simulink model "MainPlanevsRainCameras"  (R2020a)
settings: Solver=FixedStepDiscrete  StartTime=0.0  StopTime=20  RelTol=1e-3
model workspace (MAT data in the model file):
  firstWarning = 0
  originalScenarioChecksum = '4AECC2AEC181DD8EA774641D9E64C004'
undefined symbols (not defined in the file): driving
libraries: drivingscenarioandsensors x28
(part 2 of 6)

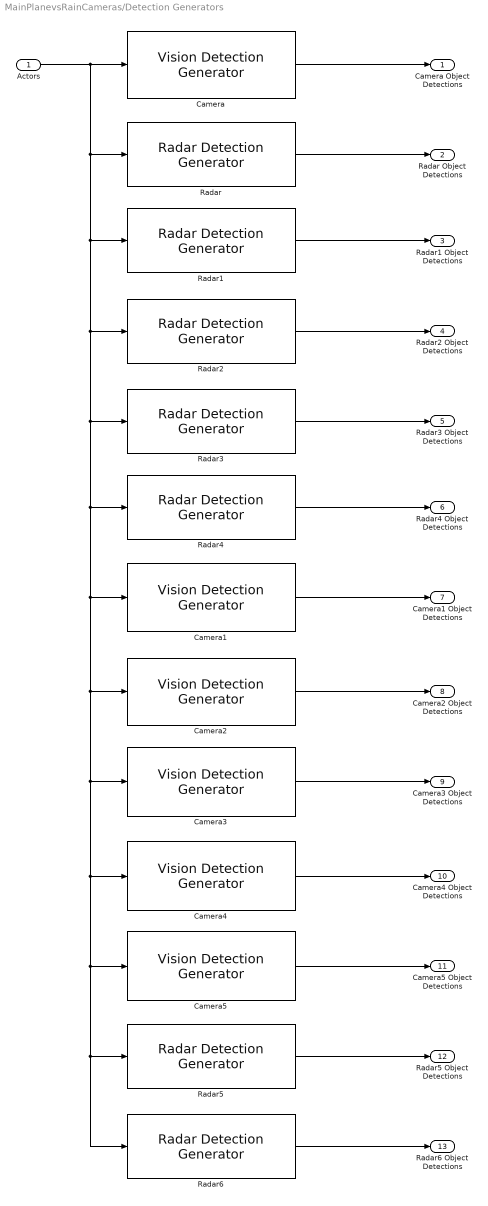
== system MainPlanevsRainCameras/Detection Generators ==
  Actors : Inport
  Camera : drivingscenarioandsensors/Vision Detection Generator  SensorIndex=1  DetectorOutput=Objects only  UpdateInterval=0.1  LaneUpdateInterval=0.1  SensorLocation=[1.9 0]  Height=1.1  Yaw=2.64254529406472  Pitch=1  Roll=0  BusNameSource=Auto  BusName=BusObjectDetections  BusName2Source=Auto  BusName2=BusLaneDetections  MaxNumDetectionsSource=Property  MaxNumDetections=50  MaxNumLanesSource=Property  MaxNumLanes=30  DetectionCoordinates=Ego Cartesian  SimulateUsing=Interpreted execution  MaxRange=11  BoundingBoxAccuracy=5  ProcessNoiseIntensity=5  MaxSpeed=50  MaxAllowedOcclusion=0.5  MinObjectImageSize=[15 15]  DetectionProbability=0.9  FalsePositivesPerImage=0.1  MinLaneImageSize=[20 3]  LaneBoundaryAccuracy=3  HasNoise=on  InitialSeedSource=Repeatable  InitialSeed=0  UsedSeed=0  ActorProfilesSource=MATLAB expression  ActorProfilesParameters=driving.internal.ActorProfilesParameters  ActorProfilesExpression=[struct('ActorID',1,'ClassID',1,'Length',4.7,'Width',1.8,'Height',1.4,'OriginOffset',[-1.35 0 0],'MeshVertices',[3.7 -0.9 1.4;3.7 0.9 1.4;-1 0.9 1.4;-1 -0.9 1.4;3.7 -0.9 0;3.7 0.9 0;-1 0.9 0;-1 -0.9 0],'MeshFaces',[6 2 1;1 5 6;8 4 3;3 7 8;6 7 3;3 2 6;5 1 4;4 8 5;4 1 2;2 3 4;7 6 5;5 8 7],'RCSPattern',[10 10;10 10],'RCSAzimuthAngles',[-180 180],'RCSElevationAngles',[-90 90]); struct('ActorID',2,'ClassID',1,'Length',4.7,'Width',1.8,'Height',1.4,'OriginOffset',[-1.35 0 0],'MeshVertices',[3.7 -0.9 1.4;3.7 0.9 1.4;-1 0.9 1.4;-1 -0.9 1.4;3.7 -0.9 0;3.7 0.9 0;-1 0.9 0;-1 -0.9 0],'MeshFaces',[6 2 1;1 5 6;8 4 3;3 7 8;6 7 3;3 2 6;5 1 4;4 8 5;4 1 2;2 3 4;7 6 5;5 8 7],'RCSPattern',[10 10;10 10],'RCSAzimuthAngles',[-180 180],'RCSElevationAngles',[-90 90]); struct('ActorID',3,'ClassID',1,'Length',4.7,'Width',1.8,'Height',1.4,'OriginOffset',[-1.35 0 0],'MeshVertices',[3.7 -0.9 1.4;3.7 0.9 1.4;-1 0.9 1.4;-1 -0.9 1.4;3.7 -0.9 0;3.7 0.9 0;-1 0.9 0;-1 -0.9 0],'MeshFaces',[6 2 1;1 5 6;8 4 3;3 7 8;6 7 3;3 2 6;5 1 4;4 8 5;4 1 2;2 3 4;7 6 5;5 8 7],'RCSPattern',[10 10;10 10],'RCSAzimuthAngles',[-180 180],'RCSElevationAngles',[-90 90]); struct('ActorID',4,'ClassID',1,'Length',4.7,'Width',1.8,'Height',1.4,'OriginOffset',[-1.35 0 0],'MeshVertices',[3.7 -0.9 1.4;3.7 0.9 1.4;-1 0.9 1.4;-1 -0.9 1.4;3.7 -0.9 0;3.7 0.9 0;-1 0.9 0;-1 -0.9 0],'MeshFaces',[6 2 1;1 5 6;8 4 3;3 7 8;6 7 3;3 2 6;5 1 4;4 8 5;4 1 2;2 3 4;7 6 5;5 8 7],'RCSPattern',[10 10;10 10],'RCSAzimuthAngles',[-180 180],'RCSElevationAngles',[-90 90]); struct('ActorID',5,'ClassID',1,'Length',4.7,'Width',1.8,'Height',1.4,'OriginOffset',[-1.35 0 0],'MeshVertices',[3.7 -0.9 1.4;3.7 0.9 1.4;-1 0.9 1.4;-1 -0.9 1.4;3.7 -0.9 0;3.7 0.9 0;-1 0.9 0;-1 -0.9 0],'MeshFaces',[6 2 1;1 5 6;8 4 3;3 7 8;6 7 3;3 2 6;5 1 4;4 8 5;4 1 2;2 3 4;7 6 5;5 8 7],'RCSPattern',[10 10;10 10],'RCSAzimuthAngles',[-180 180],'RCSElevationAngles',[-90 90]); struct('ActorID',6,'ClassID',4,'Length',0.24,'Width',0.45,'Height',1.7,'OriginOffset',[0 0 0],'MeshVertices',[0.12 -0.225 1.7;0.12 0.225 1.7;-0.12 0.225 1.7;-0.12 -0.225 1.7;0.12 -0.225 -1.11022302462516e-16;0.12 0.225 -1.11022302462516e-16;-0.12 0.225 -1.11022302462516e-16;-0.12 -0.225 -1.11022302462516e-16],'MeshFaces',[6 2 1;1 5 6;8 4 3;3 7 8;6 7 3;3 2 6;5 1 4;4 8 5;4 1 2;2 3 4;7 6 5;5 8 7],'RCSPattern',[-8 -8;-8 -8],'RCSAzimuthAngles',[-180 180],'RCSElevationAngles',[-90 90]); struct('ActorID',7,'ClassID',4,'Length',0.24,'Width',0.45,'Height',1.7,'OriginOffset',[0 0 0],'MeshVertices',[0.12 -0.225 1.7;0.12 0.225 1.7;-0.12 0.225 1.7;-0.12 -0.225 1.7;0.12 -0.225 -1.11022302462516e-16;0.12 0.225 -1.11022302462516e-16;-0.12 0.225 -1.11022302462516e-16;-0.12 -0.225 -1.11022302462516e-16],'MeshFaces',[6 2 1;1 5 6;8 4 3;3 7 8;6 7 3;3 2 6;5 1 4;4 8 5;4 1 2;2 3 4;7 6 5;5 8 7],'RCSPattern',[-8 -8;-8 -8],'RCSAzimuthAngles',[-180 180],'RCSElevationAngles',[-90 90]); struct('ActorID',8,'ClassID',4,'Length',0.24,'Width',0.45,'Height',1.7,'OriginOffset',[0 0 0],'MeshVertices',[0.12 -0.225 1.7;0.12 0.225 1.7;-0.12 0.225 1.7;-0.12 -0.225 1.7;0.12 -0.225 -1.11022302462516e-16;0.12 0.225 -1.11022302462516e-16;-0.12 0.225 -1.11022302462516e-16;-0.12 -0.225 -1.11022302462516e-16],'MeshFaces',[6 2 1;1 5 6;8 4 3;3 7 8;6 7 3;3 2 6;5 1 4;4 8 5;4 1 2;2 3 4;7 6 5;5 8 7],'RCSPattern',[-8 -8;-8 -8],'RCSAzimuthAngles',[-180 180],'RCSElevationAngles',[-90 90]); struct('ActorID',9,'ClassID',4,'Length',0.24,'Width',0.45,'Height',1.7,'OriginOffset',[0 0 0],'MeshVertices',[0.12 -0.225 1.7;0.12 0.225 1.7;-0.12 0.225 1.7;-0.12 -0.225 1.7;0.12 -0.225 -1.11022302462516e-16;0.12 0.225 -1.11022302462516e-16;-0.12 0.225 -1.11022302462516e-16;-0.12 -0.225 -1.11022302462516e-16],'MeshFaces',[6 2 1;1 5 6;8 4 3;3 7 8;6 7 3;3 2 6;5 1 4;4 8 5;4 1 2;2 3 4;7 6 5;5 8 7],'RCSPattern',[-8 -8;-8 -8],'RCSAzimuthAngles',[-180 180],'RCSElevationAngles',[-90 90]); struct('ActorID',10,'ClassID',4,'Length',0.24,'Width',0.45,'Height',1.7,'OriginOffset',[0 0 0],'MeshVertices',[0.12 -0.225 1.7;0.12 0.225 1.7;-0.12 0.225 1.7;-0.12 -0.225 1.7;0.12 -0.225 -1.11022302462516e-16;0.12 0.225 -1.11022302462516e-16;-0.12 0.225 -1.11022302462516e-16;-0.12 -0.225 -1.11022302462516e-16],'MeshFaces',[6 2 1;1 5 6;8 4 3;3 7 8;6 7 3;3 2 6;5 1 4;4 8 5;4 1 2;2 3 4;7 6 5;5 8 7],'RCSPattern',[-8 -8;-8 -8],'RCSAzimuthAngles',[-180 180],'RCSElevationAngles',[-90 90]); struct('ActorID',11,'ClassID',4,'Length',0.24,'Width',0.45,'Height',1.7,'OriginOffset',[0 0 0],'MeshVertices',[0.12 -0.225 1.7;0.12 0.225 1.7;-0.12 0.225 1.7;-0.12 -0.225 1.7;0.12 -0.225 -1.11022302462516e-16;0.12 0.225 -1.11022302462516e-16;-0.12 0.225 -1.11022302462516e-16;-0.12 -0.225 -1.11022302462516e-16],'MeshFaces',[6 2 1;1 5 6;8 4 3;3 7 8;6 7 3;3 2 6;5 1 4;4 8 5;4 1 2;2 3 4;7 6 5;5 8 7],'RCSPattern',[-8 -8;-8 -8],'RCSAzimuthAngles',[-180 180],'RCSElevationAngles',[-90 90]); struct('ActorID',12,'ClassID',4,'Length',0.24,'Width',0.45,'Height',1.7,'OriginOffset',[0 0 0],'MeshVertices',[0.12 -0.225 1.7;0.12 0.225 1.7;-0.12 0.225 1.7;-0.12 -0.225 1.7;0.12 -0.225 -1.11022302462516e-16;0.12 0.225 -1.11022302462516e-16;-0.12 0.225 -1.11022302462516e-16;-0.12 -0.225 -1.11022302462516e-16],'MeshFaces',[6 2 1;1 5 6;8 4 3;3 7 8;6 7 3;3 2 6;5 1 4;4 8 5;4 1 2;2 3 4;7 6 5;5 8 7],'RCSPattern',[-8 -8;-8 -8],'RCSAzimuthAngles',[-180 180],'RCSElevationAngles',[-90 90]); struct('ActorID',13,'ClassID',4,'Length',0.24,'Width',0.45,'Height',1.7,'OriginOffset',[0 0 0],'MeshVertices',[0.12 -0.225 1.7;0.12 0.225 1.7;-0.12 0.225 1.7;-0.12 -0.225 1.7;0.12 -0.225 -1.11022302462516e-16;0.12 0.225 -1.11022302462516e-16;-0.12 0.225 -1.11022302462516e-16;-0.12 -0.225 -1.11022302462516e-16],'MeshFaces',[6 2 1;1 5 6;8 4 3;3 7 8;6 7 3;3 2 6;5 1 4;4 8 5;4 1 2;2 3 4;7 6 5;5 8 7],'RCSPattern',[-8 -8;-8 -8],'RCSAzimuthAngles',[-180 180],'RCSElevationAngles',[-90 90]); struct('ActorID',14,'ClassID',4,'Length',0.24,'Width',0.45,'Height',1.7,'OriginOffset',[0 0 0],'MeshVertices',[0.12 -0.225 1.7;0.12 0.225 1.7;-0.12 0.225 1.7;-0.12 -0.225 1.7;0.12 -0.225 -1.11022302462516e-16;0.12 0.225 -1.11022302462516e-16;-0.12 0.225 -1.11022302462516e-16;-0.12 -0.225 -1.11022302462516e-16],'MeshFaces',[6 2 1;1 5 6;8 4 3;3 7 8;6 7 3;3 2 6;5 1 4;4 8 5;4 1 2;2 3 4;7 6 5;5 8 7],'RCSPattern',[-8 -8;-8 -8],'RCSAzimuthAngles',[-180 180],'RCSElevationAngles',[-90 90]); struct('ActorID',15,'ClassID',4,'Length',0.24,'Width',0.45,'Height',1.7,'OriginOffset',[0 0 0],'MeshVertices',[0.12 -0.225 1.7;0.12 0.225 1.7;-0.12 0.225 1.7;-0.12 -0.225 1.7;0.12 -0.225 -1.11022302462516e-16;0.12 0.225 -1.11022302462516e-16;-0.12 0.225 -1.11022302462516e-16;-0.12 -0.225 -1.11022302462516e-16],'MeshFaces',[6 2 1;1 5 6;8 4 3;3 7 8;6 7 3;3 2 6;5 1 4;4 8 5;4 1 2;2 3 4;7 6 5;5 8 7],'RCSPattern',[-8 -8;-8 -8],'RCSAzimuthAngles',[-180 180],'RCSElevationAngles',[-90 90]); struct('ActorID',16,'ClassID',4,'Length',0.24,'Width',0.45,'Height',1.7,'OriginOffset',[0 0 0],'MeshVertices',[0.12 -0.225 1.7;0.12 0.225 1.7;-0.12 0.225 1.7;-0.12 -0.225 1.7;0.12 -0.225 -1.11022302462516e-16;0.12 0.225 -1.11022302462516e-16;-0.12 0.225 -1.11022302462516e-16;-0.12 -0.225 -1.11022302462516e-16],'MeshFaces',[6 2 1;1 5 6;8 4 3;3 7 8;6 7 3;3 2 6;5 1 4;4 8 5;4 1 2;2 3 4;7 6 5;5 8 7],'RCSPattern',[-8 -8;-8 -8],'RCSAzimuthAngles',[-180 180],'RCSElevationAngles',[-90 90]); struct('ActorID',17,'ClassID',4,'Length',0.24,'Width',0.45,'Height',1.7,'OriginOffset',[0 0 0],'MeshVertices',[0.12 -0.225 1.7;0.12 0.225 1.7;-0.12 0.225 1.7;-0.12 -0.225 1.7;0.12 -0.225 -1.11022302462516e-16;0.12 0.225 -1.11022302462516e-16;-0.12 0.225 -1.11022302462516e-16;-0.12 -0.225 -1.11022302462516e-16],'MeshFaces',[6 2 1;1 5 6;8 4 3;3 7 8;6 7 3;3 2 6;5 1 4;4 8 5;4 1 2;2 3 4;7 6 5;5 8 7],'RCSPattern',[-8 -8;-8 -8],'RCSAzimuthAngles',[-180 180],'RCSElevationAngles',[-90 90]); struct('ActorID',18,'ClassID',4,'Length',0.24,'Width',0.45,'Height',1.7,'OriginOffset',[0 0 0],'MeshVertices',[0.12 -0.225 1.7;0.12 0.225 1.7;-0.12 0.225 1.7;-0.12 -0.225 1.7;0.12 -0.225 -1.11022302462516e-16;0.12 0.225 -1.11022302462516e-16;-0.12 0.225 -1.11022302462516e-16;-0.12 -0.225 -1.11022302462516e-16],'MeshFaces',[6 2 1;1 5 6;8 4 3;3 7 8;6 7 3;3 2 6;5 1 4;4 8 5;4 1 2;2 3 4;7 6 5;5 8 7],'RCSPattern',[-8 -8;-8 -8],'RCSAzimuthAngles',[-180 180],'RCSElevationAngles',[-90 90]); struct('ActorID',19,'ClassID',4,'Length',0.24,'Width',0.45,'Height',1.7,'OriginOffset',[0 0 0],'MeshVertices',[0.12 -0.225 1.7;0.12 0.225 1.7;-0.12 0.225 1.7;-0.12 -0.225 1.7;0.12 -0.225 -1.11022302462516e-16;0.12 0.225 -1.11022302462516e-16;-0.12 0.225 -1.11022302462516e-16;-0.12 -0.225 -1.11022302462516e-16],'MeshFaces',[6 2 1;1 5 6;8 4 3;3 7 8;6 7 3;3 2 6;5 1 4;4 8 5;4 1 2;2 3 4;7 6 5;5 8 7],'RCSPattern',[-8 -8;-8 -8],'RCSAzimuthAngles',[-180 180],'RCSElevationAngles',[-90 90]); struct('ActorID',20,'ClassID',4,'Length',0.24,'Width',0.45,'Height',1.7,'OriginOffset',[0 0 0],'MeshVertices',[0.12 -0.225 1.7;0.12 0.225 1.7;-0.12 0.225 1.7;-0.12 -0.225 1.7;0.12 -0.225 -1.11022302462516e-16;0.12 0.225 -1.11022302462516e-16;-0.12 0.225 -1.11022302462516e-16;-0.12 -0.225 -1.11022302462516e-16],'MeshFaces',[6 2 1;1 5 6;8 4 3;3 7 8;6 7 3;3 2 6;5 1 4;4 8 5;4 1 2;2 3 4;7 6 5;5 8 7],'RCSPattern',[-8 -8;-8 -8],'RCSAzimuthAngles',[-180 180],'RCSElevationAngles',[-90 90]); struct('ActorID',21,'ClassID',4,'Length',0.24,'Width',0.45,'Height',1.7,'OriginOffset',[0 0 0],'MeshVertices',[0.12 -0.225 1.7;0.12 0.225 1.7;-0.12 0.225 1.7;-0.12 -0.225 1.7;0.12 -0.225 -1.11022302462516e-16;0.12 0.225 -1.11022302462516e-16;-0.12 0.225 -1.11022302462516e-16;-0.12 -0.225 -1.11022302462516e-16],'MeshFaces',[6 2 1;1 5 6;8 4 3;3 7 8;6 7 3;3 2 6;5 1 4;4 8 5;4 1 2;2 3 4;7 6 5;5 8 7],'RCSPattern',[-8 -8;-8 -8],'RCSAzimuthAngles',[-180 180],'RCSElevationAngles',[-90 90]); struct('ActorID',22,'ClassID',4,'Length',0.24,'Width',0.45,'Height',1.7,'OriginOffset',[0 0 0],'MeshVertices',[0.12 -0.225 1.7;0.12 0.225 1.7;-0.12 0.225 1.7;-0.12 -0.225 1.7;0.12 -0.225 -1.11022302462516e-16;0.12 0.225 -1.11022302462516e-16;-0.12 0.225 -1.11022302462516e-16;-0.12 -0.225 -1.11022302462516e-16],'MeshFaces',[6 2 1;1 5 6;8 4 3;3 7 8;6 7 3;3 2 6;5 1 4;4 8 5;4 1 2;2 3 4;7 6 5;5 8 7],'RCSPattern',[-8 -8;-8 -8],'RCSAzimuthAngles',[-180 180],'RCSElevationAngles',[-90 90]); struct('ActorID',23,'ClassID',4,'Length',0.24,'Width',0.45,'Height',1.7,'OriginOffset',[0 0 0],'MeshVertices',[0.12 -0.225 1.7;0.12 0.225 1.7;-0.12 0.225 1.7;-0.12 -0.225 1.7;0.12 -0.225 -1.11022302462516e-16;0.12 0.225 -1.11022302462516e-16;-0.12 0.225 -1.11022302462516e-16;-0.12 -0.225 -1.11022302462516e-16],'MeshFaces',[6 2 1;1 5 6;8 4 3;3 7 8;6 7 3;3 2 6;5 1 4;4 8 5;4 1 2;2 3 4;7 6 5;5 8 7],'RCSPattern',[-8 -8;-8 -8],'RCSAzimuthAngles',[-180 180],'RCSElevationAngles',[-90 90]); struct('ActorID',24,'ClassID',4,'Length',0.24,'Width',0.45,'Height',1.7,'OriginOffset',[0 0 0],'MeshVertices',[0.12 -0.225 1.7;0.12 0.225 1.7;-0.12 0.225 1.7;-0.12 -0.225 1.7;0.12 -0.225 -1.11022302462516e-16;0.12 0.225 -1.11022302462516e-16;-0.12 0.225 -1.11022302462516e-16;-0.12 -0.225 -1.11022302462516e-16],'MeshFaces',[6 2 1;1 5 6;8 4 3;3 7 8;6 7 3;3 2 6;5 1 4;4 8 5;4 1 2;2 3 4;7 6 5;5 8 7],'RCSPattern',[-8 -8;-8 -8],'RCSAzimuthAngles',[-180 180],'RCSElevationAngles',[-90 90]); struct('ActorID',25,'ClassID',4,'Length',0.24,'Width',0.45,'Height',1.7,'OriginOffset',[0 0 0],'MeshVertices',[0.12 -0.225 1.7;0.12 0.225 1.7;-0.12 0.225 1.7;-0.12 -0.225 1.7;0.12 -0.225 -1.11022302462516e-16;0.12 0.225 -1.11022302462516e-16;-0.12 0.225 -1.11022302462516e-16;-0.12 -0.225 -1.11022302462516e-16],'MeshFaces',[6 2 1;1 5 6;8 4 3;3 7 8;6 7 3;3 2 6;5 1 4;4 8 5;4 1 2;2 3 4;7 6 5;5 8 7],'RCSPattern',[-8 -8;-8 -8],'RCSAzimuthAngles',[-180 180],'RCSElevationAngles',[-90 90]); struct('ActorID',26,'ClassID',4,'Length',0.24,'Width',0.45,'Height',1.7,'OriginOffset',[0 0 0],'MeshVertices',[0.12 -0.225 1.7;0.12 0.225 1.7;-0.12 0.225 1.7;-0.12 -0.225 1.7;0.12 -0.225 -1.11022302462516e-16;0.12 0.225 -1.11022302462516e-16;-0.12 0.225 -1.11022302462516e-16;-0.12 -0.225 -1.11022302462516e-16],'MeshFaces',[6 2 1;1 5 6;8 4 3;3 7 8;6 7 3;3 2 6;5 1 4;4 8 5;4 1 2;2 3 4;7 6 5;5 8 7],'RCSPattern',[-8 -8;-8 -8],'RCSAzimuthAngles',[-180 180],'RCSElevationAngles',[-90 90]); struct('ActorID',27,'ClassID',4,'Length',0.24,'Width',0.45,'Height',1.7,'OriginOffset',[0 0 0],'MeshVertices',[0.12 -0.225 1.7;0.12 0.225 1.7;-0.12 0.225 1.7;-0.12 -0.225 1.7;0.12 -0.225 -1.11022302462516e-16;0.12 0.225 -1.11022302462516e-16;-0.12 0.225 -1.11022302462516e-16;-0.12 -0.225 -1.11022302462516e-16],'MeshFaces',[6 2 1;1 5 6;8 4 3;3 7 8;6 7 3;3 2 6;5 1 4;4 8 5;4 1 2;2 3 4;7 6 5;5 8 7],'RCSPattern',[-8 -8;-8 -8],'RCSAzimuthAngles',[-180 180],'RCSElevationAngles',[-90 90]); struct('ActorID',28,'ClassID',3,'Length',1.7,'Width',0.45,'Height',1.7,'OriginOffset',[0 0 0],'MeshVertices',[0.85 -0.225 1.7;0.85 0.225 1.7;-0.85 0.225 1.7;-0.85 -0.225 1.7;0.85 -0.225 -1.11022302462516e-16;0.85 0.225 -1.11022302462516e-16;-0.85 0.225 -1.11022302462516e-16;-0.85 -0.225 -1.11022302462516e-16],'MeshFaces',[6 2 1;1 5 6;8 4 3;3 7 8;6 7 3;3 2 6;5 1 4;4 8 5;4 1 2;2 3 4;7 6 5;5 8 7],'RCSPattern',[10 10;10 10],'RCSAzimuthAngles',[-180 180],'RCSElevationAngles',[-90 90]); struct('ActorID',29,'ClassID',4,'Length',0.24,'Width',0.45,'Height',1.7,'OriginOffset',[0 0 0],'MeshVertices',[0.12 -0.225 1.7;0.12 0.225 1.7;-0.12 0.225 1.7;-0.12 -0.225 1.7;0.12 -0.225 -1.11022302462516e-16;0.12 0.225 -1.11022302462516e-16;-0.12 0.225 -1.11022302462516e-16;-0.12 -0.225 -1.11022302462516e-16],'MeshFaces',[6 2 1;1 5 6;8 4 3;3 7 8;6 7 3;3 2 6;5 1 4;4 8 5;4 1 2;2 3 4;7 6 5;5 8 7],'RCSPattern',[-8 -8;-8 -8],'RCSAzimuthAngles',[-180 180],'RCSElevationAngles',[-90 90])]  Intrinsics=driving.internal.cameraIntrinsics('FocalLength',[800 799.999999999999],'PrincipalPoint',[320 240],'ImageSize',[480 640],'RadialDistortion',[0 0],'TangentialDistortion',[0 0],'Skew',0)
  Camera1 : drivingscenarioandsensors/Vision Detection Generator  SensorIndex=7  DetectorOutput=Objects only  UpdateInterval=0.1  LaneUpdateInterval=0.1  SensorLocation=[0 0.9]  Height=1.1  Yaw=90  Pitch=1  Roll=0  BusNameSource=Auto  BusName=BusObjectDetections  BusName2Source=Auto  BusName2=BusLaneDetections  MaxNumDetectionsSource=Property  MaxNumDetections=50  MaxNumLanesSource=Property  MaxNumLanes=30  DetectionCoordinates=Ego Cartesian  SimulateUsing=Interpreted execution  MaxRange=10  BoundingBoxAccuracy=5  ProcessNoiseIntensity=5  MaxSpeed=50  MaxAllowedOcclusion=0.5  MinObjectImageSize=[15 15]  DetectionProbability=0.2  FalsePositivesPerImage=0.1  MinLaneImageSize=[20 3]  LaneBoundaryAccuracy=3  HasNoise=on  InitialSeedSource=Repeatable  InitialSeed=0  UsedSeed=0  ActorProfilesSource=MATLAB expression  ActorProfilesParameters=driving.internal.ActorProfilesParameters  ActorProfilesExpression=[struct('ActorID',1,'ClassID',1,'Length',4.7,'Width',1.8,'Height',1.4,'OriginOffset',[-1.35 0 0],'MeshVertices',[3.7 -0.9 1.4;3.7 0.9 1.4;-1 0.9 1.4;-1 -0.9 1.4;3.7 -0.9 0;3.7 0.9 0;-1 0.9 0;-1 -0.9 0],'MeshFaces',[6 2 1;1 5 6;8 4 3;3 7 8;6 7 3;3 2 6;5 1 4;4 8 5;4 1 2;2 3 4;7 6 5;5 8 7],'RCSPattern',[10 10;10 10],'RCSAzimuthAngles',[-180 180],'RCSElevationAngles',[-90 90]); struct('ActorID',2,'ClassID',1,'Length',4.7,'Width',1.8,'Height',1.4,'OriginOffset',[-1.35 0 0],'MeshVertices',[3.7 -0.9 1.4;3.7 0.9 1.4;-1 0.9 1.4;-1 -0.9 1.4;3.7 -0.9 0;3.7 0.9 0;-1 0.9 0;-1 -0.9 0],'MeshFaces',[6 2 1;1 5 6;8 4 3;3 7 8;6 7 3;3 2 6;5 1 4;4 8 5;4 1 2;2 3 4;7 6 5;5 8 7],'RCSPattern',[10 10;10 10],'RCSAzimuthAngles',[-180 180],'RCSElevationAngles',[-90 90]); struct('ActorID',3,'ClassID',1,'Length',4.7,'Width',1.8,'Height',1.4,'OriginOffset',[-1.35 0 0],'MeshVertices',[3.7 -0.9 1.4;3.7 0.9 1.4;-1 0.9 1.4;-1 -0.9 1.4;3.7 -0.9 0;3.7 0.9 0;-1 0.9 0;-1 -0.9 0],'MeshFaces',[6 2 1;1 5 6;8 4 3;3 7 8;6 7 3;3 2 6;5 1 4;4 8 5;4 1 2;2 3 4;7 6 5;5 8 7],'RCSPattern',[10 10;10 10],'RCSAzimuthAngles',[-180 180],'RCSElevationAngles',[-90 90]); struct('ActorID',4,'ClassID',1,'Length',4.7,'Width',1.8,'Height',1.4,'OriginOffset',[-1.35 0 0],'MeshVertices',[3.7 -0.9 1.4;3.7 0.9 1.4;-1 0.9 1.4;-1 -0.9 1.4;3.7 -0.9 0;3.7 0.9 0;-1 0.9 0;-1 -0.9 0],'MeshFaces',[6 2 1;1 5 6;8 4 3;3 7 8;6 7 3;3 2 6;5 1 4;4 8 5;4 1 2;2 3 4;7 6 5;5 8 7],'RCSPattern',[10 10;10 10],'RCSAzimuthAngles',[-180 180],'RCSElevationAngles',[-90 90]); struct('ActorID',5,'ClassID',1,'Length',4.7,'Width',1.8,'Height',1.4,'OriginOffset',[-1.35 0 0],'MeshVertices',[3.7 -0.9 1.4;3.7 0.9 1.4;-1 0.9 1.4;-1 -0.9 1.4;3.7 -0.9 0;3.7 0.9 0;-1 0.9 0;-1 -0.9 0],'MeshFaces',[6 2 1;1 5 6;8 4 3;3 7 8;6 7 3;3 2 6;5 1 4;4 8 5;4 1 2;2 3 4;7 6 5;5 8 7],'RCSPattern',[10 10;10 10],'RCSAzimuthAngles',[-180 180],'RCSElevationAngles',[-90 90]); struct('ActorID',6,'ClassID',4,'Length',0.24,'Width',0.45,'Height',1.7,'OriginOffset',[0 0 0],'MeshVertices',[0.12 -0.225 1.7;0.12 0.225 1.7;-0.12 0.225 1.7;-0.12 -0.225 1.7;0.12 -0.225 -1.11022302462516e-16;0.12 0.225 -1.11022302462516e-16;-0.12 0.225 -1.11022302462516e-16;-0.12 -0.225 -1.11022302462516e-16],'MeshFaces',[6 2 1;1 5 6;8 4 3;3 7 8;6 7 3;3 2 6;5 1 4;4 8 5;4 1 2;2 3 4;7 6 5;5 8 7],'RCSPattern',[-8 -8;-8 -8],'RCSAzimuthAngles',[-180 180],'RCSElevationAngles',[-90 90]); struct('ActorID',7,'ClassID',4,'Length',0.24,'Width',0.45,'Height',1.7,'OriginOffset',[0 0 0],'MeshVertices',[0.12 -0.225 1.7;0.12 0.225 1.7;-0.12 0.225 1.7;-0.12 -0.225 1.7;0.12 -0.225 -1.11022302462516e-16;0.12 0.225 -1.11022302462516e-16;-0.12 0.225 -1.11022302462516e-16;-0.12 -0.225 -1.11022302462516e-16],'MeshFaces',[6 2 1;1 5 6;8 4 3;3 7 8;6 7 3;3 2 6;5 1 4;4 8 5;4 1 2;2 3 4;7 6 5;5 8 7],'RCSPattern',[-8 -8;-8 -8],'RCSAzimuthAngles',[-180 180],'RCSElevationAngles',[-90 90]); struct('ActorID',8,'ClassID',4,'Length',0.24,'Width',0.45,'Height',1.7,'OriginOffset',[0 0 0],'MeshVertices',[0.12 -0.225 1.7;0.12 0.225 1.7;-0.12 0.225 1.7;-0.12 -0.225 1.7;0.12 -0.225 -1.11022302462516e-16;0.12 0.225 -1.11022302462516e-16;-0.12 0.225 -1.11022302462516e-16;-0.12 -0.225 -1.11022302462516e-16],'MeshFaces',[6 2 1;1 5 6;8 4 3;3 7 8;6 7 3;3 2 6;5 1 4;4 8 5;4 1 2;2 3 4;7 6 5;5 8 7],'RCSPattern',[-8 -8;-8 -8],'RCSAzimuthAngles',[-180 180],'RCSElevationAngles',[-90 90]); struct('ActorID',9,'ClassID',4,'Length',0.24,'Width',0.45,'Height',1.7,'OriginOffset',[0 0 0],'MeshVertices',[0.12 -0.225 1.7;0.12 0.225 1.7;-0.12 0.225 1.7;-0.12 -0.225 1.7;0.12 -0.225 -1.11022302462516e-16;0.12 0.225 -1.11022302462516e-16;-0.12 0.225 -1.11022302462516e-16;-0.12 -0.225 -1.11022302462516e-16],'MeshFaces',[6 2 1;1 5 6;8 4 3;3 7 8;6 7 3;3 2 6;5 1 4;4 8 5;4 1 2;2 3 4;7 6 5;5 8 7],'RCSPattern',[-8 -8;-8 -8],'RCSAzimuthAngles',[-180 180],'RCSElevationAngles',[-90 90]); struct('ActorID',10,'ClassID',4,'Length',0.24,'Width',0.45,'Height',1.7,'OriginOffset',[0 0 0],'MeshVertices',[0.12 -0.225 1.7;0.12 0.225 1.7;-0.12 0.225 1.7;-0.12 -0.225 1.7;0.12 -0.225 -1.11022302462516e-16;0.12 0.225 -1.11022302462516e-16;-0.12 0.225 -1.11022302462516e-16;-0.12 -0.225 -1.11022302462516e-16],'MeshFaces',[6 2 1;1 5 6;8 4 3;3 7 8;6 7 3;3 2 6;5 1 4;4 8 5;4 1 2;2 3 4;7 6 5;5 8 7],'RCSPattern',[-8 -8;-8 -8],'RCSAzimuthAngles',[-180 180],'RCSElevationAngles',[-90 90]); struct('ActorID',11,'ClassID',4,'Length',0.24,'Width',0.45,'Height',1.7,'OriginOffset',[0 0 0],'MeshVertices',[0.12 -0.225 1.7;0.12 0.225 1.7;-0.12 0.225 1.7;-0.12 -0.225 1.7;0.12 -0.225 -1.11022302462516e-16;0.12 0.225 -1.11022302462516e-16;-0.12 0.225 -1.11022302462516e-16;-0.12 -0.225 -1.11022302462516e-16],'MeshFaces',[6 2 1;1 5 6;8 4 3;3 7 8;6 7 3;3 2 6;5 1 4;4 8 5;4 1 2;2 3 4;7 6 5;5 8 7],'RCSPattern',[-8 -8;-8 -8],'RCSAzimuthAngles',[-180 180],'RCSElevationAngles',[-90 90]); struct('ActorID',12,'ClassID',4,'Length',0.24,'Width',0.45,'Height',1.7,'OriginOffset',[0 0 0],'MeshVertices',[0.12 -0.225 1.7;0.12 0.225 1.7;-0.12 0.225 1.7;-0.12 -0.225 1.7;0.12 -0.225 -1.11022302462516e-16;0.12 0.225 -1.11022302462516e-16;-0.12 0.225 -1.11022302462516e-16;-0.12 -0.225 -1.11022302462516e-16],'MeshFaces',[6 2 1;1 5 6;8 4 3;3 7 8;6 7 3;3 2 6;5 1 4;4 8 5;4 1 2;2 3 4;7 6 5;5 8 7],'RCSPattern',[-8 -8;-8 -8],'RCSAzimuthAngles',[-180 180],'RCSElevationAngles',[-90 90]); struct('ActorID',13,'ClassID',4,'Length',0.24,'Width',0.45,'Height',1.7,'OriginOffset',[0 0 0],'MeshVertices',[0.12 -0.225 1.7;0.12 0.225 1.7;-0.12 0.225 1.7;-0.12 -0.225 1.7;0.12 -0.225 -1.11022302462516e-16;0.12 0.225 -1.11022302462516e-16;-0.12 0.225 -1.11022302462516e-16;-0.12 -0.225 -1.11022302462516e-16],'MeshFaces',[6 2 1;1 5 6;8 4 3;3 7 8;6 7 3;3 2 6;5 1 4;4 8 5;4 1 2;2 3 4;7 6 5;5 8 7],'RCSPattern',[-8 -8;-8 -8],'RCSAzimuthAngles',[-180 180],'RCSElevationAngles',[-90 90]); struct('ActorID',14,'ClassID',4,'Length',0.24,'Width',0.45,'Height',1.7,'OriginOffset',[0 0 0],'MeshVertices',[0.12 -0.225 1.7;0.12 0.225 1.7;-0.12 0.225 1.7;-0.12 -0.225 1.7;0.12 -0.225 -1.11022302462516e-16;0.12 0.225 -1.11022302462516e-16;-0.12 0.225 -1.11022302462516e-16;-0.12 -0.225 -1.11022302462516e-16],'MeshFaces',[6 2 1;1 5 6;8 4 3;3 7 8;6 7 3;3 2 6;5 1 4;4 8 5;4 1 2;2 3 4;7 6 5;5 8 7],'RCSPattern',[-8 -8;-8 -8],'RCSAzimuthAngles',[-180 180],'RCSElevationAngles',[-90 90]); struct('ActorID',15,'ClassID',4,'Length',0.24,'Width',0.45,'Height',1.7,'OriginOffset',[0 0 0],'MeshVertices',[0.12 -0.225 1.7;0.12 0.225 1.7;-0.12 0.225 1.7;-0.12 -0.225 1.7;0.12 -0.225 -1.11022302462516e-16;0.12 0.225 -1.11022302462516e-16;-0.12 0.225 -1.11022302462516e-16;-0.12 -0.225 -1.11022302462516e-16],'MeshFaces',[6 2 1;1 5 6;8 4 3;3 7 8;6 7 3;3 2 6;5 1 4;4 8 5;4 1 2;2 3 4;7 6 5;5 8 7],'RCSPattern',[-8 -8;-8 -8],'RCSAzimuthAngles',[-180 180],'RCSElevationAngles',[-90 90]); struct('ActorID',16,'ClassID',4,'Length',0.24,'Width',0.45,'Height',1.7,'OriginOffset',[0 0 0],'MeshVertices',[0.12 -0.225 1.7;0.12 0.225 1.7;-0.12 0.225 1.7;-0.12 -0.225 1.7;0.12 -0.225 -1.11022302462516e-16;0.12 0.225 -1.11022302462516e-16;-0.12 0.225 -1.11022302462516e-16;-0.12 -0.225 -1.11022302462516e-16],'MeshFaces',[6 2 1;1 5 6;8 4 3;3 7 8;6 7 3;3 2 6;5 1 4;4 8 5;4 1 2;2 3 4;7 6 5;5 8 7],'RCSPattern',[-8 -8;-8 -8],'RCSAzimuthAngles',[-180 180],'RCSElevationAngles',[-90 90]); struct('ActorID',17,'ClassID',4,'Length',0.24,'Width',0.45,'Height',1.7,'OriginOffset',[0 0 0],'MeshVertices',[0.12 -0.225 1.7;0.12 0.225 1.7;-0.12 0.225 1.7;-0.12 -0.225 1.7;0.12 -0.225 -1.11022302462516e-16;0.12 0.225 -1.11022302462516e-16;-0.12 0.225 -1.11022302462516e-16;-0.12 -0.225 -1.11022302462516e-16],'MeshFaces',[6 2 1;1 5 6;8 4 3;3 7 8;6 7 3;3 2 6;5 1 4;4 8 5;4 1 2;2 3 4;7 6 5;5 8 7],'RCSPattern',[-8 -8;-8 -8],'RCSAzimuthAngles',[-180 180],'RCSElevationAngles',[-90 90]); struct('ActorID',18,'ClassID',4,'Length',0.24,'Width',0.45,'Height',1.7,'OriginOffset',[0 0 0],'MeshVertices',[0.12 -0.225 1.7;0.12 0.225 1.7;-0.12 0.225 1.7;-0.12 -0.225 1.7;0.12 -0.225 -1.11022302462516e-16;0.12 0.225 -1.11022302462516e-16;-0.12 0.225 -1.11022302462516e-16;-0.12 -0.225 -1.11022302462516e-16],'MeshFaces',[6 2 1;1 5 6;8 4 3;3 7 8;6 7 3;3 2 6;5 1 4;4 8 5;4 1 2;2 3 4;7 6 5;5 8 7],'RCSPattern',[-8 -8;-8 -8],'RCSAzimuthAngles',[-180 180],'RCSElevationAngles',[-90 90]); struct('ActorID',19,'ClassID',4,'Length',0.24,'Width',0.45,'Height',1.7,'OriginOffset',[0 0 0],'MeshVertices',[0.12 -0.225 1.7;0.12 0.225 1.7;-0.12 0.225 1.7;-0.12 -0.225 1.7;0.12 -0.225 -1.11022302462516e-16;0.12 0.225 -1.11022302462516e-16;-0.12 0.225 -1.11022302462516e-16;-0.12 -0.225 -1.11022302462516e-16],'MeshFaces',[6 2 1;1 5 6;8 4 3;3 7 8;6 7 3;3 2 6;5 1 4;4 8 5;4 1 2;2 3 4;7 6 5;5 8 7],'RCSPattern',[-8 -8;-8 -8],'RCSAzimuthAngles',[-180 180],'RCSElevationAngles',[-90 90]); struct('ActorID',20,'ClassID',4,'Length',0.24,'Width',0.45,'Height',1.7,'OriginOffset',[0 0 0],'MeshVertices',[0.12 -0.225 1.7;0.12 0.225 1.7;-0.12 0.225 1.7;-0.12 -0.225 1.7;0.12 -0.225 -1.11022302462516e-16;0.12 0.225 -1.11022302462516e-16;-0.12 0.225 -1.11022302462516e-16;-0.12 -0.225 -1.11022302462516e-16],'MeshFaces',[6 2 1;1 5 6;8 4 3;3 7 8;6 7 3;3 2 6;5 1 4;4 8 5;4 1 2;2 3 4;7 6 5;5 8 7],'RCSPattern',[-8 -8;-8 -8],'RCSAzimuthAngles',[-180 180],'RCSElevationAngles',[-90 90]); struct('ActorID',21,'ClassID',4,'Length',0.24,'Width',0.45,'Height',1.7,'OriginOffset',[0 0 0],'MeshVertices',[0.12 -0.225 1.7;0.12 0.225 1.7;-0.12 0.225 1.7;-0.12 -0.225 1.7;0.12 -0.225 -1.11022302462516e-16;0.12 0.225 -1.11022302462516e-16;-0.12 0.225 -1.11022302462516e-16;-0.12 -0.225 -1.11022302462516e-16],'MeshFaces',[6 2 1;1 5 6;8 4 3;3 7 8;6 7 3;3 2 6;5 1 4;4 8 5;4 1 2;2 3 4;7 6 5;5 8 7],'RCSPattern',[-8 -8;-8 -8],'RCSAzimuthAngles',[-180 180],'RCSElevationAngles',[-90 90]); struct('ActorID',22,'ClassID',4,'Length',0.24,'Width',0.45,'Height',1.7,'OriginOffset',[0 0 0],'MeshVertices',[0.12 -0.225 1.7;0.12 0.225 1.7;-0.12 0.225 1.7;-0.12 -0.225 1.7;0.12 -0.225 -1.11022302462516e-16;0.12 0.225 -1.11022302462516e-16;-0.12 0.225 -1.11022302462516e-16;-0.12 -0.225 -1.11022302462516e-16],'MeshFaces',[6 2 1;1 5 6;8 4 3;3 7 8;6 7 3;3 2 6;5 1 4;4 8 5;4 1 2;2 3 4;7 6 5;5 8 7],'RCSPattern',[-8 -8;-8 -8],'RCSAzimuthAngles',[-180 180],'RCSElevationAngles',[-90 90]); struct('ActorID',23,'ClassID',4,'Length',0.24,'Width',0.45,'Height',1.7,'OriginOffset',[0 0 0],'MeshVertices',[0.12 -0.225 1.7;0.12 0.225 1.7;-0.12 0.225 1.7;-0.12 -0.225 1.7;0.12 -0.225 -1.11022302462516e-16;0.12 0.225 -1.11022302462516e-16;-0.12 0.225 -1.11022302462516e-16;-0.12 -0.225 -1.11022302462516e-16],'MeshFaces',[6 2 1;1 5 6;8 4 3;3 7 8;6 7 3;3 2 6;5 1 4;4 8 5;4 1 2;2 3 4;7 6 5;5 8 7],'RCSPattern',[-8 -8;-8 -8],'RCSAzimuthAngles',[-180 180],'RCSElevationAngles',[-90 90]); struct('ActorID',24,'ClassID',4,'Length',0.24,'Width',0.45,'Height',1.7,'OriginOffset',[0 0 0],'MeshVertices',[0.12 -0.225 1.7;0.12 0.225 1.7;-0.12 0.225 1.7;-0.12 -0.225 1.7;0.12 -0.225 -1.11022302462516e-16;0.12 0.225 -1.11022302462516e-16;-0.12 0.225 -1.11022302462516e-16;-0.12 -0.225 -1.11022302462516e-16],'MeshFaces',[6 2 1;1 5 6;8 4 3;3 7 8;6 7 3;3 2 6;5 1 4;4 8 5;4 1 2;2 3 4;7 6 5;5 8 7],'RCSPattern',[-8 -8;-8 -8],'RCSAzimuthAngles',[-180 180],'RCSElevationAngles',[-90 90]); struct('ActorID',25,'ClassID',4,'Length',0.24,'Width',0.45,'Height',1.7,'OriginOffset',[0 0 0],'MeshVertices',[0.12 -0.225 1.7;0.12 0.225 1.7;-0.12 0.225 1.7;-0.12 -0.225 1.7;0.12 -0.225 -1.11022302462516e-16;0.12 0.225 -1.11022302462516e-16;-0.12 0.225 -1.11022302462516e-16;-0.12 -0.225 -1.11022302462516e-16],'MeshFaces',[6 2 1;1 5 6;8 4 3;3 7 8;6 7 3;3 2 6;5 1 4;4 8 5;4 1 2;2 3 4;7 6 5;5 8 7],'RCSPattern',[-8 -8;-8 -8],'RCSAzimuthAngles',[-180 180],'RCSElevationAngles',[-90 90]); struct('ActorID',26,'ClassID',4,'Length',0.24,'Width',0.45,'Height',1.7,'OriginOffset',[0 0 0],'MeshVertices',[0.12 -0.225 1.7;0.12 0.225 1.7;-0.12 0.225 1.7;-0.12 -0.225 1.7;0.12 -0.225 -1.11022302462516e-16;0.12 0.225 -1.11022302462516e-16;-0.12 0.225 -1.11022302462516e-16;-0.12 -0.225 -1.11022302462516e-16],'MeshFaces',[6 2 1;1 5 6;8 4 3;3 7 8;6 7 3;3 2 6;5 1 4;4 8 5;4 1 2;2 3 4;7 6 5;5 8 7],'RCSPattern',[-8 -8;-8 -8],'RCSAzimuthAngles',[-180 180],'RCSElevationAngles',[-90 90]); struct('ActorID',27,'ClassID',4,'Length',0.24,'Width',0.45,'Height',1.7,'OriginOffset',[0 0 0],'MeshVertices',[0.12 -0.225 1.7;0.12 0.225 1.7;-0.12 0.225 1.7;-0.12 -0.225 1.7;0.12 -0.225 -1.11022302462516e-16;0.12 0.225 -1.11022302462516e-16;-0.12 0.225 -1.11022302462516e-16;-0.12 -0.225 -1.11022302462516e-16],'MeshFaces',[6 2 1;1 5 6;8 4 3;3 7 8;6 7 3;3 2 6;5 1 4;4 8 5;4 1 2;2 3 4;7 6 5;5 8 7],'RCSPattern',[-8 -8;-8 -8],'RCSAzimuthAngles',[-180 180],'RCSElevationAngles',[-90 90]); struct('ActorID',28,'ClassID',3,'Length',1.7,'Width',0.45,'Height',1.7,'OriginOffset',[0 0 0],'MeshVertices',[0.85 -0.225 1.7;0.85 0.225 1.7;-0.85 0.225 1.7;-0.85 -0.225 1.7;0.85 -0.225 -1.11022302462516e-16;0.85 0.225 -1.11022302462516e-16;-0.85 0.225 -1.11022302462516e-16;-0.85 -0.225 -1.11022302462516e-16],'MeshFaces',[6 2 1;1 5 6;8 4 3;3 7 8;6 7 3;3 2 6;5 1 4;4 8 5;4 1 2;2 3 4;7 6 5;5 8 7],'RCSPattern',[10 10;10 10],'RCSAzimuthAngles',[-180 180],'RCSElevationAngles',[-90 90]); struct('ActorID',29,'ClassID',4,'Length',0.24,'Width',0.45,'Height',1.7,'OriginOffset',[0 0 0],'MeshVertices',[0.12 -0.225 1.7;0.12 0.225 1.7;-0.12 0.225 1.7;-0.12 -0.225 1.7;0.12 -0.225 -1.11022302462516e-16;0.12 0.225 -1.11022302462516e-16;-0.12 0.225 -1.11022302462516e-16;-0.12 -0.225 -1.11022302462516e-16],'MeshFaces',[6 2 1;1 5 6;8 4 3;3 7 8;6 7 3;3 2 6;5 1 4;4 8 5;4 1 2;2 3 4;7 6 5;5 8 7],'RCSPattern',[-8 -8;-8 -8],'RCSAzimuthAngles',[-180 180],'RCSElevationAngles',[-90 90])]  Intrinsics=driving.internal.cameraIntrinsics('FocalLength',[320 320],'PrincipalPoint',[320 240],'ImageSize',[480 640],'RadialDistortion',[0 0],'TangentialDistortion',[0 0],'Skew',0)
  Camera2 : drivingscenarioandsensors/Vision Detection Generator  SensorIndex=8  DetectorOutput=Objects only  UpdateInterval=0.1  LaneUpdateInterval=0.1  SensorLocation=[0 -0.9]  Height=1.1  Yaw=-90  Pitch=1  Roll=0  BusNameSource=Auto  BusName=BusObjectDetections  BusName2Source=Auto  BusName2=BusLaneDetections  MaxNumDetectionsSource=Property  MaxNumDetections=50  MaxNumLanesSource=Property  MaxNumLanes=30  DetectionCoordinates=Ego Cartesian  SimulateUsing=Interpreted execution  MaxRange=10  BoundingBoxAccuracy=5  ProcessNoiseIntensity=2  MaxSpeed=50  MaxAllowedOcclusion=0.5  MinObjectImageSize=[15 15]  DetectionProbability=0.2  FalsePositivesPerImage=0.1  MinLaneImageSize=[20 3]  LaneBoundaryAccuracy=3  HasNoise=on  InitialSeedSource=Repeatable  InitialSeed=0  UsedSeed=0  ActorProfilesSource=MATLAB expression  ActorProfilesParameters=driving.internal.ActorProfilesParameters  ActorProfilesExpression=[struct('ActorID',1,'ClassID',1,'Length',4.7,'Width',1.8,'Height',1.4,'OriginOffset',[-1.35 0 0],'MeshVertices',[3.7 -0.9 1.4;3.7 0.9 1.4;-1 0.9 1.4;-1 -0.9 1.4;3.7 -0.9 0;3.7 0.9 0;-1 0.9 0;-1 -0.9 0],'MeshFaces',[6 2 1;1 5 6;8 4 3;3 7 8;6 7 3;3 2 6;5 1 4;4 8 5;4 1 2;2 3 4;7 6 5;5 8 7],'RCSPattern',[10 10;10 10],'RCSAzimuthAngles',[-180 180],'RCSElevationAngles',[-90 90]); struct('ActorID',2,'ClassID',1,'Length',4.7,'Width',1.8,'Height',1.4,'OriginOffset',[-1.35 0 0],'MeshVertices',[3.7 -0.9 1.4;3.7 0.9 1.4;-1 0.9 1.4;-1 -0.9 1.4;3.7 -0.9 0;3.7 0.9 0;-1 0.9 0;-1 -0.9 0],'MeshFaces',[6 2 1;1 5 6;8 4 3;3 7 8;6 7 3;3 2 6;5 1 4;4 8 5;4 1 2;2 3 4;7 6 5;5 8 7],'RCSPattern',[10 10;10 10],'RCSAzimuthAngles',[-180 180],'RCSElevationAngles',[-90 90]); struct('ActorID',3,'ClassID',1,'Length',4.7,'Width',1.8,'Height',1.4,'OriginOffset',[-1.35 0 0],'MeshVertices',[3.7 -0.9 1.4;3.7 0.9 1.4;-1 0.9 1.4;-1 -0.9 1.4;3.7 -0.9 0;3.7 0.9 0;-1 0.9 0;-1 -0.9 0],'MeshFaces',[6 2 1;1 5 6;8 4 3;3 7 8;6 7 3;3 2 6;5 1 4;4 8 5;4 1 2;2 3 4;7 6 5;5 8 7],'RCSPattern',[10 10;10 10],'RCSAzimuthAngles',[-180 180],'RCSElevationAngles',[-90 90]); struct('ActorID',4,'ClassID',1,'Length',4.7,'Width',1.8,'Height',1.4,'OriginOffset',[-1.35 0 0],'MeshVertices',[3.7 -0.9 1.4;3.7 0.9 1.4;-1 0.9 1.4;-1 -0.9 1.4;3.7 -0.9 0;3.7 0.9 0;-1 0.9 0;-1 -0.9 0],'MeshFaces',[6 2 1;1 5 6;8 4 3;3 7 8;6 7 3;3 2 6;5 1 4;4 8 5;4 1 2;2 3 4;7 6 5;5 8 7],'RCSPattern',[10 10;10 10],'RCSAzimuthAngles',[-180 180],'RCSElevationAngles',[-90 90]); struct('ActorID',5,'ClassID',1,'Length',4.7,'Width',1.8,'Height',1.4,'OriginOffset',[-1.35 0 0],'MeshVertices',[3.7 -0.9 1.4;3.7 0.9 1.4;-1 0.9 1.4;-1 -0.9 1.4;3.7 -0.9 0;3.7 0.9 0;-1 0.9 0;-1 -0.9 0],'MeshFaces',[6 2 1;1 5 6;8 4 3;3 7 8;6 7 3;3 2 6;5 1 4;4 8 5;4 1 2;2 3 4;7 6 5;5 8 7],'RCSPattern',[10 10;10 10],'RCSAzimuthAngles',[-180 180],'RCSElevationAngles',[-90 90]); struct('ActorID',6,'ClassID',4,'Length',0.24,'Width',0.45,'Height',1.7,'OriginOffset',[0 0 0],'MeshVertices',[0.12 -0.225 1.7;0.12 0.225 1.7;-0.12 0.225 1.7;-0.12 -0.225 1.7;0.12 -0.225 -1.11022302462516e-16;0.12 0.225 -1.11022302462516e-16;-0.12 0.225 -1.11022302462516e-16;-0.12 -0.225 -1.11022302462516e-16],'MeshFaces',[6 2 1;1 5 6;8 4 3;3 7 8;6 7 3;3 2 6;5 1 4;4 8 5;4 1 2;2 3 4;7 6 5;5 8 7],'RCSPattern',[-8 -8;-8 -8],'RCSAzimuthAngles',[-180 180],'RCSElevationAngles',[-90 90]); struct('ActorID',7,'ClassID',4,'Length',0.24,'Width',0.45,'Height',1.7,'OriginOffset',[0 0 0],'MeshVertices',[0.12 -0.225 1.7;0.12 0.225 1.7;-0.12 0.225 1.7;-0.12 -0.225 1.7;0.12 -0.225 -1.11022302462516e-16;0.12 0.225 -1.11022302462516e-16;-0.12 0.225 -1.11022302462516e-16;-0.12 -0.225 -1.11022302462516e-16],'MeshFaces',[6 2 1;1 5 6;8 4 3;3 7 8;6 7 3;3 2 6;5 1 4;4 8 5;4 1 2;2 3 4;7 6 5;5 8 7],'RCSPattern',[-8 -8;-8 -8],'RCSAzimuthAngles',[-180 180],'RCSElevationAngles',[-90 90]); struct('ActorID',8,'ClassID',4,'Length',0.24,'Width',0.45,'Height',1.7,'OriginOffset',[0 0 0],'MeshVertices',[0.12 -0.225 1.7;0.12 0.225 1.7;-0.12 0.225 1.7;-0.12 -0.225 1.7;0.12 -0.225 -1.11022302462516e-16;0.12 0.225 -1.11022302462516e-16;-0.12 0.225 -1.11022302462516e-16;-0.12 -0.225 -1.11022302462516e-16],'MeshFaces',[6 2 1;1 5 6;8 4 3;3 7 8;6 7 3;3 2 6;5 1 4;4 8 5;4 1 2;2 3 4;7 6 5;5 8 7],'RCSPattern',[-8 -8;-8 -8],'RCSAzimuthAngles',[-180 180],'RCSElevationAngles',[-90 90]); struct('ActorID',9,'ClassID',4,'Length',0.24,'Width',0.45,'Height',1.7,'OriginOffset',[0 0 0],'MeshVertices',[0.12 -0.225 1.7;0.12 0.225 1.7;-0.12 0.225 1.7;-0.12 -0.225 1.7;0.12 -0.225 -1.11022302462516e-16;0.12 0.225 -1.11022302462516e-16;-0.12 0.225 -1.11022302462516e-16;-0.12 -0.225 -1.11022302462516e-16],'MeshFaces',[6 2 1;1 5 6;8 4 3;3 7 8;6 7 3;3 2 6;5 1 4;4 8 5;4 1 2;2 3 4;7 6 5;5 8 7],'RCSPattern',[-8 -8;-8 -8],'RCSAzimuthAngles',[-180 180],'RCSElevationAngles',[-90 90]); struct('ActorID',10,'ClassID',4,'Length',0.24,'Width',0.45,'Height',1.7,'OriginOffset',[0 0 0],'MeshVertices',[0.12 -0.225 1.7;0.12 0.225 1.7;-0.12 0.225 1.7;-0.12 -0.225 1.7;0.12 -0.225 -1.11022302462516e-16;0.12 0.225 -1.11022302462516e-16;-0.12 0.225 -1.11022302462516e-16;-0.12 -0.225 -1.11022302462516e-16],'MeshFaces',[6 2 1;1 5 6;8 4 3;3 7 8;6 7 3;3 2 6;5 1 4;4 8 5;4 1 2;2 3 4;7 6 5;5 8 7],'RCSPattern',[-8 -8;-8 -8],'RCSAzimuthAngles',[-180 180],'RCSElevationAngles',[-90 90]); struct('ActorID',11,'ClassID',4,'Length',0.24,'Width',0.45,'Height',1.7,'OriginOffset',[0 0 0],'MeshVertices',[0.12 -0.225 1.7;0.12 0.225 1.7;-0.12 0.225 1.7;-0.12 -0.225 1.7;0.12 -0.225 -1.11022302462516e-16;0.12 0.225 -1.11022302462516e-16;-0.12 0.225 -1.11022302462516e-16;-0.12 -0.225 -1.11022302462516e-16],'MeshFaces',[6 2 1;1 5 6;8 4 3;3 7 8;6 7 3;3 2 6;5 1 4;4 8 5;4 1 2;2 3 4;7 6 5;5 8 7],'RCSPattern',[-8 -8;-8 -8],'RCSAzimuthAngles',[-180 180],'RCSElevationAngles',[-90 90]); struct('ActorID',12,'ClassID',4,'Length',0.24,'Width',0.45,'Height',1.7,'OriginOffset',[0 0 0],'MeshVertices',[0.12 -0.225 1.7;0.12 0.225 1.7;-0.12 0.225 1.7;-0.12 -0.225 1.7;0.12 -0.225 -1.11022302462516e-16;0.12 0.225 -1.11022302462516e-16;-0.12 0.225 -1.11022302462516e-16;-0.12 -0.225 -1.11022302462516e-16],'MeshFaces',[6 2 1;1 5 6;8 4 3;3 7 8;6 7 3;3 2 6;5 1 4;4 8 5;4 1 2;2 3 4;7 6 5;5 8 7],'RCSPattern',[-8 -8;-8 -8],'RCSAzimuthAngles',[-180 180],'RCSElevationAngles',[-90 90]); struct('ActorID',13,'ClassID',4,'Length',0.24,'Width',0.45,'Height',1.7,'OriginOffset',[0 0 0],'MeshVertices',[0.12 -0.225 1.7;0.12 0.225 1.7;-0.12 0.225 1.7;-0.12 -0.225 1.7;0.12 -0.225 -1.11022302462516e-16;0.12 0.225 -1.11022302462516e-16;-0.12 0.225 -1.11022302462516e-16;-0.12 -0.225 -1.11022302462516e-16],'MeshFaces',[6 2 1;1 5 6;8 4 3;3 7 8;6 7 3;3 2 6;5 1 4;4 8 5;4 1 2;2 3 4;7 6 5;5 8 7],'RCSPattern',[-8 -8;-8 -8],'RCSAzimuthAngles',[-180 180],'RCSElevationAngles',[-90 90]); struct('ActorID',14,'ClassID',4,'Length',0.24,'Width',0.45,'Height',1.7,'OriginOffset',[0 0 0],'MeshVertices',[0.12 -0.225 1.7;0.12 0.225 1.7;-0.12 0.225 1.7;-0.12 -0.225 1.7;0.12 -0.225 -1.11022302462516e-16;0.12 0.225 -1.11022302462516e-16;-0.12 0.225 -1.11022302462516e-16;-0.12 -0.225 -1.11022302462516e-16],'MeshFaces',[6 2 1;1 5 6;8 4 3;3 7 8;6 7 3;3 2 6;5 1 4;4 8 5;4 1 2;2 3 4;7 6 5;5 8 7],'RCSPattern',[-8 -8;-8 -8],'RCSAzimuthAngles',[-180 180],'RCSElevationAngles',[-90 90]); struct('ActorID',15,'ClassID',4,'Length',0.24,'Width',0.45,'Height',1.7,'OriginOffset',[0 0 0],'MeshVertices',[0.12 -0.225 1.7;0.12 0.225 1.7;-0.12 0.225 1.7;-0.12 -0.225 1.7;0.12 -0.225 -1.11022302462516e-16;0.12 0.225 -1.11022302462516e-16;-0.12 0.225 -1.11022302462516e-16;-0.12 -0.225 -1.11022302462516e-16],'MeshFaces',[6 2 1;1 5 6;8 4 3;3 7 8;6 7 3;3 2 6;5 1 4;4 8 5;4 1 2;2 3 4;7 6 5;5 8 7],'RCSPattern',[-8 -8;-8 -8],'RCSAzimuthAngles',[-180 180],'RCSElevationAngles',[-90 90]); struct('ActorID',16,'ClassID',4,'Length',0.24,'Width',0.45,'Height',1.7,'OriginOffset',[0 0 0],'MeshVertices',[0.12 -0.225 1.7;0.12 0.225 1.7;-0.12 0.225 1.7;-0.12 -0.225 1.7;0.12 -0.225 -1.11022302462516e-16;0.12 0.225 -1.11022302462516e-16;-0.12 0.225 -1.11022302462516e-16;-0.12 -0.225 -1.11022302462516e-16],'MeshFaces',[6 2 1;1 5 6;8 4 3;3 7 8;6 7 3;3 2 6;5 1 4;4 8 5;4 1 2;2 3 4;7 6 5;5 8 7],'RCSPattern',[-8 -8;-8 -8],'RCSAzimuthAngles',[-180 180],'RCSElevationAngles',[-90 90]); struct('ActorID',17,'ClassID',4,'Length',0.24,'Width',0.45,'Height',1.7,'OriginOffset',[0 0 0],'MeshVertices',[0.12 -0.225 1.7;0.12 0.225 1.7;-0.12 0.225 1.7;-0.12 -0.225 1.7;0.12 -0.225 -1.11022302462516e-16;0.12 0.225 -1.11022302462516e-16;-0.12 0.225 -1.11022302462516e-16;-0.12 -0.225 -1.11022302462516e-16],'MeshFaces',[6 2 1;1 5 6;8 4 3;3 7 8;6 7 3;3 2 6;5 1 4;4 8 5;4 1 2;2 3 4;7 6 5;5 8 7],'RCSPattern',[-8 -8;-8 -8],'RCSAzimuthAngles',[-180 180],'RCSElevationAngles',[-90 90]); struct('ActorID',18,'ClassID',4,'Length',0.24,'Width',0.45,'Height',1.7,'OriginOffset',[0 0 0],'MeshVertices',[0.12 -0.225 1.7;0.12 0.225 1.7;-0.12 0.225 1.7;-0.12 -0.225 1.7;0.12 -0.225 -1.11022302462516e-16;0.12 0.225 -1.11022302462516e-16;-0.12 0.225 -1.11022302462516e-16;-0.12 -0.225 -1.11022302462516e-16],'MeshFaces',[6 2 1;1 5 6;8 4 3;3 7 8;6 7 3;3 2 6;5 1 4;4 8 5;4 1 2;2 3 4;7 6 5;5 8 7],'RCSPattern',[-8 -8;-8 -8],'RCSAzimuthAngles',[-180 180],'RCSElevationAngles',[-90 90]); struct('ActorID',19,'ClassID',4,'Length',0.24,'Width',0.45,'Height',1.7,'OriginOffset',[0 0 0],'MeshVertices',[0.12 -0.225 1.7;0.12 0.225 1.7;-0.12 0.225 1.7;-0.12 -0.225 1.7;0.12 -0.225 -1.11022302462516e-16;0.12 0.225 -1.11022302462516e-16;-0.12 0.225 -1.11022302462516e-16;-0.12 -0.225 -1.11022302462516e-16],'MeshFaces',[6 2 1;1 5 6;8 4 3;3 7 8;6 7 3;3 2 6;5 1 4;4 8 5;4 1 2;2 3 4;7 6 5;5 8 7],'RCSPattern',[-8 -8;-8 -8],'RCSAzimuthAngles',[-180 180],'RCSElevationAngles',[-90 90]); struct('ActorID',20,'ClassID',4,'Length',0.24,'Width',0.45,'Height',1.7,'OriginOffset',[0 0 0],'MeshVertices',[0.12 -0.225 1.7;0.12 0.225 1.7;-0.12 0.225 1.7;-0.12 -0.225 1.7;0.12 -0.225 -1.11022302462516e-16;0.12 0.225 -1.11022302462516e-16;-0.12 0.225 -1.11022302462516e-16;-0.12 -0.225 -1.11022302462516e-16],'MeshFaces',[6 2 1;1 5 6;8 4 3;3 7 8;6 7 3;3 2 6;5 1 4;4 8 5;4 1 2;2 3 4;7 6 5;5 8 7],'RCSPattern',[-8 -8;-8 -8],'RCSAzimuthAngles',[-180 180],'RCSElevationAngles',[-90 90]); struct('ActorID',21,'ClassID',4,'Length',0.24,'Width',0.45,'Height',1.7,'OriginOffset',[0 0 0],'MeshVertices',[0.12 -0.225 1.7;0.12 0.225 1.7;-0.12 0.225 1.7;-0.12 -0.225 1.7;0.12 -0.225 -1.11022302462516e-16;0.12 0.225 -1.11022302462516e-16;-0.12 0.225 -1.11022302462516e-16;-0.12 -0.225 -1.11022302462516e-16],'MeshFaces',[6 2 1;1 5 6;8 4 3;3 7 8;6 7 3;3 2 6;5 1 4;4 8 5;4 1 2;2 3 4;7 6 5;5 8 7],'RCSPattern',[-8 -8;-8 -8],'RCSAzimuthAngles',[-180 180],'RCSElevationAngles',[-90 90]); struct('ActorID',22,'ClassID',4,'Length',0.24,'Width',0.45,'Height',1.7,'OriginOffset',[0 0 0],'MeshVertices',[0.12 -0.225 1.7;0.12 0.225 1.7;-0.12 0.225 1.7;-0.12 -0.225 1.7;0.12 -0.225 -1.11022302462516e-16;0.12 0.225 -1.11022302462516e-16;-0.12 0.225 -1.11022302462516e-16;-0.12 -0.225 -1.11022302462516e-16],'MeshFaces',[6 2 1;1 5 6;8 4 3;3 7 8;6 7 3;3 2 6;5 1 4;4 8 5;4 1 2;2 3 4;7 6 5;5 8 7],'RCSPattern',[-8 -8;-8 -8],'RCSAzimuthAngles',[-180 180],'RCSElevationAngles',[-90 90]); struct('ActorID',23,'ClassID',4,'Length',0.24,'Width',0.45,'Height',1.7,'OriginOffset',[0 0 0],'MeshVertices',[0.12 -0.225 1.7;0.12 0.225 1.7;-0.12 0.225 1.7;-0.12 -0.225 1.7;0.12 -0.225 -1.11022302462516e-16;0.12 0.225 -1.11022302462516e-16;-0.12 0.225 -1.11022302462516e-16;-0.12 -0.225 -1.11022302462516e-16],'MeshFaces',[6 2 1;1 5 6;8 4 3;3 7 8;6 7 3;3 2 6;5 1 4;4 8 5;4 1 2;2 3 4;7 6 5;5 8 7],'RCSPattern',[-8 -8;-8 -8],'RCSAzimuthAngles',[-180 180],'RCSElevationAngles',[-90 90]); struct('ActorID',24,'ClassID',4,'Length',0.24,'Width',0.45,'Height',1.7,'OriginOffset',[0 0 0],'MeshVertices',[0.12 -0.225 1.7;0.12 0.225 1.7;-0.12 0.225 1.7;-0.12 -0.225 1.7;0.12 -0.225 -1.11022302462516e-16;0.12 0.225 -1.11022302462516e-16;-0.12 0.225 -1.11022302462516e-16;-0.12 -0.225 -1.11022302462516e-16],'MeshFaces',[6 2 1;1 5 6;8 4 3;3 7 8;6 7 3;3 2 6;5 1 4;4 8 5;4 1 2;2 3 4;7 6 5;5 8 7],'RCSPattern',[-8 -8;-8 -8],'RCSAzimuthAngles',[-180 180],'RCSElevationAngles',[-90 90]); struct('ActorID',25,'ClassID',4,'Length',0.24,'Width',0.45,'Height',1.7,'OriginOffset',[0 0 0],'MeshVertices',[0.12 -0.225 1.7;0.12 0.225 1.7;-0.12 0.225 1.7;-0.12 -0.225 1.7;0.12 -0.225 -1.11022302462516e-16;0.12 0.225 -1.11022302462516e-16;-0.12 0.225 -1.11022302462516e-16;-0.12 -0.225 -1.11022302462516e-16],'MeshFaces',[6 2 1;1 5 6;8 4 3;3 7 8;6 7 3;3 2 6;5 1 4;4 8 5;4 1 2;2 3 4;7 6 5;5 8 7],'RCSPattern',[-8 -8;-8 -8],'RCSAzimuthAngles',[-180 180],'RCSElevationAngles',[-90 90]); struct('ActorID',26,'ClassID',4,'Length',0.24,'Width',0.45,'Height',1.7,'OriginOffset',[0 0 0],'MeshVertices',[0.12 -0.225 1.7;0.12 0.225 1.7;-0.12 0.225 1.7;-0.12 -0.225 1.7;0.12 -0.225 -1.11022302462516e-16;0.12 0.225 -1.11022302462516e-16;-0.12 0.225 -1.11022302462516e-16;-0.12 -0.225 -1.11022302462516e-16],'MeshFaces',[6 2 1;1 5 6;8 4 3;3 7 8;6 7 3;3 2 6;5 1 4;4 8 5;4 1 2;2 3 4;7 6 5;5 8 7],'RCSPattern',[-8 -8;-8 -8],'RCSAzimuthAngles',[-180 180],'RCSElevationAngles',[-90 90]); struct('ActorID',27,'ClassID',4,'Length',0.24,'Width',0.45,'Height',1.7,'OriginOffset',[0 0 0],'MeshVertices',[0.12 -0.225 1.7;0.12 0.225 1.7;-0.12 0.225 1.7;-0.12 -0.225 1.7;0.12 -0.225 -1.11022302462516e-16;0.12 0.225 -1.11022302462516e-16;-0.12 0.225 -1.11022302462516e-16;-0.12 -0.225 -1.11022302462516e-16],'MeshFaces',[6 2 1;1 5 6;8 4 3;3 7 8;6 7 3;3 2 6;5 1 4;4 8 5;4 1 2;2 3 4;7 6 5;5 8 7],'RCSPattern',[-8 -8;-8 -8],'RCSAzimuthAngles',[-180 180],'RCSElevationAngles',[-90 90]); struct('ActorID',28,'ClassID',3,'Length',1.7,'Width',0.45,'Height',1.7,'OriginOffset',[0 0 0],'MeshVertices',[0.85 -0.225 1.7;0.85 0.225 1.7;-0.85 0.225 1.7;-0.85 -0.225 1.7;0.85 -0.225 -1.11022302462516e-16;0.85 0.225 -1.11022302462516e-16;-0.85 0.225 -1.11022302462516e-16;-0.85 -0.225 -1.11022302462516e-16],'MeshFaces',[6 2 1;1 5 6;8 4 3;3 7 8;6 7 3;3 2 6;5 1 4;4 8 5;4 1 2;2 3 4;7 6 5;5 8 7],'RCSPattern',[10 10;10 10],'RCSAzimuthAngles',[-180 180],'RCSElevationAngles',[-90 90]); struct('ActorID',29,'ClassID',4,'Length',0.24,'Width',0.45,'Height',1.7,'OriginOffset',[0 0 0],'MeshVertices',[0.12 -0.225 1.7;0.12 0.225 1.7;-0.12 0.225 1.7;-0.12 -0.225 1.7;0.12 -0.225 -1.11022302462516e-16;0.12 0.225 -1.11022302462516e-16;-0.12 0.225 -1.11022302462516e-16;-0.12 -0.225 -1.11022302462516e-16],'MeshFaces',[6 2 1;1 5 6;8 4 3;3 7 8;6 7 3;3 2 6;5 1 4;4 8 5;4 1 2;2 3 4;7 6 5;5 8 7],'RCSPattern',[-8 -8;-8 -8],'RCSAzimuthAngles',[-180 180],'RCSElevationAngles',[-90 90])]  Intrinsics=driving.internal.cameraIntrinsics('FocalLength',[320 320],'PrincipalPoint',[320 240],'ImageSize',[480 640],'RadialDistortion',[0 0],'TangentialDistortion',[0 0],'Skew',0)
  Camera3 : drivingscenarioandsensors/Vision Detection Generator  SensorIndex=9  DetectorOutput=Objects only  UpdateInterval=0.1  LaneUpdateInterval=0.1  SensorLocation=[3.7 0]  Height=1.1  Yaw=64.0691935373481  Pitch=1  Roll=0  BusNameSource=Auto  BusName=BusObjectDetections  BusName2Source=Auto  BusName2=BusLaneDetections  MaxNumDetectionsSource=Property  MaxNumDetections=50  MaxNumLanesSource=Property  MaxNumLanes=30  DetectionCoordinates=Ego Cartesian  SimulateUsing=Interpreted execution  MaxRange=10  BoundingBoxAccuracy=5  ProcessNoiseIntensity=5  MaxSpeed=50  MaxAllowedOcclusion=0.5  MinObjectImageSize=[15 15]  DetectionProbability=0.2  FalsePositivesPerImage=0.1  MinLaneImageSize=[20 3]  LaneBoundaryAccuracy=3  HasNoise=on  InitialSeedSource=Repeatable  InitialSeed=0  UsedSeed=0  ActorProfilesSource=MATLAB expression  ActorProfilesParameters=driving.internal.ActorProfilesParameters  ActorProfilesExpression=[struct('ActorID',1,'ClassID',1,'Length',4.7,'Width',1.8,'Height',1.4,'OriginOffset',[-1.35 0 0],'MeshVertices',[3.7 -0.9 1.4;3.7 0.9 1.4;-1 0.9 1.4;-1 -0.9 1.4;3.7 -0.9 0;3.7 0.9 0;-1 0.9 0;-1 -0.9 0],'MeshFaces',[6 2 1;1 5 6;8 4 3;3 7 8;6 7 3;3 2 6;5 1 4;4 8 5;4 1 2;2 3 4;7 6 5;5 8 7],'RCSPattern',[10 10;10 10],'RCSAzimuthAngles',[-180 180],'RCSElevationAngles',[-90 90]); struct('ActorID',2,'ClassID',1,'Length',4.7,'Width',1.8,'Height',1.4,'OriginOffset',[-1.35 0 0],'MeshVertices',[3.7 -0.9 1.4;3.7 0.9 1.4;-1 0.9 1.4;-1 -0.9 1.4;3.7 -0.9 0;3.7 0.9 0;-1 0.9 0;-1 -0.9 0],'MeshFaces',[6 2 1;1 5 6;8 4 3;3 7 8;6 7 3;3 2 6;5 1 4;4 8 5;4 1 2;2 3 4;7 6 5;5 8 7],'RCSPattern',[10 10;10 10],'RCSAzimuthAngles',[-180 180],'RCSElevationAngles',[-90 90]); struct('ActorID',3,'ClassID',1,'Length',4.7,'Width',1.8,'Height',1.4,'OriginOffset',[-1.35 0 0],'MeshVertices',[3.7 -0.9 1.4;3.7 0.9 1.4;-1 0.9 1.4;-1 -0.9 1.4;3.7 -0.9 0;3.7 0.9 0;-1 0.9 0;-1 -0.9 0],'MeshFaces',[6 2 1;1 5 6;8 4 3;3 7 8;6 7 3;3 2 6;5 1 4;4 8 5;4 1 2;2 3 4;7 6 5;5 8 7],'RCSPattern',[10 10;10 10],'RCSAzimuthAngles',[-180 180],'RCSElevationAngles',[-90 90]); struct('ActorID',4,'ClassID',1,'Length',4.7,'Width',1.8,'Height',1.4,'OriginOffset',[-1.35 0 0],'MeshVertices',[3.7 -0.9 1.4;3.7 0.9 1.4;-1 0.9 1.4;-1 -0.9 1.4;3.7 -0.9 0;3.7 0.9 0;-1 0.9 0;-1 -0.9 0],'MeshFaces',[6 2 1;1 5 6;8 4 3;3 7 8;6 7 3;3 2 6;5 1 4;4 8 5;4 1 2;2 3 4;7 6 5;5 8 7],'RCSPattern',[10 10;10 10],'RCSAzimuthAngles',[-180 180],'RCSElevationAngles',[-90 90]); struct('ActorID',5,'ClassID',1,'Length',4.7,'Width',1.8,'Height',1.4,'OriginOffset',[-1.35 0 0],'MeshVertices',[3.7 -0.9 1.4;3.7 0.9 1.4;-1 0.9 1.4;-1 -0.9 1.4;3.7 -0.9 0;3.7 0.9 0;-1 0.9 0;-1 -0.9 0],'MeshFaces',[6 2 1;1 5 6;8 4 3;3 7 8;6 7 3;3 2 6;5 1 4;4 8 5;4 1 2;2 3 4;7 6 5;5 8 7],'RCSPattern',[10 10;10 10],'RCSAzimuthAngles',[-180 180],'RCSElevationAngles',[-90 90]); struct('ActorID',6,'ClassID',4,'Length',0.24,'Width',0.45,'Height',1.7,'OriginOffset',[0 0 0],'MeshVertices',[0.12 -0.225 1.7;0.12 0.225 1.7;-0.12 0.225 1.7;-0.12 -0.225 1.7;0.12 -0.225 -1.11022302462516e-16;0.12 0.225 -1.11022302462516e-16;-0.12 0.225 -1.11022302462516e-16;-0.12 -0.225 -1.11022302462516e-16],'MeshFaces',[6 2 1;1 5 6;8 4 3;3 7 8;6 7 3;3 2 6;5 1 4;4 8 5;4 1 2;2 3 4;7 6 5;5 8 7],'RCSPattern',[-8 -8;-8 -8],'RCSAzimuthAngles',[-180 180],'RCSElevationAngles',[-90 90]); struct('ActorID',7,'ClassID',4,'Length',0.24,'Width',0.45,'Height',1.7,'OriginOffset',[0 0 0],'MeshVertices',[0.12 -0.225 1.7;0.12 0.225 1.7;-0.12 0.225 1.7;-0.12 -0.225 1.7;0.12 -0.225 -1.11022302462516e-16;0.12 0.225 -1.11022302462516e-16;-0.12 0.225 -1.11022302462516e-16;-0.12 -0.225 -1.11022302462516e-16],'MeshFaces',[6 2 1;1 5 6;8 4 3;3 7 8;6 7 3;3 2 6;5 1 4;4 8 5;4 1 2;2 3 4;7 6 5;5 8 7],'RCSPattern',[-8 -8;-8 -8],'RCSAzimuthAngles',[-180 180],'RCSElevationAngles',[-90 90]); struct('ActorID',8,'ClassID',4,'Length',0.24,'Width',0.45,'Height',1.7,'OriginOffset',[0 0 0],'MeshVertices',[0.12 -0.225 1.7;0.12 0.225 1.7;-0.12 0.225 1.7;-0.12 -0.225 1.7;0.12 -0.225 -1.11022302462516e-16;0.12 0.225 -1.11022302462516e-16;-0.12 0.225 -1.11022302462516e-16;-0.12 -0.225 -1.11022302462516e-16],'MeshFaces',[6 2 1;1 5 6;8 4 3;3 7 8;6 7 3;3 2 6;5 1 4;4 8 5;4 1 2;2 3 4;7 6 5;5 8 7],'RCSPattern',[-8 -8;-8 -8],'RCSAzimuthAngles',[-180 180],'RCSElevationAngles',[-90 90]); struct('ActorID',9,'ClassID',4,'Length',0.24,'Width',0.45,'Height',1.7,'OriginOffset',[0 0 0],'MeshVertices',[0.12 -0.225 1.7;0.12 0.225 1.7;-0.12 0.225 1.7;-0.12 -0.225 1.7;0.12 -0.225 -1.11022302462516e-16;0.12 0.225 -1.11022302462516e-16;-0.12 0.225 -1.11022302462516e-16;-0.12 -0.225 -1.11022302462516e-16],'MeshFaces',[6 2 1;1 5 6;8 4 3;3 7 8;6 7 3;3 2 6;5 1 4;4 8 5;4 1 2;2 3 4;7 6 5;5 8 7],'RCSPattern',[-8 -8;-8 -8],'RCSAzimuthAngles',[-180 180],'RCSElevationAngles',[-90 90]); struct('ActorID',10,'ClassID',4,'Length',0.24,'Width',0.45,'Height',1.7,'OriginOffset',[0 0 0],'MeshVertices',[0.12 -0.225 1.7;0.12 0.225 1.7;-0.12 0.225 1.7;-0.12 -0.225 1.7;0.12 -0.225 -1.11022302462516e-16;0.12 0.225 -1.11022302462516e-16;-0.12 0.225 -1.11022302462516e-16;-0.12 -0.225 -1.11022302462516e-16],'MeshFaces',[6 2 1;1 5 6;8 4 3;3 7 8;6 7 3;3 2 6;5 1 4;4 8 5;4 1 2;2 3 4;7 6 5;5 8 7],'RCSPattern',[-8 -8;-8 -8],'RCSAzimuthAngles',[-180 180],'RCSElevationAngles',[-90 90]); struct('ActorID',11,'ClassID',4,'Length',0.24,'Width',0.45,'Height',1.7,'OriginOffset',[0 0 0],'MeshVertices',[0.12 -0.225 1.7;0.12 0.225 1.7;-0.12 0.225 1.7;-0.12 -0.225 1.7;0.12 -0.225 -1.11022302462516e-16;0.12 0.225 -1.11022302462516e-16;-0.12 0.225 -1.11022302462516e-16;-0.12 -0.225 -1.11022302462516e-16],'MeshFaces',[6 2 1;1 5 6;8 4 3;3 7 8;6 7 3;3 2 6;5 1 4;4 8 5;4 1 2;2 3 4;7 6 5;5 8 7],'RCSPattern',[-8 -8;-8 -8],'RCSAzimuthAngles',[-180 180],'RCSElevationAngles',[-90 90]); struct('ActorID',12,'ClassID',4,'Length',0.24,'Width',0.45,'Height',1.7,'OriginOffset',[0 0 0],'MeshVertices',[0.12 -0.225 1.7;0.12 0.225 1.7;-0.12 0.225 1.7;-0.12 -0.225 1.7;0.12 -0.225 -1.11022302462516e-16;0.12 0.225 -1.11022302462516e-16;-0.12 0.225 -1.11022302462516e-16;-0.12 -0.225 -1.11022302462516e-16],'MeshFaces',[6 2 1;1 5 6;8 4 3;3 7 8;6 7 3;3 2 6;5 1 4;4 8 5;4 1 2;2 3 4;7 6 5;5 8 7],'RCSPattern',[-8 -8;-8 -8],'RCSAzimuthAngles',[-180 180],'RCSElevationAngles',[-90 90]); struct('ActorID',13,'ClassID',4,'Length',0.24,'Width',0.45,'Height',1.7,'OriginOffset',[0 0 0],'MeshVertices',[0.12 -0.225 1.7;0.12 0.225 1.7;-0.12 0.225 1.7;-0.12 -0.225 1.7;0.12 -0.225 -1.11022302462516e-16;0.12 0.225 -1.11022302462516e-16;-0.12 0.225 -1.11022302462516e-16;-0.12 -0.225 -1.11022302462516e-16],'MeshFaces',[6 2 1;1 5 6;8 4 3;3 7 8;6 7 3;3 2 6;5 1 4;4 8 5;4 1 2;2 3 4;7 6 5;5 8 7],'RCSPattern',[-8 -8;-8 -8],'RCSAzimuthAngles',[-180 180],'RCSElevationAngles',[-90 90]); struct('ActorID',14,'ClassID',4,'Length',0.24,'Width',0.45,'Height',1.7,'OriginOffset',[0 0 0],'MeshVertices',[0.12 -0.225 1.7;0.12 0.225 1.7;-0.12 0.225 1.7;-0.12 -0.225 1.7;0.12 -0.225 -1.11022302462516e-16;0.12 0.225 -1.11022302462516e-16;-0.12 0.225 -1.11022302462516e-16;-0.12 -0.225 -1.11022302462516e-16],'MeshFaces',[6 2 1;1 5 6;8 4 3;3 7 8;6 7 3;3 2 6;5 1 4;4 8 5;4 1 2;2 3 4;7 6 5;5 8 7],'RCSPattern',[-8 -8;-8 -8],'RCSAzimuthAngles',[-180 180],'RCSElevationAngles',[-90 90]); struct('ActorID',15,'ClassID',4,'Length',0.24,'Width',0.45,'Height',1.7,'OriginOffset',[0 0 0],'MeshVertices',[0.12 -0.225 1.7;0.12 0.225 1.7;-0.12 0.225 1.7;-0.12 -0.225 1.7;0.12 -0.225 -1.11022302462516e-16;0.12 0.225 -1.11022302462516e-16;-0.12 0.225 -1.11022302462516e-16;-0.12 -0.225 -1.11022302462516e-16],'MeshFaces',[6 2 1;1 5 6;8 4 3;3 7 8;6 7 3;3 2 6;5 1 4;4 8 5;4 1 2;2 3 4;7 6 5;5 8 7],'RCSPattern',[-8 -8;-8 -8],'RCSAzimuthAngles',[-180 180],'RCSElevationAngles',[-90 90]); struct('ActorID',16,'ClassID',4,'Length',0.24,'Width',0.45,'Height',1.7,'OriginOffset',[0 0 0],'MeshVertices',[0.12 -0.225 1.7;0.12 0.225 1.7;-0.12 0.225 1.7;-0.12 -0.225 1.7;0.12 -0.225 -1.11022302462516e-16;0.12 0.225 -1.11022302462516e-16;-0.12 0.225 -1.11022302462516e-16;-0.12 -0.225 -1.11022302462516e-16],'MeshFaces',[6 2 1;1 5 6;8 4 3;3 7 8;6 7 3;3 2 6;5 1 4;4 8 5;4 1 2;2 3 4;7 6 5;5 8 7],'RCSPattern',[-8 -8;-8 -8],'RCSAzimuthAngles',[-180 180],'RCSElevationAngles',[-90 90]); struct('ActorID',17,'ClassID',4,'Length',0.24,'Width',0.45,'Height',1.7,'OriginOffset',[0 0 0],'MeshVertices',[0.12 -0.225 1.7;0.12 0.225 1.7;-0.12 0.225 1.7;-0.12 -0.225 1.7;0.12 -0.225 -1.11022302462516e-16;0.12 0.225 -1.11022302462516e-16;-0.12 0.225 -1.11022302462516e-16;-0.12 -0.225 -1.11022302462516e-16],'MeshFaces',[6 2 1;1 5 6;8 4 3;3 7 8;6 7 3;3 2 6;5 1 4;4 8 5;4 1 2;2 3 4;7 6 5;5 8 7],'RCSPattern',[-8 -8;-8 -8],'RCSAzimuthAngles',[-180 180],'RCSElevationAngles',[-90 90]); struct('ActorID',18,'ClassID',4,'Length',0.24,'Width',0.45,'Height',1.7,'OriginOffset',[0 0 0],'MeshVertices',[0.12 -0.225 1.7;0.12 0.225 1.7;-0.12 0.225 1.7;-0.12 -0.225 1.7;0.12 -0.225 -1.11022302462516e-16;0.12 0.225 -1.11022302462516e-16;-0.12 0.225 -1.11022302462516e-16;-0.12 -0.225 -1.11022302462516e-16],'MeshFaces',[6 2 1;1 5 6;8 4 3;3 7 8;6 7 3;3 2 6;5 1 4;4 8 5;4 1 2;2 3 4;7 6 5;5 8 7],'RCSPattern',[-8 -8;-8 -8],'RCSAzimuthAngles',[-180 180],'RCSElevationAngles',[-90 90]); struct('ActorID',19,'ClassID',4,'Length',0.24,'Width',0.45,'Height',1.7,'OriginOffset',[0 0 0],'MeshVertices',[0.12 -0.225 1.7;0.12 0.225 1.7;-0.12 0.225 1.7;-0.12 -0.225 1.7;0.12 -0.225 -1.11022302462516e-16;0.12 0.225 -1.11022302462516e-16;-0.12 0.225 -1.11022302462516e-16;-0.12 -0.225 -1.11022302462516e-16],'MeshFaces',[6 2 1;1 5 6;8 4 3;3 7 8;6 7 3;3 2 6;5 1 4;4 8 5;4 1 2;2 3 4;7 6 5;5 8 7],'RCSPattern',[-8 -8;-8 -8],'RCSAzimuthAngles',[-180 180],'RCSElevationAngles',[-90 90]); struct('ActorID',20,'ClassID',4,'Length',0.24,'Width',0.45,'Height',1.7,'OriginOffset',[0 0 0],'MeshVertices',[0.12 -0.225 1.7;0.12 0.225 1.7;-0.12 0.225 1.7;-0.12 -0.225 1.7;0.12 -0.225 -1.11022302462516e-16;0.12 0.225 -1.11022302462516e-16;-0.12 0.225 -1.11022302462516e-16;-0.12 -0.225 -1.11022302462516e-16],'MeshFaces',[6 2 1;1 5 6;8 4 3;3 7 8;6 7 3;3 2 6;5 1 4;4 8 5;4 1 2;2 3 4;7 6 5;5 8 7],'RCSPattern',[-8 -8;-8 -8],'RCSAzimuthAngles',[-180 180],'RCSElevationAngles',[-90 90]); struct('ActorID',21,'ClassID',4,'Length',0.24,'Width',0.45,'Height',1.7,'OriginOffset',[0 0 0],'MeshVertices',[0.12 -0.225 1.7;0.12 0.225 1.7;-0.12 0.225 1.7;-0.12 -0.225 1.7;0.12 -0.225 -1.11022302462516e-16;0.12 0.225 -1.11022302462516e-16;-0.12 0.225 -1.11022302462516e-16;-0.12 -0.225 -1.11022302462516e-16],'MeshFaces',[6 2 1;1 5 6;8 4 3;3 7 8;6 7 3;3 2 6;5 1 4;4 8 5;4 1 2;2 3 4;7 6 5;5 8 7],'RCSPattern',[-8 -8;-8 -8],'RCSAzimuthAngles',[-180 180],'RCSElevationAngles',[-90 90]); struct('ActorID',22,'ClassID',4,'Length',0.24,'Width',0.45,'Height',1.7,'OriginOffset',[0 0 0],'MeshVertices',[0.12 -0.225 1.7;0.12 0.225 1.7;-0.12 0.225 1.7;-0.12 -0.225 1.7;0.12 -0.225 -1.11022302462516e-16;0.12 0.225 -1.11022302462516e-16;-0.12 0.225 -1.11022302462516e-16;-0.12 -0.225 -1.11022302462516e-16],'MeshFaces',[6 2 1;1 5 6;8 4 3;3 7 8;6 7 3;3 2 6;5 1 4;4 8 5;4 1 2;2 3 4;7 6 5;5 8 7],'RCSPattern',[-8 -8;-8 -8],'RCSAzimuthAngles',[-180 180],'RCSElevationAngles',[-90 90]); struct('ActorID',23,'ClassID',4,'Length',0.24,'Width',0.45,'Height',1.7,'OriginOffset',[0 0 0],'MeshVertices',[0.12 -0.225 1.7;0.12 0.225 1.7;-0.12 0.225 1.7;-0.12 -0.225 1.7;0.12 -0.225 -1.11022302462516e-16;0.12 0.225 -1.11022302462516e-16;-0.12 0.225 -1.11022302462516e-16;-0.12 -0.225 -1.11022302462516e-16],'MeshFaces',[6 2 1;1 5 6;8 4 3;3 7 8;6 7 3;3 2 6;5 1 4;4 8 5;4 1 2;2 3 4;7 6 5;5 8 7],'RCSPattern',[-8 -8;-8 -8],'RCSAzimuthAngles',[-180 180],'RCSElevationAngles',[-90 90]); struct('ActorID',24,'ClassID',4,'Length',0.24,'Width',0.45,'Height',1.7,'OriginOffset',[0 0 0],'MeshVertices',[0.12 -0.225 1.7;0.12 0.225 1.7;-0.12 0.225 1.7;-0.12 -0.225 1.7;0.12 -0.225 -1.11022302462516e-16;0.12 0.225 -1.11022302462516e-16;-0.12 0.225 -1.11022302462516e-16;-0.12 -0.225 -1.11022302462516e-16],'MeshFaces',[6 2 1;1 5 6;8 4 3;3 7 8;6 7 3;3 2 6;5 1 4;4 8 5;4 1 2;2 3 4;7 6 5;5 8 7],'RCSPattern',[-8 -8;-8 -8],'RCSAzimuthAngles',[-180 180],'RCSElevationAngles',[-90 90]); struct('ActorID',25,'ClassID',4,'Length',0.24,'Width',0.45,'Height',1.7,'OriginOffset',[0 0 0],'MeshVertices',[0.12 -0.225 1.7;0.12 0.225 1.7;-0.12 0.225 1.7;-0.12 -0.225 1.7;0.12 -0.225 -1.11022302462516e-16;0.12 0.225 -1.11022302462516e-16;-0.12 0.225 -1.11022302462516e-16;-0.12 -0.225 -1.11022302462516e-16],'MeshFaces',[6 2 1;1 5 6;8 4 3;3 7 8;6 7 3;3 2 6;5 1 4;4 8 5;4 1 2;2 3 4;7 6 5;5 8 7],'RCSPattern',[-8 -8;-8 -8],'RCSAzimuthAngles',[-180 180],'RCSElevationAngles',[-90 90]); struct('ActorID',26,'ClassID',4,'Length',0.24,'Width',0.45,'Height',1.7,'OriginOffset',[0 0 0],'MeshVertices',[0.12 -0.225 1.7;0.12 0.225 1.7;-0.12 0.225 1.7;-0.12 -0.225 1.7;0.12 -0.225 -1.11022302462516e-16;0.12 0.225 -1.11022302462516e-16;-0.12 0.225 -1.11022302462516e-16;-0.12 -0.225 -1.11022302462516e-16],'MeshFaces',[6 2 1;1 5 6;8 4 3;3 7 8;6 7 3;3 2 6;5 1 4;4 8 5;4 1 2;2 3 4;7 6 5;5 8 7],'RCSPattern',[-8 -8;-8 -8],'RCSAzimuthAngles',[-180 180],'RCSElevationAngles',[-90 90]); struct('ActorID',27,'ClassID',4,'Length',0.24,'Width',0.45,'Height',1.7,'OriginOffset',[0 0 0],'MeshVertices',[0.12 -0.225 1.7;0.12 0.225 1.7;-0.12 0.225 1.7;-0.12 -0.225 1.7;0.12 -0.225 -1.11022302462516e-16;0.12 0.225 -1.11022302462516e-16;-0.12 0.225 -1.11022302462516e-16;-0.12 -0.225 -1.11022302462516e-16],'MeshFaces',[6 2 1;1 5 6;8 4 3;3 7 8;6 7 3;3 2 6;5 1 4;4 8 5;4 1 2;2 3 4;7 6 5;5 8 7],'RCSPattern',[-8 -8;-8 -8],'RCSAzimuthAngles',[-180 180],'RCSElevationAngles',[-90 90]); struct('ActorID',28,'ClassID',3,'Length',1.7,'Width',0.45,'Height',1.7,'OriginOffset',[0 0 0],'MeshVertices',[0.85 -0.225 1.7;0.85 0.225 1.7;-0.85 0.225 1.7;-0.85 -0.225 1.7;0.85 -0.225 -1.11022302462516e-16;0.85 0.225 -1.11022302462516e-16;-0.85 0.225 -1.11022302462516e-16;-0.85 -0.225 -1.11022302462516e-16],'MeshFaces',[6 2 1;1 5 6;8 4 3;3 7 8;6 7 3;3 2 6;5 1 4;4 8 5;4 1 2;2 3 4;7 6 5;5 8 7],'RCSPattern',[10 10;10 10],'RCSAzimuthAngles',[-180 180],'RCSElevationAngles',[-90 90]); struct('ActorID',29,'ClassID',4,'Length',0.24,'Width',0.45,'Height',1.7,'OriginOffset',[0 0 0],'MeshVertices',[0.12 -0.225 1.7;0.12 0.225 1.7;-0.12 0.225 1.7;-0.12 -0.225 1.7;0.12 -0.225 -1.11022302462516e-16;0.12 0.225 -1.11022302462516e-16;-0.12 0.225 -1.11022302462516e-16;-0.12 -0.225 -1.11022302462516e-16],'MeshFaces',[6 2 1;1 5 6;8 4 3;3 7 8;6 7 3;3 2 6;5 1 4;4 8 5;4 1 2;2 3 4;7 6 5;5 8 7],'RCSPattern',[-8 -8;-8 -8],'RCSAzimuthAngles',[-180 180],'RCSElevationAngles',[-90 90])]  Intrinsics=driving.internal.cameraIntrinsics('FocalLength',[320 320],'PrincipalPoint',[320 240],'ImageSize',[480 640],'RadialDistortion',[0 0],'TangentialDistortion',[0 0],'Skew',0)
  Camera4 : drivingscenarioandsensors/Vision Detection Generator  SensorIndex=10  DetectorOutput=Objects only  UpdateInterval=0.1  LaneUpdateInterval=0.1  SensorLocation=[3.7 0]  Height=1.1  Yaw=-62.9424470891587  Pitch=1  Roll=0  BusNameSource=Auto  BusName=BusObjectDetections  BusName2Source=Auto  BusName2=BusLaneDetections  MaxNumDetectionsSource=Property  MaxNumDetections=50  MaxNumLanesSource=Property  MaxNumLanes=30  DetectionCoordinates=Ego Cartesian  SimulateUsing=Interpreted execution  MaxRange=10  BoundingBoxAccuracy=5  ProcessNoiseIntensity=5  MaxSpeed=50  MaxAllowedOcclusion=0.5  MinObjectImageSize=[15 15]  DetectionProbability=0.2  FalsePositivesPerImage=0.1  MinLaneImageSize=[20 3]  LaneBoundaryAccuracy=3  HasNoise=on  InitialSeedSource=Repeatable  InitialSeed=0  UsedSeed=0  ActorProfilesSource=MATLAB expression  ActorProfilesParameters=driving.internal.ActorProfilesParameters  ActorProfilesExpression=[struct('ActorID',1,'ClassID',1,'Length',4.7,'Width',1.8,'Height',1.4,'OriginOffset',[-1.35 0 0],'MeshVertices',[3.7 -0.9 1.4;3.7 0.9 1.4;-1 0.9 1.4;-1 -0.9 1.4;3.7 -0.9 0;3.7 0.9 0;-1 0.9 0;-1 -0.9 0],'MeshFaces',[6 2 1;1 5 6;8 4 3;3 7 8;6 7 3;3 2 6;5 1 4;4 8 5;4 1 2;2 3 4;7 6 5;5 8 7],'RCSPattern',[10 10;10 10],'RCSAzimuthAngles',[-180 180],'RCSElevationAngles',[-90 90]); struct('ActorID',2,'ClassID',1,'Length',4.7,'Width',1.8,'Height',1.4,'OriginOffset',[-1.35 0 0],'MeshVertices',[3.7 -0.9 1.4;3.7 0.9 1.4;-1 0.9 1.4;-1 -0.9 1.4;3.7 -0.9 0;3.7 0.9 0;-1 0.9 0;-1 -0.9 0],'MeshFaces',[6 2 1;1 5 6;8 4 3;3 7 8;6 7 3;3 2 6;5 1 4;4 8 5;4 1 2;2 3 4;7 6 5;5 8 7],'RCSPattern',[10 10;10 10],'RCSAzimuthAngles',[-180 180],'RCSElevationAngles',[-90 90]); struct('ActorID',3,'ClassID',1,'Length',4.7,'Width',1.8,'Height',1.4,'OriginOffset',[-1.35 0 0],'MeshVertices',[3.7 -0.9 1.4;3.7 0.9 1.4;-1 0.9 1.4;-1 -0.9 1.4;3.7 -0.9 0;3.7 0.9 0;-1 0.9 0;-1 -0.9 0],'MeshFaces',[6 2 1;1 5 6;8 4 3;3 7 8;6 7 3;3 2 6;5 1 4;4 8 5;4 1 2;2 3 4;7 6 5;5 8 7],'RCSPattern',[10 10;10 10],'RCSAzimuthAngles',[-180 180],'RCSElevationAngles',[-90 90]); struct('ActorID',4,'ClassID',1,'Length',4.7,'Width',1.8,'Height',1.4,'OriginOffset',[-1.35 0 0],'MeshVertices',[3.7 -0.9 1.4;3.7 0.9 1.4;-1 0.9 1.4;-1 -0.9 1.4;3.7 -0.9 0;3.7 0.9 0;-1 0.9 0;-1 -0.9 0],'MeshFaces',[6 2 1;1 5 6;8 4 3;3 7 8;6 7 3;3 2 6;5 1 4;4 8 5;4 1 2;2 3 4;7 6 5;5 8 7],'RCSPattern',[10 10;10 10],'RCSAzimuthAngles',[-180 180],'RCSElevationAngles',[-90 90]); struct('ActorID',5,'ClassID',1,'Length',4.7,'Width',1.8,'Height',1.4,'OriginOffset',[-1.35 0 0],'MeshVertices',[3.7 -0.9 1.4;3.7 0.9 1.4;-1 0.9 1.4;-1 -0.9 1.4;3.7 -0.9 0;3.7 0.9 0;-1 0.9 0;-1 -0.9 0],'MeshFaces',[6 2 1;1 5 6;8 4 3;3 7 8;6 7 3;3 2 6;5 1 4;4 8 5;4 1 2;2 3 4;7 6 5;5 8 7],'RCSPattern',[10 10;10 10],'RCSAzimuthAngles',[-180 180],'RCSElevationAngles',[-90 90]); struct('ActorID',6,'ClassID',4,'Length',0.24,'Width',0.45,'Height',1.7,'OriginOffset',[0 0 0],'MeshVertices',[0.12 -0.225 1.7;0.12 0.225 1.7;-0.12 0.225 1.7;-0.12 -0.225 1.7;0.12 -0.225 -1.11022302462516e-16;0.12 0.225 -1.11022302462516e-16;-0.12 0.225 -1.11022302462516e-16;-0.12 -0.225 -1.11022302462516e-16],'MeshFaces',[6 2 1;1 5 6;8 4 3;3 7 8;6 7 3;3 2 6;5 1 4;4 8 5;4 1 2;2 3 4;7 6 5;5 8 7],'RCSPattern',[-8 -8;-8 -8],'RCSAzimuthAngles',[-180 180],'RCSElevationAngles',[-90 90]); struct('ActorID',7,'ClassID',4,'Length',0.24,'Width',0.45,'Height',1.7,'OriginOffset',[0 0 0],'MeshVertices',[0.12 -0.225 1.7;0.12 0.225 1.7;-0.12 0.225 1.7;-0.12 -0.225 1.7;0.12 -0.225 -1.11022302462516e-16;0.12 0.225 -1.11022302462516e-16;-0.12 0.225 -1.11022302462516e-16;-0.12 -0.225 -1.11022302462516e-16],'MeshFaces',[6 2 1;1 5 6;8 4 3;3 7 8;6 7 3;3 2 6;5 1 4;4 8 5;4 1 2;2 3 4;7 6 5;5 8 7],'RCSPattern',[-8 -8;-8 -8],'RCSAzimuthAngles',[-180 180],'RCSElevationAngles',[-90 90]); struct('ActorID',8,'ClassID',4,'Length',0.24,'Width',0.45,'Height',1.7,'OriginOffset',[0 0 0],'MeshVertices',[0.12 -0.225 1.7;0.12 0.225 1.7;-0.12 0.225 1.7;-0.12 -0.225 1.7;0.12 -0.225 -1.11022302462516e-16;0.12 0.225 -1.11022302462516e-16;-0.12 0.225 -1.11022302462516e-16;-0.12 -0.225 -1.11022302462516e-16],'MeshFaces',[6 2 1;1 5 6;8 4 3;3 7 8;6 7 3;3 2 6;5 1 4;4 8 5;4 1 2;2 3 4;7 6 5;5 8 7],'RCSPattern',[-8 -8;-8 -8],'RCSAzimuthAngles',[-180 180],'RCSElevationAngles',[-90 90]); struct('ActorID',9,'ClassID',4,'Length',0.24,'Width',0.45,'Height',1.7,'OriginOffset',[0 0 0],'MeshVertices',[0.12 -0.225 1.7;0.12 0.225 1.7;-0.12 0.225 1.7;-0.12 -0.225 1.7;0.12 -0.225 -1.11022302462516e-16;0.12 0.225 -1.11022302462516e-16;-0.12 0.225 -1.11022302462516e-16;-0.12 -0.225 -1.11022302462516e-16],'MeshFaces',[6 2 1;1 5 6;8 4 3;3 7 8;6 7 3;3 2 6;5 1 4;4 8 5;4 1 2;2 3 4;7 6 5;5 8 7],'RCSPattern',[-8 -8;-8 -8],'RCSAzimuthAngles',[-180 180],'RCSElevationAngles',[-90 90]); struct('ActorID',10,'ClassID',4,'Length',0.24,'Width',0.45,'Height',1.7,'OriginOffset',[0 0 0],'MeshVertices',[0.12 -0.225 1.7;0.12 0.225 1.7;-0.12 0.225 1.7;-0.12 -0.225 1.7;0.12 -0.225 -1.11022302462516e-16;0.12 0.225 -1.11022302462516e-16;-0.12 0.225 -1.11022302462516e-16;-0.12 -0.225 -1.11022302462516e-16],'MeshFaces',[6 2 1;1 5 6;8 4 3;3 7 8;6 7 3;3 2 6;5 1 4;4 8 5;4 1 2;2 3 4;7 6 5;5 8 7],'RCSPattern',[-8 -8;-8 -8],'RCSAzimuthAngles',[-180 180],'RCSElevationAngles',[-90 90]); struct('ActorID',11,'ClassID',4,'Length',0.24,'Width',0.45,'Height',1.7,'OriginOffset',[0 0 0],'MeshVertices',[0.12 -0.225 1.7;0.12 0.225 1.7;-0.12 0.225 1.7;-0.12 -0.225 1.7;0.12 -0.225 -1.11022302462516e-16;0.12 0.225 -1.11022302462516e-16;-0.12 0.225 -1.11022302462516e-16;-0.12 -0.225 -1.11022302462516e-16],'MeshFaces',[6 2 1;1 5 6;8 4 3;3 7 8;6 7 3;3 2 6;5 1 4;4 8 5;4 1 2;2 3 4;7 6 5;5 8 7],'RCSPattern',[-8 -8;-8 -8],'RCSAzimuthAngles',[-180 180],'RCSElevationAngles',[-90 90]); struct('ActorID',12,'ClassID',4,'Length',0.24,'Width',0.45,'Height',1.7,'OriginOffset',[0 0 0],'MeshVertices',[0.12 -0.225 1.7;0.12 0.225 1.7;-0.12 0.225 1.7;-0.12 -0.225 1.7;0.12 -0.225 -1.11022302462516e-16;0.12 0.225 -1.11022302462516e-16;-0.12 0.225 -1.11022302462516e-16;-0.12 -0.225 -1.11022302462516e-16],'MeshFaces',[6 2 1;1 5 6;8 4 3;3 7 8;6 7 3;3 2 6;5 1 4;4 8 5;4 1 2;2 3 4;7 6 5;5 8 7],'RCSPattern',[-8 -8;-8 -8],'RCSAzimuthAngles',[-180 180],'RCSElevationAngles',[-90 90]); struct('ActorID',13,'ClassID',4,'Length',0.24,'Width',0.45,'Height',1.7,'OriginOffset',[0 0 0],'MeshVertices',[0.12 -0.225 1.7;0.12 0.225 1.7;-0.12 0.225 1.7;-0.12 -0.225 1.7;0.12 -0.225 -1.11022302462516e-16;0.12 0.225 -1.11022302462516e-16;-0.12 0.225 -1.11022302462516e-16;-0.12 -0.225 -1.11022302462516e-16],'MeshFaces',[6 2 1;1 5 6;8 4 3;3 7 8;6 7 3;3 2 6;5 1 4;4 8 5;4 1 2;2 3 4;7 6 5;5 8 7],'RCSPattern',[-8 -8;-8 -8],'RCSAzimuthAngles',[-180 180],'RCSElevationAngles',[-90 90]); struct('ActorID',14,'ClassID',4,'Length',0.24,'Width',0.45,'Height',1.7,'OriginOffset',[0 0 0],'MeshVertices',[0.12 -0.225 1.7;0.12 0.225 1.7;-0.12 0.225 1.7;-0.12 -0.225 1.7;0.12 -0.225 -1.11022302462516e-16;0.12 0.225 -1.11022302462516e-16;-0.12 0.225 -1.11022302462516e-16;-0.12 -0.225 -1.11022302462516e-16],'MeshFaces',[6 2 1;1 5 6;8 4 3;3 7 8;6 7 3;3 2 6;5 1 4;4 8 5;4 1 2;2 3 4;7 6 5;5 8 7],'RCSPattern',[-8 -8;-8 -8],'RCSAzimuthAngles',[-180 180],'RCSElevationAngles',[-90 90]); struct('ActorID',15,'ClassID',4,'Length',0.24,'Width',0.45,'Height',1.7,'OriginOffset',[0 0 0],'MeshVertices',[0.12 -0.225 1.7;0.12 0.225 1.7;-0.12 0.225 1.7;-0.12 -0.225 1.7;0.12 -0.225 -1.11022302462516e-16;0.12 0.225 -1.11022302462516e-16;-0.12 0.225 -1.11022302462516e-16;-0.12 -0.225 -1.11022302462516e-16],'MeshFaces',[6 2 1;1 5 6;8 4 3;3 7 8;6 7 3;3 2 6;5 1 4;4 8 5;4 1 2;2 3 4;7 6 5;5 8 7],'RCSPattern',[-8 -8;-8 -8],'RCSAzimuthAngles',[-180 180],'RCSElevationAngles',[-90 90]); struct('ActorID',16,'ClassID',4,'Length',0.24,'Width',0.45,'Height',1.7,'OriginOffset',[0 0 0],'MeshVertices',[0.12 -0.225 1.7;0.12 0.225 1.7;-0.12 0.225 1.7;-0.12 -0.225 1.7;0.12 -0.225 -1.11022302462516e-16;0.12 0.225 -1.11022302462516e-16;-0.12 0.225 -1.11022302462516e-16;-0.12 -0.225 -1.11022302462516e-16],'MeshFaces',[6 2 1;1 5 6;8 4 3;3 7 8;6 7 3;3 2 6;5 1 4;4 8 5;4 1 2;2 3 4;7 6 5;5 8 7],'RCSPattern',[-8 -8;-8 -8],'RCSAzimuthAngles',[-180 180],'RCSElevationAngles',[-90 90]); struct('ActorID',17,'ClassID',4,'Length',0.24,'Width',0.45,'Height',1.7,'OriginOffset',[0 0 0],'MeshVertices',[0.12 -0.225 1.7;0.12 0.225 1.7;-0.12 0.225 1.7;-0.12 -0.225 1.7;0.12 -0.225 -1.11022302462516e-16;0.12 0.225 -1.11022302462516e-16;-0.12 0.225 -1.11022302462516e-16;-0.12 -0.225 -1.11022302462516e-16],'MeshFaces',[6 2 1;1 5 6;8 4 3;3 7 8;6 7 3;3 2 6;5 1 4;4 8 5;4 1 2;2 3 4;7 6 5;5 8 7],'RCSPattern',[-8 -8;-8 -8],'RCSAzimuthAngles',[-180 180],'RCSElevationAngles',[-90 90]); struct('ActorID',18,'ClassID',4,'Length',0.24,'Width',0.45,'Height',1.7,'OriginOffset',[0 0 0],'MeshVertices',[0.12 -0.225 1.7;0.12 0.225 1.7;-0.12 0.225 1.7;-0.12 -0.225 1.7;0.12 -0.225 -1.11022302462516e-16;0.12 0.225 -1.11022302462516e-16;-0.12 0.225 -1.11022302462516e-16;-0.12 -0.225 -1.11022302462516e-16],'MeshFaces',[6 2 1;1 5 6;8 4 3;3 7 8;6 7 3;3 2 6;5 1 4;4 8 5;4 1 2;2 3 4;7 6 5;5 8 7],'RCSPattern',[-8 -8;-8 -8],'RCSAzimuthAngles',[-180 180],'RCSElevationAngles',[-90 90]); struct('ActorID',19,'ClassID',4,'Length',0.24,'Width',0.45,'Height',1.7,'OriginOffset',[0 0 0],'MeshVertices',[0.12 -0.225 1.7;0.12 0.225 1.7;-0.12 0.225 1.7;-0.12 -0.225 1.7;0.12 -0.225 -1.11022302462516e-16;0.12 0.225 -1.11022302462516e-16;-0.12 0.225 -1.11022302462516e-16;-0.12 -0.225 -1.11022302462516e-16],'MeshFaces',[6 2 1;1 5 6;8 4 3;3 7 8;6 7 3;3 2 6;5 1 4;4 8 5;4 1 2;2 3 4;7 6 5;5 8 7],'RCSPattern',[-8 -8;-8 -8],'RCSAzimuthAngles',[-180 180],'RCSElevationAngles',[-90 90]); struct('ActorID',20,'ClassID',4,'Length',0.24,'Width',0.45,'Height',1.7,'OriginOffset',[0 0 0],'MeshVertices',[0.12 -0.225 1.7;0.12 0.225 1.7;-0.12 0.225 1.7;-0.12 -0.225 1.7;0.12 -0.225 -1.11022302462516e-16;0.12 0.225 -1.11022302462516e-16;-0.12 0.225 -1.11022302462516e-16;-0.12 -0.225 -1.11022302462516e-16],'MeshFaces',[6 2 1;1 5 6;8 4 3;3 7 8;6 7 3;3 2 6;5 1 4;4 8 5;4 1 2;2 3 4;7 6 5;5 8 7],'RCSPattern',[-8 -8;-8 -8],'RCSAzimuthAngles',[-180 180],'RCSElevationAngles',[-90 90]); struct('ActorID',21,'ClassID',4,'Length',0.24,'Width',0.45,'Height',1.7,'OriginOffset',[0 0 0],'MeshVertices',[0.12 -0.225 1.7;0.12 0.225 1.7;-0.12 0.225 1.7;-0.12 -0.225 1.7;0.12 -0.225 -1.11022302462516e-16;0.12 0.225 -1.11022302462516e-16;-0.12 0.225 -1.11022302462516e-16;-0.12 -0.225 -1.11022302462516e-16],'MeshFaces',[6 2 1;1 5 6;8 4 3;3 7 8;6 7 3;3 2 6;5 1 4;4 8 5;4 1 2;2 3 4;7 6 5;5 8 7],'RCSPattern',[-8 -8;-8 -8],'RCSAzimuthAngles',[-180 180],'RCSElevationAngles',[-90 90]); struct('ActorID',22,'ClassID',4,'Length',0.24,'Width',0.45,'Height',1.7,'OriginOffset',[0 0 0],'MeshVertices',[0.12 -0.225 1.7;0.12 0.225 1.7;-0.12 0.225 1.7;-0.12 -0.225 1.7;0.12 -0.225 -1.11022302462516e-16;0.12 0.225 -1.11022302462516e-16;-0.12 0.225 -1.11022302462516e-16;-0.12 -0.225 -1.11022302462516e-16],'MeshFaces',[6 2 1;1 5 6;8 4 3;3 7 8;6 7 3;3 2 6;5 1 4;4 8 5;4 1 2;2 3 4;7 6 5;5 8 7],'RCSPattern',[-8 -8;-8 -8],'RCSAzimuthAngles',[-180 180],'RCSElevationAngles',[-90 90]); struct('ActorID',23,'ClassID',4,'Length',0.24,'Width',0.45,'Height',1.7,'OriginOffset',[0 0 0],'MeshVertices',[0.12 -0.225 1.7;0.12 0.225 1.7;-0.12 0.225 1.7;-0.12 -0.225 1.7;0.12 -0.225 -1.11022302462516e-16;0.12 0.225 -1.11022302462516e-16;-0.12 0.225 -1.11022302462516e-16;-0.12 -0.225 -1.11022302462516e-16],'MeshFaces',[6 2 1;1 5 6;8 4 3;3 7 8;6 7 3;3 2 6;5 1 4;4 8 5;4 1 2;2 3 4;7 6 5;5 8 7],'RCSPattern',[-8 -8;-8 -8],'RCSAzimuthAngles',[-180 180],'RCSElevationAngles',[-90 90]); struct('ActorID',24,'ClassID',4,'Length',0.24,'Width',0.45,'Height',1.7,'OriginOffset',[0 0 0],'MeshVertices',[0.12 -0.225 1.7;0.12 0.225 1.7;-0.12 0.225 1.7;-0.12 -0.225 1.7;0.12 -0.225 -1.11022302462516e-16;0.12 0.225 -1.11022302462516e-16;-0.12 0.225 -1.11022302462516e-16;-0.12 -0.225 -1.11022302462516e-16],'MeshFaces',[6 2 1;1 5 6;8 4 3;3 7 8;6 7 3;3 2 6;5 1 4;4 8 5;4 1 2;2 3 4;7 6 5;5 8 7],'RCSPattern',[-8 -8;-8 -8],'RCSAzimuthAngles',[-180 180],'RCSElevationAngles',[-90 90]); struct('ActorID',25,'ClassID',4,'Length',0.24,'Width',0.45,'Height',1.7,'OriginOffset',[0 0 0],'MeshVertices',[0.12 -0.225 1.7;0.12 0.225 1.7;-0.12 0.225 1.7;-0.12 -0.225 1.7;0.12 -0.225 -1.11022302462516e-16;0.12 0.225 -1.11022302462516e-16;-0.12 0.225 -1.11022302462516e-16;-0.12 -0.225 -1.11022302462516e-16],'MeshFaces',[6 2 1;1 5 6;8 4 3;3 7 8;6 7 3;3 2 6;5 1 4;4 8 5;4 1 2;2 3 4;7 6 5;5 8 7],'RCSPattern',[-8 -8;-8 -8],'RCSAzimuthAngles',[-180 180],'RCSElevationAngles',[-90 90]); struct('ActorID',26,'ClassID',4,'Length',0.24,'Width',0.45,'Height',1.7,'OriginOffset',[0 0 0],'MeshVertices',[0.12 -0.225 1.7;0.12 0.225 1.7;-0.12 0.225 1.7;-0.12 -0.225 1.7;0.12 -0.225 -1.11022302462516e-16;0.12 0.225 -1.11022302462516e-16;-0.12 0.225 -1.11022302462516e-16;-0.12 -0.225 -1.11022302462516e-16],'MeshFaces',[6 2 1;1 5 6;8 4 3;3 7 8;6 7 3;3 2 6;5 1 4;4 8 5;4 1 2;2 3 4;7 6 5;5 8 7],'RCSPattern',[-8 -8;-8 -8],'RCSAzimuthAngles',[-180 180],'RCSElevationAngles',[-90 90]); struct('ActorID',27,'ClassID',4,'Length',0.24,'Width',0.45,'Height',1.7,'OriginOffset',[0 0 0],'MeshVertices',[0.12 -0.225 1.7;0.12 0.225 1.7;-0.12 0.225 1.7;-0.12 -0.225 1.7;0.12 -0.225 -1.11022302462516e-16;0.12 0.225 -1.11022302462516e-16;-0.12 0.225 -1.11022302462516e-16;-0.12 -0.225 -1.11022302462516e-16],'MeshFaces',[6 2 1;1 5 6;8 4 3;3 7 8;6 7 3;3 2 6;5 1 4;4 8 5;4 1 2;2 3 4;7 6 5;5 8 7],'RCSPattern',[-8 -8;-8 -8],'RCSAzimuthAngles',[-180 180],'RCSElevationAngles',[-90 90]); struct('ActorID',28,'ClassID',3,'Length',1.7,'Width',0.45,'Height',1.7,'OriginOffset',[0 0 0],'MeshVertices',[0.85 -0.225 1.7;0.85 0.225 1.7;-0.85 0.225 1.7;-0.85 -0.225 1.7;0.85 -0.225 -1.11022302462516e-16;0.85 0.225 -1.11022302462516e-16;-0.85 0.225 -1.11022302462516e-16;-0.85 -0.225 -1.11022302462516e-16],'MeshFaces',[6 2 1;1 5 6;8 4 3;3 7 8;6 7 3;3 2 6;5 1 4;4 8 5;4 1 2;2 3 4;7 6 5;5 8 7],'RCSPattern',[10 10;10 10],'RCSAzimuthAngles',[-180 180],'RCSElevationAngles',[-90 90]); struct('ActorID',29,'ClassID',4,'Length',0.24,'Width',0.45,'Height',1.7,'OriginOffset',[0 0 0],'MeshVertices',[0.12 -0.225 1.7;0.12 0.225 1.7;-0.12 0.225 1.7;-0.12 -0.225 1.7;0.12 -0.225 -1.11022302462516e-16;0.12 0.225 -1.11022302462516e-16;-0.12 0.225 -1.11022302462516e-16;-0.12 -0.225 -1.11022302462516e-16],'MeshFaces',[6 2 1;1 5 6;8 4 3;3 7 8;6 7 3;3 2 6;5 1 4;4 8 5;4 1 2;2 3 4;7 6 5;5 8 7],'RCSPattern',[-8 -8;-8 -8],'RCSAzimuthAngles',[-180 180],'RCSElevationAngles',[-90 90])]  Intrinsics=driving.internal.cameraIntrinsics('FocalLength',[320 320],'PrincipalPoint',[320 240],'ImageSize',[480 640],'RadialDistortion',[0 0],'TangentialDistortion',[0 0],'Skew',0)
  Camera5 : drivingscenarioandsensors/Vision Detection Generator  SensorIndex=11  DetectorOutput=Objects only  UpdateInterval=0.1  LaneUpdateInterval=0.1  SensorLocation=[0 0]  Height=1.1  Yaw=-180  Pitch=1  Roll=0  BusNameSource=Auto  BusName=BusObjectDetections  BusName2Source=Auto  BusName2=BusLaneDetections  MaxNumDetectionsSource=Property  MaxNumDetections=50  MaxNumLanesSource=Property  MaxNumLanes=30  DetectionCoordinates=Ego Cartesian  SimulateUsing=Interpreted execution  MaxRange=10  BoundingBoxAccuracy=5  ProcessNoiseIntensity=5  MaxSpeed=50  MaxAllowedOcclusion=0.5  MinObjectImageSize=[15 15]  DetectionProbability=0.2  FalsePositivesPerImage=0.1  MinLaneImageSize=[20 3]  LaneBoundaryAccuracy=3  HasNoise=on  InitialSeedSource=Repeatable  InitialSeed=0  UsedSeed=0  ActorProfilesSource=MATLAB expression  ActorProfilesParameters=driving.internal.ActorProfilesParameters  ActorProfilesExpression=[struct('ActorID',1,'ClassID',1,'Length',4.7,'Width',1.8,'Height',1.4,'OriginOffset',[-1.35 0 0],'MeshVertices',[3.7 -0.9 1.4;3.7 0.9 1.4;-1 0.9 1.4;-1 -0.9 1.4;3.7 -0.9 0;3.7 0.9 0;-1 0.9 0;-1 -0.9 0],'MeshFaces',[6 2 1;1 5 6;8 4 3;3 7 8;6 7 3;3 2 6;5 1 4;4 8 5;4 1 2;2 3 4;7 6 5;5 8 7],'RCSPattern',[10 10;10 10],'RCSAzimuthAngles',[-180 180],'RCSElevationAngles',[-90 90]); struct('ActorID',2,'ClassID',1,'Length',4.7,'Width',1.8,'Height',1.4,'OriginOffset',[-1.35 0 0],'MeshVertices',[3.7 -0.9 1.4;3.7 0.9 1.4;-1 0.9 1.4;-1 -0.9 1.4;3.7 -0.9 0;3.7 0.9 0;-1 0.9 0;-1 -0.9 0],'MeshFaces',[6 2 1;1 5 6;8 4 3;3 7 8;6 7 3;3 2 6;5 1 4;4 8 5;4 1 2;2 3 4;7 6 5;5 8 7],'RCSPattern',[10 10;10 10],'RCSAzimuthAngles',[-180 180],'RCSElevationAngles',[-90 90]); struct('ActorID',3,'ClassID',1,'Length',4.7,'Width',1.8,'Height',1.4,'OriginOffset',[-1.35 0 0],'MeshVertices',[3.7 -0.9 1.4;3.7 0.9 1.4;-1 0.9 1.4;-1 -0.9 1.4;3.7 -0.9 0;3.7 0.9 0;-1 0.9 0;-1 -0.9 0],'MeshFaces',[6 2 1;1 5 6;8 4 3;3 7 8;6 7 3;3 2 6;5 1 4;4 8 5;4 1 2;2 3 4;7 6 5;5 8 7],'RCSPattern',[10 10;10 10],'RCSAzimuthAngles',[-180 180],'RCSElevationAngles',[-90 90]); struct('ActorID',4,'ClassID',1,'Length',4.7,'Width',1.8,'Height',1.4,'OriginOffset',[-1.35 0 0],'MeshVertices',[3.7 -0.9 1.4;3.7 0.9 1.4;-1 0.9 1.4;-1 -0.9 1.4;3.7 -0.9 0;3.7 0.9 0;-1 0.9 0;-1 -0.9 0],'MeshFaces',[6 2 1;1 5 6;8 4 3;3 7 8;6 7 3;3 2 6;5 1 4;4 8 5;4 1 2;2 3 4;7 6 5;5 8 7],'RCSPattern',[10 10;10 10],'RCSAzimuthAngles',[-180 180],'RCSElevationAngles',[-90 90]); struct('ActorID',5,'ClassID',1,'Length',4.7,'Width',1.8,'Height',1.4,'OriginOffset',[-1.35 0 0],'MeshVertices',[3.7 -0.9 1.4;3.7 0.9 1.4;-1 0.9 1.4;-1 -0.9 1.4;3.7 -0.9 0;3.7 0.9 0;-1 0.9 0;-1 -0.9 0],'MeshFaces',[6 2 1;1 5 6;8 4 3;3 7 8;6 7 3;3 2 6;5 1 4;4 8 5;4 1 2;2 3 4;7 6 5;5 8 7],'RCSPattern',[10 10;10 10],'RCSAzimuthAngles',[-180 180],'RCSElevationAngles',[-90 90]); struct('ActorID',6,'ClassID',4,'Length',0.24,'Width',0.45,'Height',1.7,'OriginOffset',[0 0 0],'MeshVertices',[0.12 -0.225 1.7;0.12 0.225 1.7;-0.12 0.225 1.7;-0.12 -0.225 1.7;0.12 -0.225 -1.11022302462516e-16;0.12 0.225 -1.11022302462516e-16;-0.12 0.225 -1.11022302462516e-16;-0.12 -0.225 -1.11022302462516e-16],'MeshFaces',[6 2 1;1 5 6;8 4 3;3 7 8;6 7 3;3 2 6;5 1 4;4 8 5;4 1 2;2 3 4;7 6 5;5 8 7],'RCSPattern',[-8 -8;-8 -8],'RCSAzimuthAngles',[-180 180],'RCSElevationAngles',[-90 90]); struct('ActorID',7,'ClassID',4,'Length',0.24,'Width',0.45,'Height',1.7,'OriginOffset',[0 0 0],'MeshVertices',[0.12 -0.225 1.7;0.12 0.225 1.7;-0.12 0.225 1.7;-0.12 -0.225 1.7;0.12 -0.225 -1.11022302462516e-16;0.12 0.225 -1.11022302462516e-16;-0.12 0.225 -1.11022302462516e-16;-0.12 -0.225 -1.11022302462516e-16],'MeshFaces',[6 2 1;1 5 6;8 4 3;3 7 8;6 7 3;3 2 6;5 1 4;4 8 5;4 1 2;2 3 4;7 6 5;5 8 7],'RCSPattern',[-8 -8;-8 -8],'RCSAzimuthAngles',[-180 180],'RCSElevationAngles',[-90 90]); struct('ActorID',8,'ClassID',4,'Length',0.24,'Width',0.45,'Height',1.7,'OriginOffset',[0 0 0],'MeshVertices',[0.12 -0.225 1.7;0.12 0.225 1.7;-0.12 0.225 1.7;-0.12 -0.225 1.7;0.12 -0.225 -1.11022302462516e-16;0.12 0.225 -1.11022302462516e-16;-0.12 0.225 -1.11022302462516e-16;-0.12 -0.225 -1.11022302462516e-16],'MeshFaces',[6 2 1;1 5 6;8 4 3;3 7 8;6 7 3;3 2 6;5 1 4;4 8 5;4 1 2;2 3 4;7 6 5;5 8 7],'RCSPattern',[-8 -8;-8 -8],'RCSAzimuthAngles',[-180 180],'RCSElevationAngles',[-90 90]); struct('ActorID',9,'ClassID',4,'Length',0.24,'Width',0.45,'Height',1.7,'OriginOffset',[0 0 0],'MeshVertices',[0.12 -0.225 1.7;0.12 0.225 1.7;-0.12 0.225 1.7;-0.12 -0.225 1.7;0.12 -0.225 -1.11022302462516e-16;0.12 0.225 -1.11022302462516e-16;-0.12 0.225 -1.11022302462516e-16;-0.12 -0.225 -1.11022302462516e-16],'MeshFaces',[6 2 1;1 5 6;8 4 3;3 7 8;6 7 3;3 2 6;5 1 4;4 8 5;4 1 2;2 3 4;7 6 5;5 8 7],'RCSPattern',[-8 -8;-8 -8],'RCSAzimuthAngles',[-180 180],'RCSElevationAngles',[-90 90]); struct('ActorID',10,'ClassID',4,'Length',0.24,'Width',0.45,'Height',1.7,'OriginOffset',[0 0 0],'MeshVertices',[0.12 -0.225 1.7;0.12 0.225 1.7;-0.12 0.225 1.7;-0.12 -0.225 1.7;0.12 -0.225 -1.11022302462516e-16;0.12 0.225 -1.11022302462516e-16;-0.12 0.225 -1.11022302462516e-16;-0.12 -0.225 -1.11022302462516e-16],'MeshFaces',[6 2 1;1 5 6;8 4 3;3 7 8;6 7 3;3 2 6;5 1 4;4 8 5;4 1 2;2 3 4;7 6 5;5 8 7],'RCSPattern',[-8 -8;-8 -8],'RCSAzimuthAngles',[-180 180],'RCSElevationAngles',[-90 90]); struct('ActorID',11,'ClassID',4,'Length',0.24,'Width',0.45,'Height',1.7,'OriginOffset',[0 0 0],'MeshVertices',[0.12 -0.225 1.7;0.12 0.225 1.7;-0.12 0.225 1.7;-0.12 -0.225 1.7;0.12 -0.225 -1.11022302462516e-16;0.12 0.225 -1.11022302462516e-16;-0.12 0.225 -1.11022302462516e-16;-0.12 -0.225 -1.11022302462516e-16],'MeshFaces',[6 2 1;1 5 6;8 4 3;3 7 8;6 7 3;3 2 6;5 1 4;4 8 5;4 1 2;2 3 4;7 6 5;5 8 7],'RCSPattern',[-8 -8;-8 -8],'RCSAzimuthAngles',[-180 180],'RCSElevationAngles',[-90 90]); struct('ActorID',12,'ClassID',4,'Length',0.24,'Width',0.45,'Height',1.7,'OriginOffset',[0 0 0],'MeshVertices',[0.12 -0.225 1.7;0.12 0.225 1.7;-0.12 0.225 1.7;-0.12 -0.225 1.7;0.12 -0.225 -1.11022302462516e-16;0.12 0.225 -1.11022302462516e-16;-0.12 0.225 -1.11022302462516e-16;-0.12 -0.225 -1.11022302462516e-16],'MeshFaces',[6 2 1;1 5 6;8 4 3;3 7 8;6 7 3;3 2 6;5 1 4;4 8 5;4 1 2;2 3 4;7 6 5;5 8 7],'RCSPattern',[-8 -8;-8 -8],'RCSAzimuthAngles',[-180 180],'RCSElevationAngles',[-90 90]); struct('ActorID',13,'ClassID',4,'Length',0.24,'Width',0.45,'Height',1.7,'OriginOffset',[0 0 0],'MeshVertices',[0.12 -0.225 1.7;0.12 0.225 1.7;-0.12 0.225 1.7;-0.12 -0.225 1.7;0.12 -0.225 -1.11022302462516e-16;0.12 0.225 -1.11022302462516e-16;-0.12 0.225 -1.11022302462516e-16;-0.12 -0.225 -1.11022302462516e-16],'MeshFaces',[6 2 1;1 5 6;8 4 3;3 7 8;6 7 3;3 2 6;5 1 4;4 8 5;4 1 2;2 3 4;7 6 5;5 8 7],'RCSPattern',[-8 -8;-8 -8],'RCSAzimuthAngles',[-180 180],'RCSElevationAngles',[-90 90]); struct('ActorID',14,'ClassID',4,'Length',0.24,'Width',0.45,'Height',1.7,'OriginOffset',[0 0 0],'MeshVertices',[0.12 -0.225 1.7;0.12 0.225 1.7;-0.12 0.225 1.7;-0.12 -0.225 1.7;0.12 -0.225 -1.11022302462516e-16;0.12 0.225 -1.11022302462516e-16;-0.12 0.225 -1.11022302462516e-16;-0.12 -0.225 -1.11022302462516e-16],'MeshFaces',[6 2 1;1 5 6;8 4 3;3 7 8;6 7 3;3 2 6;5 1 4;4 8 5;4 1 2;2 3 4;7 6 5;5 8 7],'RCSPattern',[-8 -8;-8 -8],'RCSAzimuthAngles',[-180 180],'RCSElevationAngles',[-90 90]); struct('ActorID',15,'ClassID',4,'Length',0.24,'Width',0.45,'Height',1.7,'OriginOffset',[0 0 0],'MeshVertices',[0.12 -0.225 1.7;0.12 0.225 1.7;-0.12 0.225 1.7;-0.12 -0.225 1.7;0.12 -0.225 -1.11022302462516e-16;0.12 0.225 -1.11022302462516e-16;-0.12 0.225 -1.11022302462516e-16;-0.12 -0.225 -1.11022302462516e-16],'MeshFaces',[6 2 1;1 5 6;8 4 3;3 7 8;6 7 3;3 2 6;5 1 4;4 8 5;4 1 2;2 3 4;7 6 5;5 8 7],'RCSPattern',[-8 -8;-8 -8],'RCSAzimuthAngles',[-180 180],'RCSElevationAngles',[-90 90]); struct('ActorID',16,'ClassID',4,'Length',0.24,'Width',0.45,'Height',1.7,'OriginOffset',[0 0 0],'MeshVertices',[0.12 -0.225 1.7;0.12 0.225 1.7;-0.12 0.225 1.7;-0.12 -0.225 1.7;0.12 -0.225 -1.11022302462516e-16;0.12 0.225 -1.11022302462516e-16;-0.12 0.225 -1.11022302462516e-16;-0.12 -0.225 -1.11022302462516e-16],'MeshFaces',[6 2 1;1 5 6;8 4 3;3 7 8;6 7 3;3 2 6;5 1 4;4 8 5;4 1 2;2 3 4;7 6 5;5 8 7],'RCSPattern',[-8 -8;-8 -8],'RCSAzimuthAngles',[-180 180],'RCSElevationAngles',[-90 90]); struct('ActorID',17,'ClassID',4,'Length',0.24,'Width',0.45,'Height',1.7,'OriginOffset',[0 0 0],'MeshVertices',[0.12 -0.225 1.7;0.12 0.225 1.7;-0.12 0.225 1.7;-0.12 -0.225 1.7;0.12 -0.225 -1.11022302462516e-16;0.12 0.225 -1.11022302462516e-16;-0.12 0.225 -1.11022302462516e-16;-0.12 -0.225 -1.11022302462516e-16],'MeshFaces',[6 2 1;1 5 6;8 4 3;3 7 8;6 7 3;3 2 6;5 1 4;4 8 5;4 1 2;2 3 4;7 6 5;5 8 7],'RCSPattern',[-8 -8;-8 -8],'RCSAzimuthAngles',[-180 180],'RCSElevationAngles',[-90 90]); struct('ActorID',18,'ClassID',4,'Length',0.24,'Width',0.45,'Height',1.7,'OriginOffset',[0 0 0],'MeshVertices',[0.12 -0.225 1.7;0.12 0.225 1.7;-0.12 0.225 1.7;-0.12 -0.225 1.7;0.12 -0.225 -1.11022302462516e-16;0.12 0.225 -1.11022302462516e-16;-0.12 0.225 -1.11022302462516e-16;-0.12 -0.225 -1.11022302462516e-16],'MeshFaces',[6 2 1;1 5 6;8 4 3;3 7 8;6 7 3;3 2 6;5 1 4;4 8 5;4 1 2;2 3 4;7 6 5;5 8 7],'RCSPattern',[-8 -8;-8 -8],'RCSAzimuthAngles',[-180 180],'RCSElevationAngles',[-90 90]); struct('ActorID',19,'ClassID',4,'Length',0.24,'Width',0.45,'Height',1.7,'OriginOffset',[0 0 0],'MeshVertices',[0.12 -0.225 1.7;0.12 0.225 1.7;-0.12 0.225 1.7;-0.12 -0.225 1.7;0.12 -0.225 -1.11022302462516e-16;0.12 0.225 -1.11022302462516e-16;-0.12 0.225 -1.11022302462516e-16;-0.12 -0.225 -1.11022302462516e-16],'MeshFaces',[6 2 1;1 5 6;8 4 3;3 7 8;6 7 3;3 2 6;5 1 4;4 8 5;4 1 2;2 3 4;7 6 5;5 8 7],'RCSPattern',[-8 -8;-8 -8],'RCSAzimuthAngles',[-180 180],'RCSElevationAngles',[-90 90]); struct('ActorID',20,'ClassID',4,'Length',0.24,'Width',0.45,'Height',1.7,'OriginOffset',[0 0 0],'MeshVertices',[0.12 -0.225 1.7;0.12 0.225 1.7;-0.12 0.225 1.7;-0.12 -0.225 1.7;0.12 -0.225 -1.11022302462516e-16;0.12 0.225 -1.11022302462516e-16;-0.12 0.225 -1.11022302462516e-16;-0.12 -0.225 -1.11022302462516e-16],'MeshFaces',[6 2 1;1 5 6;8 4 3;3 7 8;6 7 3;3 2 6;5 1 4;4 8 5;4 1 2;2 3 4;7 6 5;5 8 7],'RCSPattern',[-8 -8;-8 -8],'RCSAzimuthAngles',[-180 180],'RCSElevationAngles',[-90 90]); struct('ActorID',21,'ClassID',4,'Length',0.24,'Width',0.45,'Height',1.7,'OriginOffset',[0 0 0],'MeshVertices',[0.12 -0.225 1.7;0.12 0.225 1.7;-0.12 0.225 1.7;-0.12 -0.225 1.7;0.12 -0.225 -1.11022302462516e-16;0.12 0.225 -1.11022302462516e-16;-0.12 0.225 -1.11022302462516e-16;-0.12 -0.225 -1.11022302462516e-16],'MeshFaces',[6 2 1;1 5 6;8 4 3;3 7 8;6 7 3;3 2 6;5 1 4;4 8 5;4 1 2;2 3 4;7 6 5;5 8 7],'RCSPattern',[-8 -8;-8 -8],'RCSAzimuthAngles',[-180 180],'RCSElevationAngles',[-90 90]); struct('ActorID',22,'ClassID',4,'Length',0.24,'Width',0.45,'Height',1.7,'OriginOffset',[0 0 0],'MeshVertices',[0.12 -0.225 1.7;0.12 0.225 1.7;-0.12 0.225 1.7;-0.12 -0.225 1.7;0.12 -0.225 -1.11022302462516e-16;0.12 0.225 -1.11022302462516e-16;-0.12 0.225 -1.11022302462516e-16;-0.12 -0.225 -1.11022302462516e-16],'MeshFaces',[6 2 1;1 5 6;8 4 3;3 7 8;6 7 3;3 2 6;5 1 4;4 8 5;4 1 2;2 3 4;7 6 5;5 8 7],'RCSPattern',[-8 -8;-8 -8],'RCSAzimuthAngles',[-180 180],'RCSElevationAngles',[-90 90]); struct('ActorID',23,'ClassID',4,'Length',0.24,'Width',0.45,'Height',1.7,'OriginOffset',[0 0 0],'MeshVertices',[0.12 -0.225 1.7;0.12 0.225 1.7;-0.12 0.225 1.7;-0.12 -0.225 1.7;0.12 -0.225 -1.11022302462516e-16;0.12 0.225 -1.11022302462516e-16;-0.12 0.225 -1.11022302462516e-16;-0.12 -0.225 -1.11022302462516e-16],'MeshFaces',[6 2 1;1 5 6;8 4 3;3 7 8;6 7 3;3 2 6;5 1 4;4 8 5;4 1 2;2 3 4;7 6 5;5 8 7],'RCSPattern',[-8 -8;-8 -8],'RCSAzimuthAngles',[-180 180],'RCSElevationAngles',[-90 90]); struct('ActorID',24,'ClassID',4,'Length',0.24,'Width',0.45,'Height',1.7,'OriginOffset',[0 0 0],'MeshVertices',[0.12 -0.225 1.7;0.12 0.225 1.7;-0.12 0.225 1.7;-0.12 -0.225 1.7;0.12 -0.225 -1.11022302462516e-16;0.12 0.225 -1.11022302462516e-16;-0.12 0.225 -1.11022302462516e-16;-0.12 -0.225 -1.11022302462516e-16],'MeshFaces',[6 2 1;1 5 6;8 4 3;3 7 8;6 7 3;3 2 6;5 1 4;4 8 5;4 1 2;2 3 4;7 6 5;5 8 7],'RCSPattern',[-8 -8;-8 -8],'RCSAzimuthAngles',[-180 180],'RCSElevationAngles',[-90 90]); struct('ActorID',25,'ClassID',4,'Length',0.24,'Width',0.45,'Height',1.7,'OriginOffset',[0 0 0],'MeshVertices',[0.12 -0.225 1.7;0.12 0.225 1.7;-0.12 0.225 1.7;-0.12 -0.225 1.7;0.12 -0.225 -1.11022302462516e-16;0.12 0.225 -1.11022302462516e-16;-0.12 0.225 -1.11022302462516e-16;-0.12 -0.225 -1.11022302462516e-16],'MeshFaces',[6 2 1;1 5 6;8 4 3;3 7 8;6 7 3;3 2 6;5 1 4;4 8 5;4 1 2;2 3 4;7 6 5;5 8 7],'RCSPattern',[-8 -8;-8 -8],'RCSAzimuthAngles',[-180 180],'RCSElevationAngles',[-90 90]); struct('ActorID',26,'ClassID',4,'Length',0.24,'Width',0.45,'Height',1.7,'OriginOffset',[0 0 0],'MeshVertices',[0.12 -0.225 1.7;0.12 0.225 1.7;-0.12 0.225 1.7;-0.12 -0.225 1.7;0.12 -0.225 -1.11022302462516e-16;0.12 0.225 -1.11022302462516e-16;-0.12 0.225 -1.11022302462516e-16;-0.12 -0.225 -1.11022302462516e-16],'MeshFaces',[6 2 1;1 5 6;8 4 3;3 7 8;6 7 3;3 2 6;5 1 4;4 8 5;4 1 2;2 3 4;7 6 5;5 8 7],'RCSPattern',[-8 -8;-8 -8],'RCSAzimuthAngles',[-180 180],'RCSElevationAngles',[-90 90]); struct('ActorID',27,'ClassID',4,'Length',0.24,'Width',0.45,'Height',1.7,'OriginOffset',[0 0 0],'MeshVertices',[0.12 -0.225 1.7;0.12 0.225 1.7;-0.12 0.225 1.7;-0.12 -0.225 1.7;0.12 -0.225 -1.11022302462516e-16;0.12 0.225 -1.11022302462516e-16;-0.12 0.225 -1.11022302462516e-16;-0.12 -0.225 -1.11022302462516e-16],'MeshFaces',[6 2 1;1 5 6;8 4 3;3 7 8;6 7 3;3 2 6;5 1 4;4 8 5;4 1 2;2 3 4;7 6 5;5 8 7],'RCSPattern',[-8 -8;-8 -8],'RCSAzimuthAngles',[-180 180],'RCSElevationAngles',[-90 90]); struct('ActorID',28,'ClassID',3,'Length',1.7,'Width',0.45,'Height',1.7,'OriginOffset',[0 0 0],'MeshVertices',[0.85 -0.225 1.7;0.85 0.225 1.7;-0.85 0.225 1.7;-0.85 -0.225 1.7;0.85 -0.225 -1.11022302462516e-16;0.85 0.225 -1.11022302462516e-16;-0.85 0.225 -1.11022302462516e-16;-0.85 -0.225 -1.11022302462516e-16],'MeshFaces',[6 2 1;1 5 6;8 4 3;3 7 8;6 7 3;3 2 6;5 1 4;4 8 5;4 1 2;2 3 4;7 6 5;5 8 7],'RCSPattern',[10 10;10 10],'RCSAzimuthAngles',[-180 180],'RCSElevationAngles',[-90 90]); struct('ActorID',29,'ClassID',4,'Length',0.24,'Width',0.45,'Height',1.7,'OriginOffset',[0 0 0],'MeshVertices',[0.12 -0.225 1.7;0.12 0.225 1.7;-0.12 0.225 1.7;-0.12 -0.225 1.7;0.12 -0.225 -1.11022302462516e-16;0.12 0.225 -1.11022302462516e-16;-0.12 0.225 -1.11022302462516e-16;-0.12 -0.225 -1.11022302462516e-16],'MeshFaces',[6 2 1;1 5 6;8 4 3;3 7 8;6 7 3;3 2 6;5 1 4;4 8 5;4 1 2;2 3 4;7 6 5;5 8 7],'RCSPattern',[-8 -8;-8 -8],'RCSAzimuthAngles',[-180 180],'RCSElevationAngles',[-90 90])]  Intrinsics=driving.internal.cameraIntrinsics('FocalLength',[320 320],'PrincipalPoint',[320 240],'ImageSize',[480 640],'RadialDistortion',[0 0],'TangentialDistortion',[0 0],'Skew',0)
  Radar : drivingscenarioandsensors/Radar Detection Generator  SensorIndex=2  UpdateInterval=0.1  SensorLocation=[2.8 0.9]  Height=0.2  Yaw=31.1100682148404  Pitch=0  Roll=0  BusNameSource=Auto  BusName=BusRadarDetectionGenerator  MaxNumDetectionsSource=Property  MaxNumDetections=50  DetectionCoordinates=Ego Cartesian  SimulateUsing=Interpreted execution  AzimuthResolution=4  ElevationResolution=10  RangeResolution=2.5  RangeRateResolution=0.5  AzimuthBiasFraction=0.1  ElevationBiasFraction=0.1  RangeBiasFraction=0.05  RangeRateBiasFraction=0.05  FieldOfView=[90 1.5]  MaxRange=10  RangeRateLimits=[-100 100]  DetectionProbability=0.9  FalseAlarmRate=1e-06  ReferenceRange=15  ReferenceRCS=0  HasElevation=on  HasRangeRate=off  HasNoise=on  HasFalseAlarms=on  HasOcclusion=on  InitialSeedSource=Repeatable  InitialSeed=0  UsedSeed=0  ActorProfilesSource=MATLAB expression  ActorProfilesParameters=driving.internal.ActorProfilesRadarParameters  ActorProfilesExpression=[struct('ActorID',1,'ClassID',1,'Length',4.7,'Width',1.8,'Height',1.4,'OriginOffset',[-1.35 0 0],'MeshVertices',[3.7 -0.9 1.4;3.7 0.9 1.4;-1 0.9 1.4;-1 -0.9 1.4;3.7 -0.9 0;3.7 0.9 0;-1 0.9 0;-1 -0.9 0],'MeshFaces',[6 2 1;1 5 6;8 4 3;3 7 8;6 7 3;3 2 6;5 1 4;4 8 5;4 1 2;2 3 4;7 6 5;5 8 7],'RCSPattern',[10 10;10 10],'RCSAzimuthAngles',[-180 180],'RCSElevationAngles',[-90 90]); struct('ActorID',2,'ClassID',1,'Length',4.7,'Width',1.8,'Height',1.4,'OriginOffset',[-1.35 0 0],'MeshVertices',[3.7 -0.9 1.4;3.7 0.9 1.4;-1 0.9 1.4;-1 -0.9 1.4;3.7 -0.9 0;3.7 0.9 0;-1 0.9 0;-1 -0.9 0],'MeshFaces',[6 2 1;1 5 6;8 4 3;3 7 8;6 7 3;3 2 6;5 1 4;4 8 5;4 1 2;2 3 4;7 6 5;5 8 7],'RCSPattern',[10 10;10 10],'RCSAzimuthAngles',[-180 180],'RCSElevationAngles',[-90 90]); struct('ActorID',3,'ClassID',1,'Length',4.7,'Width',1.8,'Height',1.4,'OriginOffset',[-1.35 0 0],'MeshVertices',[3.7 -0.9 1.4;3.7 0.9 1.4;-1 0.9 1.4;-1 -0.9 1.4;3.7 -0.9 0;3.7 0.9 0;-1 0.9 0;-1 -0.9 0],'MeshFaces',[6 2 1;1 5 6;8 4 3;3 7 8;6 7 3;3 2 6;5 1 4;4 8 5;4 1 2;2 3 4;7 6 5;5 8 7],'RCSPattern',[10 10;10 10],'RCSAzimuthAngles',[-180 180],'RCSElevationAngles',[-90 90]); struct('ActorID',4,'ClassID',1,'Length',4.7,'Width',1.8,'Height',1.4,'OriginOffset',[-1.35 0 0],'MeshVertices',[3.7 -0.9 1.4;3.7 0.9 1.4;-1 0.9 1.4;-1 -0.9 1.4;3.7 -0.9 0;3.7 0.9 0;-1 0.9 0;-1 -0.9 0],'MeshFaces',[6 2 1;1 5 6;8 4 3;3 7 8;6 7 3;3 2 6;5 1 4;4 8 5;4 1 2;2 3 4;7 6 5;5 8 7],'RCSPattern',[10 10;10 10],'RCSAzimuthAngles',[-180 180],'RCSElevationAngles',[-90 90]); struct('ActorID',5,'ClassID',1,'Length',4.7,'Width',1.8,'Height',1.4,'OriginOffset',[-1.35 0 0],'MeshVertices',[3.7 -0.9 1.4;3.7 0.9 1.4;-1 0.9 1.4;-1 -0.9 1.4;3.7 -0.9 0;3.7 0.9 0;-1 0.9 0;-1 -0.9 0],'MeshFaces',[6 2 1;1 5 6;8 4 3;3 7 8;6 7 3;3 2 6;5 1 4;4 8 5;4 1 2;2 3 4;7 6 5;5 8 7],'RCSPattern',[10 10;10 10],'RCSAzimuthAngles',[-180 180],'RCSElevationAngles',[-90 90]); struct('ActorID',6,'ClassID',4,'Length',0.24,'Width',0.45,'Height',1.7,'OriginOffset',[0 0 0],'MeshVertices',[0.12 -0.225 1.7;0.12 0.225 1.7;-0.12 0.225 1.7;-0.12 -0.225 1.7;0.12 -0.225 -1.11022302462516e-16;0.12 0.225 -1.11022302462516e-16;-0.12 0.225 -1.11022302462516e-16;-0.12 -0.225 -1.11022302462516e-16],'MeshFaces',[6 2 1;1 5 6;8 4 3;3 7 8;6 7 3;3 2 6;5 1 4;4 8 5;4 1 2;2 3 4;7 6 5;5 8 7],'RCSPattern',[-8 -8;-8 -8],'RCSAzimuthAngles',[-180 180],'RCSElevationAngles',[-90 90]); struct('ActorID',7,'ClassID',4,'Length',0.24,'Width',0.45,'Height',1.7,'OriginOffset',[0 0 0],'MeshVertices',[0.12 -0.225 1.7;0.12 0.225 1.7;-0.12 0.225 1.7;-0.12 -0.225 1.7;0.12 -0.225 -1.11022302462516e-16;0.12 0.225 -1.11022302462516e-16;-0.12 0.225 -1.11022302462516e-16;-0.12 -0.225 -1.11022302462516e-16],'MeshFaces',[6 2 1;1 5 6;8 4 3;3 7 8;6 7 3;3 2 6;5 1 4;4 8 5;4 1 2;2 3 4;7 6 5;5 8 7],'RCSPattern',[-8 -8;-8 -8],'RCSAzimuthAngles',[-180 180],'RCSElevationAngles',[-90 90]); struct('ActorID',8,'ClassID',4,'Length',0.24,'Width',0.45,'Height',1.7,'OriginOffset',[0 0 0],'MeshVertices',[0.12 -0.225 1.7;0.12 0.225 1.7;-0.12 0.225 1.7;-0.12 -0.225 1.7;0.12 -0.225 -1.11022302462516e-16;0.12 0.225 -1.11022302462516e-16;-0.12 0.225 -1.11022302462516e-16;-0.12 -0.225 -1.11022302462516e-16],'MeshFaces',[6 2 1;1 5 6;8 4 3;3 7 8;6 7 3;3 2 6;5 1 4;4 8 5;4 1 2;2 3 4;7 6 5;5 8 7],'RCSPattern',[-8 -8;-8 -8],'RCSAzimuthAngles',[-180 180],'RCSElevationAngles',[-90 90]); struct('ActorID',9,'ClassID',4,'Length',0.24,'Width',0.45,'Height',1.7,'OriginOffset',[0 0 0],'MeshVertices',[0.12 -0.225 1.7;0.12 0.225 1.7;-0.12 0.225 1.7;-0.12 -0.225 1.7;0.12 -0.225 -1.11022302462516e-16;0.12 0.225 -1.11022302462516e-16;-0.12 0.225 -1.11022302462516e-16;-0.12 -0.225 -1.11022302462516e-16],'MeshFaces',[6 2 1;1 5 6;8 4 3;3 7 8;6 7 3;3 2 6;5 1 4;4 8 5;4 1 2;2 3 4;7 6 5;5 8 7],'RCSPattern',[-8 -8;-8 -8],'RCSAzimuthAngles',[-180 180],'RCSElevationAngles',[-90 90]); struct('ActorID',10,'ClassID',4,'Length',0.24,'Width',0.45,'Height',1.7,'OriginOffset',[0 0 0],'MeshVertices',[0.12 -0.225 1.7;0.12 0.225 1.7;-0.12 0.225 1.7;-0.12 -0.225 1.7;0.12 -0.225 -1.11022302462516e-16;0.12 0.225 -1.11022302462516e-16;-0.12 0.225 -1.11022302462516e-16;-0.12 -0.225 -1.11022302462516e-16],'MeshFaces',[6 2 1;1 5 6;8 4 3;3 7 8;6 7 3;3 2 6;5 1 4;4 8 5;4 1 2;2 3 4;7 6 5;5 8 7],'RCSPattern',[-8 -8;-8 -8],'RCSAzimuthAngles',[-180 180],'RCSElevationAngles',[-90 90]); struct('ActorID',11,'ClassID',4,'Length',0.24,'Width',0.45,'Height',1.7,'OriginOffset',[0 0 0],'MeshVertices',[0.12 -0.225 1.7;0.12 0.225 1.7;-0.12 0.225 1.7;-0.12 -0.225 1.7;0.12 -0.225 -1.11022302462516e-16;0.12 0.225 -1.11022302462516e-16;-0.12 0.225 -1.11022302462516e-16;-0.12 -0.225 -1.11022302462516e-16],'MeshFaces',[6 2 1;1 5 6;8 4 3;3 7 8;6 7 3;3 2 6;5 1 4;4 8 5;4 1 2;2 3 4;7 6 5;5 8 7],'RCSPattern',[-8 -8;-8 -8],'RCSAzimuthAngles',[-180 180],'RCSElevationAngles',[-90 90]); struct('ActorID',12,'ClassID',4,'Length',0.24,'Width',0.45,'Height',1.7,'OriginOffset',[0 0 0],'MeshVertices',[0.12 -0.225 1.7;0.12 0.225 1.7;-0.12 0.225 1.7;-0.12 -0.225 1.7;0.12 -0.225 -1.11022302462516e-16;0.12 0.225 -1.11022302462516e-16;-0.12 0.225 -1.11022302462516e-16;-0.12 -0.225 -1.11022302462516e-16],'MeshFaces',[6 2 1;1 5 6;8 4 3;3 7 8;6 7 3;3 2 6;5 1 4;4 8 5;4 1 2;2 3 4;7 6 5;5 8 7],'RCSPattern',[-8 -8;-8 -8],'RCSAzimuthAngles',[-180 180],'RCSElevationAngles',[-90 90]); struct('ActorID',13,'ClassID',4,'Length',0.24,'Width',0.45,'Height',1.7,'OriginOffset',[0 0 0],'MeshVertices',[0.12 -0.225 1.7;0.12 0.225 1.7;-0.12 0.225 1.7;-0.12 -0.225 1.7;0.12 -0.225 -1.11022302462516e-16;0.12 0.225 -1.11022302462516e-16;-0.12 0.225 -1.11022302462516e-16;-0.12 -0.225 -1.11022302462516e-16],'MeshFaces',[6 2 1;1 5 6;8 4 3;3 7 8;6 7 3;3 2 6;5 1 4;4 8 5;4 1 2;2 3 4;7 6 5;5 8 7],'RCSPattern',[-8 -8;-8 -8],'RCSAzimuthAngles',[-180 180],'RCSElevationAngles',[-90 90]); struct('ActorID',14,'ClassID',4,'Length',0.24,'Width',0.45,'Height',1.7,'OriginOffset',[0 0 0],'MeshVertices',[0.12 -0.225 1.7;0.12 0.225 1.7;-0.12 0.225 1.7;-0.12 -0.225 1.7;0.12 -0.225 -1.11022302462516e-16;0.12 0.225 -1.11022302462516e-16;-0.12 0.225 -1.11022302462516e-16;-0.12 -0.225 -1.11022302462516e-16],'MeshFaces',[6 2 1;1 5 6;8 4 3;3 7 8;6 7 3;3 2 6;5 1 4;4 8 5;4 1 2;2 3 4;7 6 5;5 8 7],'RCSPattern',[-8 -8;-8 -8],'RCSAzimuthAngles',[-180 180],'RCSElevationAngles',[-90 90]); struct('ActorID',15,'ClassID',4,'Length',0.24,'Width',0.45,'Height',1.7,'OriginOffset',[0 0 0],'MeshVertices',[0.12 -0.225 1.7;0.12 0.225 1.7;-0.12 0.225 1.7;-0.12 -0.225 1.7;0.12 -0.225 -1.11022302462516e-16;0.12 0.225 -1.11022302462516e-16;-0.12 0.225 -1.11022302462516e-16;-0.12 -0.225 -1.11022302462516e-16],'MeshFaces',[6 2 1;1 5 6;8 4 3;3 7 8;6 7 3;3 2 6;5 1 4;4 8 5;4 1 2;2 3 4;7 6 5;5 8 7],'RCSPattern',[-8 -8;-8 -8],'RCSAzimuthAngles',[-180 180],'RCSElevationAngles',[-90 90]); struct('ActorID',16,'ClassID',4,'Length',0.24,'Width',0.45,'Height',1.7,'OriginOffset',[0 0 0],'MeshVertices',[0.12 -0.225 1.7;0.12 0.225 1.7;-0.12 0.225 1.7;-0.12 -0.225 1.7;0.12 -0.225 -1.11022302462516e-16;0.12 0.225 -1.11022302462516e-16;-0.12 0.225 -1.11022302462516e-16;-0.12 -0.225 -1.11022302462516e-16],'MeshFaces',[6 2 1;1 5 6;8 4 3;3 7 8;6 7 3;3 2 6;5 1 4;4 8 5;4 1 2;2 3 4;7 6 5;5 8 7],'RCSPattern',[-8 -8;-8 -8],'RCSAzimuthAngles',[-180 180],'RCSElevationAngles',[-90 90]); struct('ActorID',17,'ClassID',4,'Length',0.24,'Width',0.45,'Height',1.7,'OriginOffset',[0 0 0],'MeshVertices',[0.12 -0.225 1.7;0.12 0.225 1.7;-0.12 0.225 1.7;-0.12 -0.225 1.7;0.12 -0.225 -1.11022302462516e-16;0.12 0.225 -1.11022302462516e-16;-0.12 0.225 -1.11022302462516e-16;-0.12 -0.225 -1.11022302462516e-16],'MeshFaces',[6 2 1;1 5 6;8 4 3;3 7 8;6 7 3;3 2 6;5 1 4;4 8 5;4 1 2;2 3 4;7 6 5;5 8 7],'RCSPattern',[-8 -8;-8 -8],'RCSAzimuthAngles',[-180 180],'RCSElevationAngles',[-90 90]); struct('ActorID',18,'ClassID',4,'Length',0.24,'Width',0.45,'Height',1.7,'OriginOffset',[0 0 0],'MeshVertices',[0.12 -0.225 1.7;0.12 0.225 1.7;-0.12 0.225 1.7;-0.12 -0.225 1.7;0.12 -0.225 -1.11022302462516e-16;0.12 0.225 -1.11022302462516e-16;-0.12 0.225 -1.11022302462516e-16;-0.12 -0.225 -1.11022302462516e-16],'MeshFaces',[6 2 1;1 5 6;8 4 3;3 7 8;6 7 3;3 2 6;5 1 4;4 8 5;4 1 2;2 3 4;7 6 5;5 8 7],'RCSPattern',[-8 -8;-8 -8],'RCSAzimuthAngles',[-180 180],'RCSElevationAngles',[-90 90]); struct('ActorID',19,'ClassID',4,'Length',0.24,'Width',0.45,'Height',1.7,'OriginOffset',[0 0 0],'MeshVertices',[0.12 -0.225 1.7;0.12 0.225 1.7;-0.12 0.225 1.7;-0.12 -0.225 1.7;0.12 -0.225 -1.11022302462516e-16;0.12 0.225 -1.11022302462516e-16;-0.12 0.225 -1.11022302462516e-16;-0.12 -0.225 -1.11022302462516e-16],'MeshFaces',[6 2 1;1 5 6;8 4 3;3 7 8;6 7 3;3 2 6;5 1 4;4 8 5;4 1 2;2 3 4;7 6 5;5 8 7],'RCSPattern',[-8 -8;-8 -8],'RCSAzimuthAngles',[-180 180],'RCSElevationAngles',[-90 90]); struct('ActorID',20,'ClassID',4,'Length',0.24,'Width',0.45,'Height',1.7,'OriginOffset',[0 0 0],'MeshVertices',[0.12 -0.225 1.7;0.12 0.225 1.7;-0.12 0.225 1.7;-0.12 -0.225 1.7;0.12 -0.225 -1.11022302462516e-16;0.12 0.225 -1.11022302462516e-16;-0.12 0.225 -1.11022302462516e-16;-0.12 -0.225 -1.11022302462516e-16],'MeshFaces',[6 2 1;1 5 6;8 4 3;3 7 8;6 7 3;3 2 6;5 1 4;4 8 5;4 1 2;2 3 4;7 6 5;5 8 7],'RCSPattern',[-8 -8;-8 -8],'RCSAzimuthAngles',[-180 180],'RCSElevationAngles',[-90 90]); struct('ActorID',21,'ClassID',4,'Length',0.24,'Width',0.45,'Height',1.7,'OriginOffset',[0 0 0],'MeshVertices',[0.12 -0.225 1.7;0.12 0.225 1.7;-0.12 0.225 1.7;-0.12 -0.225 1.7;0.12 -0.225 -1.11022302462516e-16;0.12 0.225 -1.11022302462516e-16;-0.12 0.225 -1.11022302462516e-16;-0.12 -0.225 -1.11022302462516e-16],'MeshFaces',[6 2 1;1 5 6;8 4 3;3 7 8;6 7 3;3 2 6;5 1 4;4 8 5;4 1 2;2 3 4;7 6 5;5 8 7],'RCSPattern',[-8 -8;-8 -8],'RCSAzimuthAngles',[-180 180],'RCSElevationAngles',[-90 90]); struct('ActorID',22,'ClassID',4,'Length',0.24,'Width',0.45,'Height',1.7,'OriginOffset',[0 0 0],'MeshVertices',[0.12 -0.225 1.7;0.12 0.225 1.7;-0.12 0.225 1.7;-0.12 -0.225 1.7;0.12 -0.225 -1.11022302462516e-16;0.12 0.225 -1.11022302462516e-16;-0.12 0.225 -1.11022302462516e-16;-0.12 -0.225 -1.11022302462516e-16],'MeshFaces',[6 2 1;1 5 6;8 4 3;3 7 8;6 7 3;3 2 6;5 1 4;4 8 5;4 1 2;2 3 4;7 6 5;5 8 7],'RCSPattern',[-8 -8;-8 -8],'RCSAzimuthAngles',[-180 180],'RCSElevationAngles',[-90 90]); struct('ActorID',23,'ClassID',4,'Length',0.24,'Width',0.45,'Height',1.7,'OriginOffset',[0 0 0],'MeshVertices',[0.12 -0.225 1.7;0.12 0.225 1.7;-0.12 0.225 1.7;-0.12 -0.225 1.7;0.12 -0.225 -1.11022302462516e-16;0.12 0.225 -1.11022302462516e-16;-0.12 0.225 -1.11022302462516e-16;-0.12 -0.225 -1.11022302462516e-16],'MeshFaces',[6 2 1;1 5 6;8 4 3;3 7 8;6 7 3;3 2 6;5 1 4;4 8 5;4 1 2;2 3 4;7 6 5;5 8 7],'RCSPattern',[-8 -8;-8 -8],'RCSAzimuthAngles',[-180 180],'RCSElevationAngles',[-90 90]); struct('ActorID',24,'ClassID',4,'Length',0.24,'Width',0.45,'Height',1.7,'OriginOffset',[0 0 0],'MeshVertices',[0.12 -0.225 1.7;0.12 0.225 1.7;-0.12 0.225 1.7;-0.12 -0.225 1.7;0.12 -0.225 -1.11022302462516e-16;0.12 0.225 -1.11022302462516e-16;-0.12 0.225 -1.11022302462516e-16;-0.12 -0.225 -1.11022302462516e-16],'MeshFaces',[6 2 1;1 5 6;8 4 3;3 7 8;6 7 3;3 2 6;5 1 4;4 8 5;4 1 2;2 3 4;7 6 5;5 8 7],'RCSPattern',[-8 -8;-8 -8],'RCSAzimuthAngles',[-180 180],'RCSElevationAngles',[-90 90]); struct('ActorID',25,'ClassID',4,'Length',0.24,'Width',0.45,'Height',1.7,'OriginOffset',[0 0 0],'MeshVertices',[0.12 -0.225 1.7;0.12 0.225 1.7;-0.12 0.225 1.7;-0.12 -0.225 1.7;0.12 -0.225 -1.11022302462516e-16;0.12 0.225 -1.11022302462516e-16;-0.12 0.225 -1.11022302462516e-16;-0.12 -0.225 -1.11022302462516e-16],'MeshFaces',[6 2 1;1 5 6;8 4 3;3 7 8;6 7 3;3 2 6;5 1 4;4 8 5;4 1 2;2 3 4;7 6 5;5 8 7],'RCSPattern',[-8 -8;-8 -8],'RCSAzimuthAngles',[-180 180],'RCSElevationAngles',[-90 90]); struct('ActorID',26,'ClassID',4,'Length',0.24,'Width',0.45,'Height',1.7,'OriginOffset',[0 0 0],'MeshVertices',[0.12 -0.225 1.7;0.12 0.225 1.7;-0.12 0.225 1.7;-0.12 -0.225 1.7;0.12 -0.225 -1.11022302462516e-16;0.12 0.225 -1.11022302462516e-16;-0.12 0.225 -1.11022302462516e-16;-0.12 -0.225 -1.11022302462516e-16],'MeshFaces',[6 2 1;1 5 6;8 4 3;3 7 8;6 7 3;3 2 6;5 1 4;4 8 5;4 1 2;2 3 4;7 6 5;5 8 7],'RCSPattern',[-8 -8;-8 -8],'RCSAzimuthAngles',[-180 180],'RCSElevationAngles',[-90 90]); struct('ActorID',27,'ClassID',4,'Length',0.24,'Width',0.45,'Height',1.7,'OriginOffset',[0 0 0],'MeshVertices',[0.12 -0.225 1.7;0.12 0.225 1.7;-0.12 0.225 1.7;-0.12 -0.225 1.7;0.12 -0.225 -1.11022302462516e-16;0.12 0.225 -1.11022302462516e-16;-0.12 0.225 -1.11022302462516e-16;-0.12 -0.225 -1.11022302462516e-16],'MeshFaces',[6 2 1;1 5 6;8 4 3;3 7 8;6 7 3;3 2 6;5 1 4;4 8 5;4 1 2;2 3 4;7 6 5;5 8 7],'RCSPattern',[-8 -8;-8 -8],'RCSAzimuthAngles',[-180 180],'RCSElevationAngles',[-90 90]); struct('ActorID',28,'ClassID',3,'Length',1.7,'Width',0.45,'Height',1.7,'OriginOffset',[0 0 0],'MeshVertices',[0.85 -0.225 1.7;0.85 0.225 1.7;-0.85 0.225 1.7;-0.85 -0.225 1.7;0.85 -0.225 -1.11022302462516e-16;0.85 0.225 -1.11022302462516e-16;-0.85 0.225 -1.11022302462516e-16;-0.85 -0.225 -1.11022302462516e-16],'MeshFaces',[6 2 1;1 5 6;8 4 3;3 7 8;6 7 3;3 2 6;5 1 4;4 8 5;4 1 2;2 3 4;7 6 5;5 8 7],'RCSPattern',[10 10;10 10],'RCSAzimuthAngles',[-180 180],'RCSElevationAngles',[-90 90]); struct('ActorID',29,'ClassID',4,'Length',0.24,'Width',0.45,'Height',1.7,'OriginOffset',[0 0 0],'MeshVertices',[0.12 -0.225 1.7;0.12 0.225 1.7;-0.12 0.225 1.7;-0.12 -0.225 1.7;0.12 -0.225 -1.11022302462516e-16;0.12 0.225 -1.11022302462516e-16;-0.12 0.225 -1.11022302462516e-16;-0.12 -0.225 -1.11022302462516e-16],'MeshFaces',[6 2 1;1 5 6;8 4 3;3 7 8;6 7 3;3 2 6;5 1 4;4 8 5;4 1 2;2 3 4;7 6 5;5 8 7],'RCSPattern',[-8 -8;-8 -8],'RCSAzimuthAngles',[-180 180],'RCSElevationAngles',[-90 90])]
      settings: SourceProductBaseCode=DR
  Radar1 : drivingscenarioandsensors/Radar Detection Generator  SensorIndex=3  UpdateInterval=0.1  SensorLocation=[2.8 -0.9]  Height=0.2  Yaw=-30.9957832361237  Pitch=0  Roll=0  BusNameSource=Auto  BusName=BusRadarDetectionGenerator  MaxNumDetectionsSource=Property  MaxNumDetections=50  DetectionCoordinates=Ego Cartesian  SimulateUsing=Interpreted execution  AzimuthResolution=4  ElevationResolution=10  RangeResolution=2.5  RangeRateResolution=0.5  AzimuthBiasFraction=0.1  ElevationBiasFraction=0.1  RangeBiasFraction=0.05  RangeRateBiasFraction=0.05  FieldOfView=[90 5]  MaxRange=10  RangeRateLimits=[-100 100]  DetectionProbability=0.9  FalseAlarmRate=1e-06  ReferenceRange=15  ReferenceRCS=0  HasElevation=on  HasRangeRate=off  HasNoise=on  HasFalseAlarms=on  HasOcclusion=on  InitialSeedSource=Repeatable  InitialSeed=0  UsedSeed=0  ActorProfilesSource=MATLAB expression  ActorProfilesParameters=driving.internal.ActorProfilesRadarParameters  ActorProfilesExpression=[struct('ActorID',1,'ClassID',1,'Length',4.7,'Width',1.8,'Height',1.4,'OriginOffset',[-1.35 0 0],'MeshVertices',[3.7 -0.9 1.4;3.7 0.9 1.4;-1 0.9 1.4;-1 -0.9 1.4;3.7 -0.9 0;3.7 0.9 0;-1 0.9 0;-1 -0.9 0],'MeshFaces',[6 2 1;1 5 6;8 4 3;3 7 8;6 7 3;3 2 6;5 1 4;4 8 5;4 1 2;2 3 4;7 6 5;5 8 7],'RCSPattern',[10 10;10 10],'RCSAzimuthAngles',[-180 180],'RCSElevationAngles',[-90 90]); struct('ActorID',2,'ClassID',1,'Length',4.7,'Width',1.8,'Height',1.4,'OriginOffset',[-1.35 0 0],'MeshVertices',[3.7 -0.9 1.4;3.7 0.9 1.4;-1 0.9 1.4;-1 -0.9 1.4;3.7 -0.9 0;3.7 0.9 0;-1 0.9 0;-1 -0.9 0],'MeshFaces',[6 2 1;1 5 6;8 4 3;3 7 8;6 7 3;3 2 6;5 1 4;4 8 5;4 1 2;2 3 4;7 6 5;5 8 7],'RCSPattern',[10 10;10 10],'RCSAzimuthAngles',[-180 180],'RCSElevationAngles',[-90 90]); struct('ActorID',3,'ClassID',1,'Length',4.7,'Width',1.8,'Height',1.4,'OriginOffset',[-1.35 0 0],'MeshVertices',[3.7 -0.9 1.4;3.7 0.9 1.4;-1 0.9 1.4;-1 -0.9 1.4;3.7 -0.9 0;3.7 0.9 0;-1 0.9 0;-1 -0.9 0],'MeshFaces',[6 2 1;1 5 6;8 4 3;3 7 8;6 7 3;3 2 6;5 1 4;4 8 5;4 1 2;2 3 4;7 6 5;5 8 7],'RCSPattern',[10 10;10 10],'RCSAzimuthAngles',[-180 180],'RCSElevationAngles',[-90 90]); struct('ActorID',4,'ClassID',1,'Length',4.7,'Width',1.8,'Height',1.4,'OriginOffset',[-1.35 0 0],'MeshVertices',[3.7 -0.9 1.4;3.7 0.9 1.4;-1 0.9 1.4;-1 -0.9 1.4;3.7 -0.9 0;3.7 0.9 0;-1 0.9 0;-1 -0.9 0],'MeshFaces',[6 2 1;1 5 6;8 4 3;3 7 8;6 7 3;3 2 6;5 1 4;4 8 5;4 1 2;2 3 4;7 6 5;5 8 7],'RCSPattern',[10 10;10 10],'RCSAzimuthAngles',[-180 180],'RCSElevationAngles',[-90 90]); struct('ActorID',5,'ClassID',1,'Length',4.7,'Width',1.8,'Height',1.4,'OriginOffset',[-1.35 0 0],'MeshVertices',[3.7 -0.9 1.4;3.7 0.9 1.4;-1 0.9 1.4;-1 -0.9 1.4;3.7 -0.9 0;3.7 0.9 0;-1 0.9 0;-1 -0.9 0],'MeshFaces',[6 2 1;1 5 6;8 4 3;3 7 8;6 7 3;3 2 6;5 1 4;4 8 5;4 1 2;2 3 4;7 6 5;5 8 7],'RCSPattern',[10 10;10 10],'RCSAzimuthAngles',[-180 180],'RCSElevationAngles',[-90 90]); struct('ActorID',6,'ClassID',4,'Length',0.24,'Width',0.45,'Height',1.7,'OriginOffset',[0 0 0],'MeshVertices',[0.12 -0.225 1.7;0.12 0.225 1.7;-0.12 0.225 1.7;-0.12 -0.225 1.7;0.12 -0.225 -1.11022302462516e-16;0.12 0.225 -1.11022302462516e-16;-0.12 0.225 -1.11022302462516e-16;-0.12 -0.225 -1.11022302462516e-16],'MeshFaces',[6 2 1;1 5 6;8 4 3;3 7 8;6 7 3;3 2 6;5 1 4;4 8 5;4 1 2;2 3 4;7 6 5;5 8 7],'RCSPattern',[-8 -8;-8 -8],'RCSAzimuthAngles',[-180 180],'RCSElevationAngles',[-90 90]); struct('ActorID',7,'ClassID',4,'Length',0.24,'Width',0.45,'Height',1.7,'OriginOffset',[0 0 0],'MeshVertices',[0.12 -0.225 1.7;0.12 0.225 1.7;-0.12 0.225 1.7;-0.12 -0.225 1.7;0.12 -0.225 -1.11022302462516e-16;0.12 0.225 -1.11022302462516e-16;-0.12 0.225 -1.11022302462516e-16;-0.12 -0.225 -1.11022302462516e-16],'MeshFaces',[6 2 1;1 5 6;8 4 3;3 7 8;6 7 3;3 2 6;5 1 4;4 8 5;4 1 2;2 3 4;7 6 5;5 8 7],'RCSPattern',[-8 -8;-8 -8],'RCSAzimuthAngles',[-180 180],'RCSElevationAngles',[-90 90]); struct('ActorID',8,'ClassID',4,'Length',0.24,'Width',0.45,'Height',1.7,'OriginOffset',[0 0 0],'MeshVertices',[0.12 -0.225 1.7;0.12 0.225 1.7;-0.12 0.225 1.7;-0.12 -0.225 1.7;0.12 -0.225 -1.11022302462516e-16;0.12 0.225 -1.11022302462516e-16;-0.12 0.225 -1.11022302462516e-16;-0.12 -0.225 -1.11022302462516e-16],'MeshFaces',[6 2 1;1 5 6;8 4 3;3 7 8;6 7 3;3 2 6;5 1 4;4 8 5;4 1 2;2 3 4;7 6 5;5 8 7],'RCSPattern',[-8 -8;-8 -8],'RCSAzimuthAngles',[-180 180],'RCSElevationAngles',[-90 90]); struct('ActorID',9,'ClassID',4,'Length',0.24,'Width',0.45,'Height',1.7,'OriginOffset',[0 0 0],'MeshVertices',[0.12 -0.225 1.7;0.12 0.225 1.7;-0.12 0.225 1.7;-0.12 -0.225 1.7;0.12 -0.225 -1.11022302462516e-16;0.12 0.225 -1.11022302462516e-16;-0.12 0.225 -1.11022302462516e-16;-0.12 -0.225 -1.11022302462516e-16],'MeshFaces',[6 2 1;1 5 6;8 4 3;3 7 8;6 7 3;3 2 6;5 1 4;4 8 5;4 1 2;2 3 4;7 6 5;5 8 7],'RCSPattern',[-8 -8;-8 -8],'RCSAzimuthAngles',[-180 180],'RCSElevationAngles',[-90 90]); struct('ActorID',10,'ClassID',4,'Length',0.24,'Width',0.45,'Height',1.7,'OriginOffset',[0 0 0],'MeshVertices',[0.12 -0.225 1.7;0.12 0.225 1.7;-0.12 0.225 1.7;-0.12 -0.225 1.7;0.12 -0.225 -1.11022302462516e-16;0.12 0.225 -1.11022302462516e-16;-0.12 0.225 -1.11022302462516e-16;-0.12 -0.225 -1.11022302462516e-16],'MeshFaces',[6 2 1;1 5 6;8 4 3;3 7 8;6 7 3;3 2 6;5 1 4;4 8 5;4 1 2;2 3 4;7 6 5;5 8 7],'RCSPattern',[-8 -8;-8 -8],'RCSAzimuthAngles',[-180 180],'RCSElevationAngles',[-90 90]); struct('ActorID',11,'ClassID',4,'Length',0.24,'Width',0.45,'Height',1.7,'OriginOffset',[0 0 0],'MeshVertices',[0.12 -0.225 1.7;0.12 0.225 1.7;-0.12 0.225 1.7;-0.12 -0.225 1.7;0.12 -0.225 -1.11022302462516e-16;0.12 0.225 -1.11022302462516e-16;-0.12 0.225 -1.11022302462516e-16;-0.12 -0.225 -1.11022302462516e-16],'MeshFaces',[6 2 1;1 5 6;8 4 3;3 7 8;6 7 3;3 2 6;5 1 4;4 8 5;4 1 2;2 3 4;7 6 5;5 8 7],'RCSPattern',[-8 -8;-8 -8],'RCSAzimuthAngles',[-180 180],'RCSElevationAngles',[-90 90]); struct('ActorID',12,'ClassID',4,'Length',0.24,'Width',0.45,'Height',1.7,'OriginOffset',[0 0 0],'MeshVertices',[0.12 -0.225 1.7;0.12 0.225 1.7;-0.12 0.225 1.7;-0.12 -0.225 1.7;0.12 -0.225 -1.11022302462516e-16;0.12 0.225 -1.11022302462516e-16;-0.12 0.225 -1.11022302462516e-16;-0.12 -0.225 -1.11022302462516e-16],'MeshFaces',[6 2 1;1 5 6;8 4 3;3 7 8;6 7 3;3 2 6;5 1 4;4 8 5;4 1 2;2 3 4;7 6 5;5 8 7],'RCSPattern',[-8 -8;-8 -8],'RCSAzimuthAngles',[-180 180],'RCSElevationAngles',[-90 90]); struct('ActorID',13,'ClassID',4,'Length',0.24,'Width',0.45,'Height',1.7,'OriginOffset',[0 0 0],'MeshVertices',[0.12 -0.225 1.7;0.12 0.225 1.7;-0.12 0.225 1.7;-0.12 -0.225 1.7;0.12 -0.225 -1.11022302462516e-16;0.12 0.225 -1.11022302462516e-16;-0.12 0.225 -1.11022302462516e-16;-0.12 -0.225 -1.11022302462516e-16],'MeshFaces',[6 2 1;1 5 6;8 4 3;3 7 8;6 7 3;3 2 6;5 1 4;4 8 5;4 1 2;2 3 4;7 6 5;5 8 7],'RCSPattern',[-8 -8;-8 -8],'RCSAzimuthAngles',[-180 180],'RCSElevationAngles',[-90 90]); struct('ActorID',14,'ClassID',4,'Length',0.24,'Width',0.45,'Height',1.7,'OriginOffset',[0 0 0],'MeshVertices',[0.12 -0.225 1.7;0.12 0.225 1.7;-0.12 0.225 1.7;-0.12 -0.225 1.7;0.12 -0.225 -1.11022302462516e-16;0.12 0.225 -1.11022302462516e-16;-0.12 0.225 -1.11022302462516e-16;-0.12 -0.225 -1.11022302462516e-16],'MeshFaces',[6 2 1;1 5 6;8 4 3;3 7 8;6 7 3;3 2 6;5 1 4;4 8 5;4 1 2;2 3 4;7 6 5;5 8 7],'RCSPattern',[-8 -8;-8 -8],'RCSAzimuthAngles',[-180 180],'RCSElevationAngles',[-90 90]); struct('ActorID',15,'ClassID',4,'Length',0.24,'Width',0.45,'Height',1.7,'OriginOffset',[0 0 0],'MeshVertices',[0.12 -0.225 1.7;0.12 0.225 1.7;-0.12 0.225 1.7;-0.12 -0.225 1.7;0.12 -0.225 -1.11022302462516e-16;0.12 0.225 -1.11022302462516e-16;-0.12 0.225 -1.11022302462516e-16;-0.12 -0.225 -1.11022302462516e-16],'MeshFaces',[6 2 1;1 5 6;8 4 3;3 7 8;6 7 3;3 2 6;5 1 4;4 8 5;4 1 2;2 3 4;7 6 5;5 8 7],'RCSPattern',[-8 -8;-8 -8],'RCSAzimuthAngles',[-180 180],'RCSElevationAngles',[-90 90]); struct('ActorID',16,'ClassID',4,'Length',0.24,'Width',0.45,'Height',1.7,'OriginOffset',[0 0 0],'MeshVertices',[0.12 -0.225 1.7;0.12 0.225 1.7;-0.12 0.225 1.7;-0.12 -0.225 1.7;0.12 -0.225 -1.11022302462516e-16;0.12 0.225 -1.11022302462516e-16;-0.12 0.225 -1.11022302462516e-16;-0.12 -0.225 -1.11022302462516e-16],'MeshFaces',[6 2 1;1 5 6;8 4 3;3 7 8;6 7 3;3 2 6;5 1 4;4 8 5;4 1 2;2 3 4;7 6 5;5 8 7],'RCSPattern',[-8 -8;-8 -8],'RCSAzimuthAngles',[-180 180],'RCSElevationAngles',[-90 90]); struct('ActorID',17,'ClassID',4,'Length',0.24,'Width',0.45,'Height',1.7,'OriginOffset',[0 0 0],'MeshVertices',[0.12 -0.225 1.7;0.12 0.225 1.7;-0.12 0.225 1.7;-0.12 -0.225 1.7;0.12 -0.225 -1.11022302462516e-16;0.12 0.225 -1.11022302462516e-16;-0.12 0.225 -1.11022302462516e-16;-0.12 -0.225 -1.11022302462516e-16],'MeshFaces',[6 2 1;1 5 6;8 4 3;3 7 8;6 7 3;3 2 6;5 1 4;4 8 5;4 1 2;2 3 4;7 6 5;5 8 7],'RCSPattern',[-8 -8;-8 -8],'RCSAzimuthAngles',[-180 180],'RCSElevationAngles',[-90 90]); struct('ActorID',18,'ClassID',4,'Length',0.24,'Width',0.45,'Height',1.7,'OriginOffset',[0 0 0],'MeshVertices',[0.12 -0.225 1.7;0.12 0.225 1.7;-0.12 0.225 1.7;-0.12 -0.225 1.7;0.12 -0.225 -1.11022302462516e-16;0.12 0.225 -1.11022302462516e-16;-0.12 0.225 -1.11022302462516e-16;-0.12 -0.225 -1.11022302462516e-16],'MeshFaces',[6 2 1;1 5 6;8 4 3;3 7 8;6 7 3;3 2 6;5 1 4;4 8 5;4 1 2;2 3 4;7 6 5;5 8 7],'RCSPattern',[-8 -8;-8 -8],'RCSAzimuthAngles',[-180 180],'RCSElevationAngles',[-90 90]); struct('ActorID',19,'ClassID',4,'Length',0.24,'Width',0.45,'Height',1.7,'OriginOffset',[0 0 0],'MeshVertices',[0.12 -0.225 1.7;0.12 0.225 1.7;-0.12 0.225 1.7;-0.12 -0.225 1.7;0.12 -0.225 -1.11022302462516e-16;0.12 0.225 -1.11022302462516e-16;-0.12 0.225 -1.11022302462516e-16;-0.12 -0.225 -1.11022302462516e-16],'MeshFaces',[6 2 1;1 5 6;8 4 3;3 7 8;6 7 3;3 2 6;5 1 4;4 8 5;4 1 2;2 3 4;7 6 5;5 8 7],'RCSPattern',[-8 -8;-8 -8],'RCSAzimuthAngles',[-180 180],'RCSElevationAngles',[-90 90]); struct('ActorID',20,'ClassID',4,'Length',0.24,'Width',0.45,'Height',1.7,'OriginOffset',[0 0 0],'MeshVertices',[0.12 -0.225 1.7;0.12 0.225 1.7;-0.12 0.225 1.7;-0.12 -0.225 1.7;0.12 -0.225 -1.11022302462516e-16;0.12 0.225 -1.11022302462516e-16;-0.12 0.225 -1.11022302462516e-16;-0.12 -0.225 -1.11022302462516e-16],'MeshFaces',[6 2 1;1 5 6;8 4 3;3 7 8;6 7 3;3 2 6;5 1 4;4 8 5;4 1 2;2 3 4;7 6 5;5 8 7],'RCSPattern',[-8 -8;-8 -8],'RCSAzimuthAngles',[-180 180],'RCSElevationAngles',[-90 90]); struct('ActorID',21,'ClassID',4,'Length',0.24,'Width',0.45,'Height',1.7,'OriginOffset',[0 0 0],'MeshVertices',[0.12 -0.225 1.7;0.12 0.225 1.7;-0.12 0.225 1.7;-0.12 -0.225 1.7;0.12 -0.225 -1.11022302462516e-16;0.12 0.225 -1.11022302462516e-16;-0.12 0.225 -1.11022302462516e-16;-0.12 -0.225 -1.11022302462516e-16],'MeshFaces',[6 2 1;1 5 6;8 4 3;3 7 8;6 7 3;3 2 6;5 1 4;4 8 5;4 1 2;2 3 4;7 6 5;5 8 7],'RCSPattern',[-8 -8;-8 -8],'RCSAzimuthAngles',[-180 180],'RCSElevationAngles',[-90 90]); struct('ActorID',22,'ClassID',4,'Length',0.24,'Width',0.45,'Height',1.7,'OriginOffset',[0 0 0],'MeshVertices',[0.12 -0.225 1.7;0.12 0.225 1.7;-0.12 0.225 1.7;-0.12 -0.225 1.7;0.12 -0.225 -1.11022302462516e-16;0.12 0.225 -1.11022302462516e-16;-0.12 0.225 -1.11022302462516e-16;-0.12 -0.225 -1.11022302462516e-16],'MeshFaces',[6 2 1;1 5 6;8 4 3;3 7 8;6 7 3;3 2 6;5 1 4;4 8 5;4 1 2;2 3 4;7 6 5;5 8 7],'RCSPattern',[-8 -8;-8 -8],'RCSAzimuthAngles',[-180 180],'RCSElevationAngles',[-90 90]); struct('ActorID',23,'ClassID',4,'Length',0.24,'Width',0.45,'Height',1.7,'OriginOffset',[0 0 0],'MeshVertices',[0.12 -0.225 1.7;0.12 0.225 1.7;-0.12 0.225 1.7;-0.12 -0.225 1.7;0.12 -0.225 -1.11022302462516e-16;0.12 0.225 -1.11022302462516e-16;-0.12 0.225 -1.11022302462516e-16;-0.12 -0.225 -1.11022302462516e-16],'MeshFaces',[6 2 1;1 5 6;8 4 3;3 7 8;6 7 3;3 2 6;5 1 4;4 8 5;4 1 2;2 3 4;7 6 5;5 8 7],'RCSPattern',[-8 -8;-8 -8],'RCSAzimuthAngles',[-180 180],'RCSElevationAngles',[-90 90]); struct('ActorID',24,'ClassID',4,'Length',0.24,'Width',0.45,'Height',1.7,'OriginOffset',[0 0 0],'MeshVertices',[0.12 -0.225 1.7;0.12 0.225 1.7;-0.12 0.225 1.7;-0.12 -0.225 1.7;0.12 -0.225 -1.11022302462516e-16;0.12 0.225 -1.11022302462516e-16;-0.12 0.225 -1.11022302462516e-16;-0.12 -0.225 -1.11022302462516e-16],'MeshFaces',[6 2 1;1 5 6;8 4 3;3 7 8;6 7 3;3 2 6;5 1 4;4 8 5;4 1 2;2 3 4;7 6 5;5 8 7],'RCSPattern',[-8 -8;-8 -8],'RCSAzimuthAngles',[-180 180],'RCSElevationAngles',[-90 90]); struct('ActorID',25,'ClassID',4,'Length',0.24,'Width',0.45,'Height',1.7,'OriginOffset',[0 0 0],'MeshVertices',[0.12 -0.225 1.7;0.12 0.225 1.7;-0.12 0.225 1.7;-0.12 -0.225 1.7;0.12 -0.225 -1.11022302462516e-16;0.12 0.225 -1.11022302462516e-16;-0.12 0.225 -1.11022302462516e-16;-0.12 -0.225 -1.11022302462516e-16],'MeshFaces',[6 2 1;1 5 6;8 4 3;3 7 8;6 7 3;3 2 6;5 1 4;4 8 5;4 1 2;2 3 4;7 6 5;5 8 7],'RCSPattern',[-8 -8;-8 -8],'RCSAzimuthAngles',[-180 180],'RCSElevationAngles',[-90 90]); struct('ActorID',26,'ClassID',4,'Length',0.24,'Width',0.45,'Height',1.7,'OriginOffset',[0 0 0],'MeshVertices',[0.12 -0.225 1.7;0.12 0.225 1.7;-0.12 0.225 1.7;-0.12 -0.225 1.7;0.12 -0.225 -1.11022302462516e-16;0.12 0.225 -1.11022302462516e-16;-0.12 0.225 -1.11022302462516e-16;-0.12 -0.225 -1.11022302462516e-16],'MeshFaces',[6 2 1;1 5 6;8 4 3;3 7 8;6 7 3;3 2 6;5 1 4;4 8 5;4 1 2;2 3 4;7 6 5;5 8 7],'RCSPattern',[-8 -8;-8 -8],'RCSAzimuthAngles',[-180 180],'RCSElevationAngles',[-90 90]); struct('ActorID',27,'ClassID',4,'Length',0.24,'Width',0.45,'Height',1.7,'OriginOffset',[0 0 0],'MeshVertices',[0.12 -0.225 1.7;0.12 0.225 1.7;-0.12 0.225 1.7;-0.12 -0.225 1.7;0.12 -0.225 -1.11022302462516e-16;0.12 0.225 -1.11022302462516e-16;-0.12 0.225 -1.11022302462516e-16;-0.12 -0.225 -1.11022302462516e-16],'MeshFaces',[6 2 1;1 5 6;8 4 3;3 7 8;6 7 3;3 2 6;5 1 4;4 8 5;4 1 2;2 3 4;7 6 5;5 8 7],'RCSPattern',[-8 -8;-8 -8],'RCSAzimuthAngles',[-180 180],'RCSElevationAngles',[-90 90]); struct('ActorID',28,'ClassID',3,'Length',1.7,'Width',0.45,'Height',1.7,'OriginOffset',[0 0 0],'MeshVertices',[0.85 -0.225 1.7;0.85 0.225 1.7;-0.85 0.225 1.7;-0.85 -0.225 1.7;0.85 -0.225 -1.11022302462516e-16;0.85 0.225 -1.11022302462516e-16;-0.85 0.225 -1.11022302462516e-16;-0.85 -0.225 -1.11022302462516e-16],'MeshFaces',[6 2 1;1 5 6;8 4 3;3 7 8;6 7 3;3 2 6;5 1 4;4 8 5;4 1 2;2 3 4;7 6 5;5 8 7],'RCSPattern',[10 10;10 10],'RCSAzimuthAngles',[-180 180],'RCSElevationAngles',[-90 90]); struct('ActorID',29,'ClassID',4,'Length',0.24,'Width',0.45,'Height',1.7,'OriginOffset',[0 0 0],'MeshVertices',[0.12 -0.225 1.7;0.12 0.225 1.7;-0.12 0.225 1.7;-0.12 -0.225 1.7;0.12 -0.225 -1.11022302462516e-16;0.12 0.225 -1.11022302462516e-16;-0.12 0.225 -1.11022302462516e-16;-0.12 -0.225 -1.11022302462516e-16],'MeshFaces',[6 2 1;1 5 6;8 4 3;3 7 8;6 7 3;3 2 6;5 1 4;4 8 5;4 1 2;2 3 4;7 6 5;5 8 7],'RCSPattern',[-8 -8;-8 -8],'RCSAzimuthAngles',[-180 180],'RCSElevationAngles',[-90 90])]
      settings: SourceProductBaseCode=DR
  Radar2 : drivingscenarioandsensors/Radar Detection Generator  SensorIndex=4  UpdateInterval=0.1  SensorLocation=[0 0]  Height=0.2  Yaw=-180  Pitch=0  Roll=0  BusNameSource=Auto  BusName=BusRadarDetectionGenerator  MaxNumDetectionsSource=Property  MaxNumDetections=50  DetectionCoordinates=Ego Cartesian  SimulateUsing=Interpreted execution  AzimuthResolution=4  ElevationResolution=10  RangeResolution=2.5  RangeRateResolution=0.5  AzimuthBiasFraction=0.1  ElevationBiasFraction=0.1  RangeBiasFraction=0.05  RangeRateBiasFraction=0.05  FieldOfView=[20 5]  MaxRange=10  RangeRateLimits=[-100 100]  DetectionProbability=0.9  FalseAlarmRate=1e-06  ReferenceRange=15  ReferenceRCS=0  HasElevation=on  HasRangeRate=off  HasNoise=on  HasFalseAlarms=on  HasOcclusion=on  InitialSeedSource=Repeatable  InitialSeed=0  UsedSeed=0  ActorProfilesSource=MATLAB expression  ActorProfilesParameters=driving.internal.ActorProfilesRadarParameters  ActorProfilesExpression=[struct('ActorID',1,'ClassID',1,'Length',4.7,'Width',1.8,'Height',1.4,'OriginOffset',[-1.35 0 0],'MeshVertices',[3.7 -0.9 1.4;3.7 0.9 1.4;-1 0.9 1.4;-1 -0.9 1.4;3.7 -0.9 0;3.7 0.9 0;-1 0.9 0;-1 -0.9 0],'MeshFaces',[6 2 1;1 5 6;8 4 3;3 7 8;6 7 3;3 2 6;5 1 4;4 8 5;4 1 2;2 3 4;7 6 5;5 8 7],'RCSPattern',[10 10;10 10],'RCSAzimuthAngles',[-180 180],'RCSElevationAngles',[-90 90]); struct('ActorID',2,'ClassID',1,'Length',4.7,'Width',1.8,'Height',1.4,'OriginOffset',[-1.35 0 0],'MeshVertices',[3.7 -0.9 1.4;3.7 0.9 1.4;-1 0.9 1.4;-1 -0.9 1.4;3.7 -0.9 0;3.7 0.9 0;-1 0.9 0;-1 -0.9 0],'MeshFaces',[6 2 1;1 5 6;8 4 3;3 7 8;6 7 3;3 2 6;5 1 4;4 8 5;4 1 2;2 3 4;7 6 5;5 8 7],'RCSPattern',[10 10;10 10],'RCSAzimuthAngles',[-180 180],'RCSElevationAngles',[-90 90]); struct('ActorID',3,'ClassID',1,'Length',4.7,'Width',1.8,'Height',1.4,'OriginOffset',[-1.35 0 0],'MeshVertices',[3.7 -0.9 1.4;3.7 0.9 1.4;-1 0.9 1.4;-1 -0.9 1.4;3.7 -0.9 0;3.7 0.9 0;-1 0.9 0;-1 -0.9 0],'MeshFaces',[6 2 1;1 5 6;8 4 3;3 7 8;6 7 3;3 2 6;5 1 4;4 8 5;4 1 2;2 3 4;7 6 5;5 8 7],'RCSPattern',[10 10;10 10],'RCSAzimuthAngles',[-180 180],'RCSElevationAngles',[-90 90]); struct('ActorID',4,'ClassID',1,'Length',4.7,'Width',1.8,'Height',1.4,'OriginOffset',[-1.35 0 0],'MeshVertices',[3.7 -0.9 1.4;3.7 0.9 1.4;-1 0.9 1.4;-1 -0.9 1.4;3.7 -0.9 0;3.7 0.9 0;-1 0.9 0;-1 -0.9 0],'MeshFaces',[6 2 1;1 5 6;8 4 3;3 7 8;6 7 3;3 2 6;5 1 4;4 8 5;4 1 2;2 3 4;7 6 5;5 8 7],'RCSPattern',[10 10;10 10],'RCSAzimuthAngles',[-180 180],'RCSElevationAngles',[-90 90]); struct('ActorID',5,'ClassID',1,'Length',4.7,'Width',1.8,'Height',1.4,'OriginOffset',[-1.35 0 0],'MeshVertices',[3.7 -0.9 1.4;3.7 0.9 1.4;-1 0.9 1.4;-1 -0.9 1.4;3.7 -0.9 0;3.7 0.9 0;-1 0.9 0;-1 -0.9 0],'MeshFaces',[6 2 1;1 5 6;8 4 3;3 7 8;6 7 3;3 2 6;5 1 4;4 8 5;4 1 2;2 3 4;7 6 5;5 8 7],'RCSPattern',[10 10;10 10],'RCSAzimuthAngles',[-180 180],'RCSElevationAngles',[-90 90]); struct('ActorID',6,'ClassID',4,'Length',0.24,'Width',0.45,'Height',1.7,'OriginOffset',[0 0 0],'MeshVertices',[0.12 -0.225 1.7;0.12 0.225 1.7;-0.12 0.225 1.7;-0.12 -0.225 1.7;0.12 -0.225 -1.11022302462516e-16;0.12 0.225 -1.11022302462516e-16;-0.12 0.225 -1.11022302462516e-16;-0.12 -0.225 -1.11022302462516e-16],'MeshFaces',[6 2 1;1 5 6;8 4 3;3 7 8;6 7 3;3 2 6;5 1 4;4 8 5;4 1 2;2 3 4;7 6 5;5 8 7],'RCSPattern',[-8 -8;-8 -8],'RCSAzimuthAngles',[-180 180],'RCSElevationAngles',[-90 90]); struct('ActorID',7,'ClassID',4,'Length',0.24,'Width',0.45,'Height',1.7,'OriginOffset',[0 0 0],'MeshVertices',[0.12 -0.225 1.7;0.12 0.225 1.7;-0.12 0.225 1.7;-0.12 -0.225 1.7;0.12 -0.225 -1.11022302462516e-16;0.12 0.225 -1.11022302462516e-16;-0.12 0.225 -1.11022302462516e-16;-0.12 -0.225 -1.11022302462516e-16],'MeshFaces',[6 2 1;1 5 6;8 4 3;3 7 8;6 7 3;3 2 6;5 1 4;4 8 5;4 1 2;2 3 4;7 6 5;5 8 7],'RCSPattern',[-8 -8;-8 -8],'RCSAzimuthAngles',[-180 180],'RCSElevationAngles',[-90 90]); struct('ActorID',8,'ClassID',4,'Length',0.24,'Width',0.45,'Height',1.7,'OriginOffset',[0 0 0],'MeshVertices',[0.12 -0.225 1.7;0.12 0.225 1.7;-0.12 0.225 1.7;-0.12 -0.225 1.7;0.12 -0.225 -1.11022302462516e-16;0.12 0.225 -1.11022302462516e-16;-0.12 0.225 -1.11022302462516e-16;-0.12 -0.225 -1.11022302462516e-16],'MeshFaces',[6 2 1;1 5 6;8 4 3;3 7 8;6 7 3;3 2 6;5 1 4;4 8 5;4 1 2;2 3 4;7 6 5;5 8 7],'RCSPattern',[-8 -8;-8 -8],'RCSAzimuthAngles',[-180 180],'RCSElevationAngles',[-90 90]); struct('ActorID',9,'ClassID',4,'Length',0.24,'Width',0.45,'Height',1.7,'OriginOffset',[0 0 0],'MeshVertices',[0.12 -0.225 1.7;0.12 0.225 1.7;-0.12 0.225 1.7;-0.12 -0.225 1.7;0.12 -0.225 -1.11022302462516e-16;0.12 0.225 -1.11022302462516e-16;-0.12 0.225 -1.11022302462516e-16;-0.12 -0.225 -1.11022302462516e-16],'MeshFaces',[6 2 1;1 5 6;8 4 3;3 7 8;6 7 3;3 2 6;5 1 4;4 8 5;4 1 2;2 3 4;7 6 5;5 8 7],'RCSPattern',[-8 -8;-8 -8],'RCSAzimuthAngles',[-180 180],'RCSElevationAngles',[-90 90]); struct('ActorID',10,'ClassID',4,'Length',0.24,'Width',0.45,'Height',1.7,'OriginOffset',[0 0 0],'MeshVertices',[0.12 -0.225 1.7;0.12 0.225 1.7;-0.12 0.225 1.7;-0.12 -0.225 1.7;0.12 -0.225 -1.11022302462516e-16;0.12 0.225 -1.11022302462516e-16;-0.12 0.225 -1.11022302462516e-16;-0.12 -0.225 -1.11022302462516e-16],'MeshFaces',[6 2 1;1 5 6;8 4 3;3 7 8;6 7 3;3 2 6;5 1 4;4 8 5;4 1 2;2 3 4;7 6 5;5 8 7],'RCSPattern',[-8 -8;-8 -8],'RCSAzimuthAngles',[-180 180],'RCSElevationAngles',[-90 90]); struct('ActorID',11,'ClassID',4,'Length',0.24,'Width',0.45,'Height',1.7,'OriginOffset',[0 0 0],'MeshVertices',[0.12 -0.225 1.7;0.12 0.225 1.7;-0.12 0.225 1.7;-0.12 -0.225 1.7;0.12 -0.225 -1.11022302462516e-16;0.12 0.225 -1.11022302462516e-16;-0.12 0.225 -1.11022302462516e-16;-0.12 -0.225 -1.11022302462516e-16],'MeshFaces',[6 2 1;1 5 6;8 4 3;3 7 8;6 7 3;3 2 6;5 1 4;4 8 5;4 1 2;2 3 4;7 6 5;5 8 7],'RCSPattern',[-8 -8;-8 -8],'RCSAzimuthAngles',[-180 180],'RCSElevationAngles',[-90 90]); struct('ActorID',12,'ClassID',4,'Length',0.24,'Width',0.45,'Height',1.7,'OriginOffset',[0 0 0],'MeshVertices',[0.12 -0.225 1.7;0.12 0.225 1.7;-0.12 0.225 1.7;-0.12 -0.225 1.7;0.12 -0.225 -1.11022302462516e-16;0.12 0.225 -1.11022302462516e-16;-0.12 0.225 -1.11022302462516e-16;-0.12 -0.225 -1.11022302462516e-16],'MeshFaces',[6 2 1;1 5 6;8 4 3;3 7 8;6 7 3;3 2 6;5 1 4;4 8 5;4 1 2;2 3 4;7 6 5;5 8 7],'RCSPattern',[-8 -8;-8 -8],'RCSAzimuthAngles',[-180 180],'RCSElevationAngles',[-90 90]); struct('ActorID',13,'ClassID',4,'Length',0.24,'Width',0.45,'Height',1.7,'OriginOffset',[0 0 0],'MeshVertices',[0.12 -0.225 1.7;0.12 0.225 1.7;-0.12 0.225 1.7;-0.12 -0.225 1.7;0.12 -0.225 -1.11022302462516e-16;0.12 0.225 -1.11022302462516e-16;-0.12 0.225 -1.11022302462516e-16;-0.12 -0.225 -1.11022302462516e-16],'MeshFaces',[6 2 1;1 5 6;8 4 3;3 7 8;6 7 3;3 2 6;5 1 4;4 8 5;4 1 2;2 3 4;7 6 5;5 8 7],'RCSPattern',[-8 -8;-8 -8],'RCSAzimuthAngles',[-180 180],'RCSElevationAngles',[-90 90]); struct('ActorID',14,'ClassID',4,'Length',0.24,'Width',0.45,'Height',1.7,'OriginOffset',[0 0 0],'MeshVertices',[0.12 -0.225 1.7;0.12 0.225 1.7;-0.12 0.225 1.7;-0.12 -0.225 1.7;0.12 -0.225 -1.11022302462516e-16;0.12 0.225 -1.11022302462516e-16;-0.12 0.225 -1.11022302462516e-16;-0.12 -0.225 -1.11022302462516e-16],'MeshFaces',[6 2 1;1 5 6;8 4 3;3 7 8;6 7 3;3 2 6;5 1 4;4 8 5;4 1 2;2 3 4;7 6 5;5 8 7],'RCSPattern',[-8 -8;-8 -8],'RCSAzimuthAngles',[-180 180],'RCSElevationAngles',[-90 90]); struct('ActorID',15,'ClassID',4,'Length',0.24,'Width',0.45,'Height',1.7,'OriginOffset',[0 0 0],'MeshVertices',[0.12 -0.225 1.7;0.12 0.225 1.7;-0.12 0.225 1.7;-0.12 -0.225 1.7;0.12 -0.225 -1.11022302462516e-16;0.12 0.225 -1.11022302462516e-16;-0.12 0.225 -1.11022302462516e-16;-0.12 -0.225 -1.11022302462516e-16],'MeshFaces',[6 2 1;1 5 6;8 4 3;3 7 8;6 7 3;3 2 6;5 1 4;4 8 5;4 1 2;2 3 4;7 6 5;5 8 7],'RCSPattern',[-8 -8;-8 -8],'RCSAzimuthAngles',[-180 180],'RCSElevationAngles',[-90 90]); struct('ActorID',16,'ClassID',4,'Length',0.24,'Width',0.45,'Height',1.7,'OriginOffset',[0 0 0],'MeshVertices',[0.12 -0.225 1.7;0.12 0.225 1.7;-0.12 0.225 1.7;-0.12 -0.225 1.7;0.12 -0.225 -1.11022302462516e-16;0.12 0.225 -1.11022302462516e-16;-0.12 0.225 -1.11022302462516e-16;-0.12 -0.225 -1.11022302462516e-16],'MeshFaces',[6 2 1;1 5 6;8 4 3;3 7 8;6 7 3;3 2 6;5 1 4;4 8 5;4 1 2;2 3 4;7 6 5;5 8 7],'RCSPattern',[-8 -8;-8 -8],'RCSAzimuthAngles',[-180 180],'RCSElevationAngles',[-90 90]); struct('ActorID',17,'ClassID',4,'Length',0.24,'Width',0.45,'Height',1.7,'OriginOffset',[0 0 0],'MeshVertices',[0.12 -0.225 1.7;0.12 0.225 1.7;-0.12 0.225 1.7;-0.12 -0.225 1.7;0.12 -0.225 -1.11022302462516e-16;0.12 0.225 -1.11022302462516e-16;-0.12 0.225 -1.11022302462516e-16;-0.12 -0.225 -1.11022302462516e-16],'MeshFaces',[6 2 1;1 5 6;8 4 3;3 7 8;6 7 3;3 2 6;5 1 4;4 8 5;4 1 2;2 3 4;7 6 5;5 8 7],'RCSPattern',[-8 -8;-8 -8],'RCSAzimuthAngles',[-180 180],'RCSElevationAngles',[-90 90]); struct('ActorID',18,'ClassID',4,'Length',0.24,'Width',0.45,'Height',1.7,'OriginOffset',[0 0 0],'MeshVertices',[0.12 -0.225 1.7;0.12 0.225 1.7;-0.12 0.225 1.7;-0.12 -0.225 1.7;0.12 -0.225 -1.11022302462516e-16;0.12 0.225 -1.11022302462516e-16;-0.12 0.225 -1.11022302462516e-16;-0.12 -0.225 -1.11022302462516e-16],'MeshFaces',[6 2 1;1 5 6;8 4 3;3 7 8;6 7 3;3 2 6;5 1 4;4 8 5;4 1 2;2 3 4;7 6 5;5 8 7],'RCSPattern',[-8 -8;-8 -8],'RCSAzimuthAngles',[-180 180],'RCSElevationAngles',[-90 90]); struct('ActorID',19,'ClassID',4,'Length',0.24,'Width',0.45,'Height',1.7,'OriginOffset',[0 0 0],'MeshVertices',[0.12 -0.225 1.7;0.12 0.225 1.7;-0.12 0.225 1.7;-0.12 -0.225 1.7;0.12 -0.225 -1.11022302462516e-16;0.12 0.225 -1.11022302462516e-16;-0.12 0.225 -1.11022302462516e-16;-0.12 -0.225 -1.11022302462516e-16],'MeshFaces',[6 2 1;1 5 6;8 4 3;3 7 8;6 7 3;3 2 6;5 1 4;4 8 5;4 1 2;2 3 4;7 6 5;5 8 7],'RCSPattern',[-8 -8;-8 -8],'RCSAzimuthAngles',[-180 180],'RCSElevationAngles',[-90 90]); struct('ActorID',20,'ClassID',4,'Length',0.24,'Width',0.45,'Height',1.7,'OriginOffset',[0 0 0],'MeshVertices',[0.12 -0.225 1.7;0.12 0.225 1.7;-0.12 0.225 1.7;-0.12 -0.225 1.7;0.12 -0.225 -1.11022302462516e-16;0.12 0.225 -1.11022302462516e-16;-0.12 0.225 -1.11022302462516e-16;-0.12 -0.225 -1.11022302462516e-16],'MeshFaces',[6 2 1;1 5 6;8 4 3;3 7 8;6 7 3;3 2 6;5 1 4;4 8 5;4 1 2;2 3 4;7 6 5;5 8 7],'RCSPattern',[-8 -8;-8 -8],'RCSAzimuthAngles',[-180 180],'RCSElevationAngles',[-90 90]); struct('ActorID',21,'ClassID',4,'Length',0.24,'Width',0.45,'Height',1.7,'OriginOffset',[0 0 0],'MeshVertices',[0.12 -0.225 1.7;0.12 0.225 1.7;-0.12 0.225 1.7;-0.12 -0.225 1.7;0.12 -0.225 -1.11022302462516e-16;0.12 0.225 -1.11022302462516e-16;-0.12 0.225 -1.11022302462516e-16;-0.12 -0.225 -1.11022302462516e-16],'MeshFaces',[6 2 1;1 5 6;8 4 3;3 7 8;6 7 3;3 2 6;5 1 4;4 8 5;4 1 2;2 3 4;7 6 5;5 8 7],'RCSPattern',[-8 -8;-8 -8],'RCSAzimuthAngles',[-180 180],'RCSElevationAngles',[-90 90]); struct('ActorID',22,'ClassID',4,'Length',0.24,'Width',0.45,'Height',1.7,'OriginOffset',[0 0 0],'MeshVertices',[0.12 -0.225 1.7;0.12 0.225 1.7;-0.12 0.225 1.7;-0.12 -0.225 1.7;0.12 -0.225 -1.11022302462516e-16;0.12 0.225 -1.11022302462516e-16;-0.12 0.225 -1.11022302462516e-16;-0.12 -0.225 -1.11022302462516e-16],'MeshFaces',[6 2 1;1 5 6;8 4 3;3 7 8;6 7 3;3 2 6;5 1 4;4 8 5;4 1 2;2 3 4;7 6 5;5 8 7],'RCSPattern',[-8 -8;-8 -8],'RCSAzimuthAngles',[-180 180],'RCSElevationAngles',[-90 90]); struct('ActorID',23,'ClassID',4,'Length',0.24,'Width',0.45,'Height',1.7,'OriginOffset',[0 0 0],'MeshVertices',[0.12 -0.225 1.7;0.12 0.225 1.7;-0.12 0.225 1.7;-0.12 -0.225 1.7;0.12 -0.225 -1.11022302462516e-16;0.12 0.225 -1.11022302462516e-16;-0.12 0.225 -1.11022302462516e-16;-0.12 -0.225 -1.11022302462516e-16],'MeshFaces',[6 2 1;1 5 6;8 4 3;3 7 8;6 7 3;3 2 6;5 1 4;4 8 5;4 1 2;2 3 4;7 6 5;5 8 7],'RCSPattern',[-8 -8;-8 -8],'RCSAzimuthAngles',[-180 180],'RCSElevationAngles',[-90 90]); struct('ActorID',24,'ClassID',4,'Length',0.24,'Width',0.45,'Height',1.7,'OriginOffset',[0 0 0],'MeshVertices',[0.12 -0.225 1.7;0.12 0.225 1.7;-0.12 0.225 1.7;-0.12 -0.225 1.7;0.12 -0.225 -1.11022302462516e-16;0.12 0.225 -1.11022302462516e-16;-0.12 0.225 -1.11022302462516e-16;-0.12 -0.225 -1.11022302462516e-16],'MeshFaces',[6 2 1;1 5 6;8 4 3;3 7 8;6 7 3;3 2 6;5 1 4;4 8 5;4 1 2;2 3 4;7 6 5;5 8 7],'RCSPattern',[-8 -8;-8 -8],'RCSAzimuthAngles',[-180 180],'RCSElevationAngles',[-90 90]); struct('ActorID',25,'ClassID',4,'Length',0.24,'Width',0.45,'Height',1.7,'OriginOffset',[0 0 0],'MeshVertices',[0.12 -0.225 1.7;0.12 0.225 1.7;-0.12 0.225 1.7;-0.12 -0.225 1.7;0.12 -0.225 -1.11022302462516e-16;0.12 0.225 -1.11022302462516e-16;-0.12 0.225 -1.11022302462516e-16;-0.12 -0.225 -1.11022302462516e-16],'MeshFaces',[6 2 1;1 5 6;8 4 3;3 7 8;6 7 3;3 2 6;5 1 4;4 8 5;4 1 2;2 3 4;7 6 5;5 8 7],'RCSPattern',[-8 -8;-8 -8],'RCSAzimuthAngles',[-180 180],'RCSElevationAngles',[-90 90]); struct('ActorID',26,'ClassID',4,'Length',0.24,'Width',0.45,'Height',1.7,'OriginOffset',[0 0 0],'MeshVertices',[0.12 -0.225 1.7;0.12 0.225 1.7;-0.12 0.225 1.7;-0.12 -0.225 1.7;0.12 -0.225 -1.11022302462516e-16;0.12 0.225 -1.11022302462516e-16;-0.12 0.225 -1.11022302462516e-16;-0.12 -0.225 -1.11022302462516e-16],'MeshFaces',[6 2 1;1 5 6;8 4 3;3 7 8;6 7 3;3 2 6;5 1 4;4 8 5;4 1 2;2 3 4;7 6 5;5 8 7],'RCSPattern',[-8 -8;-8 -8],'RCSAzimuthAngles',[-180 180],'RCSElevationAngles',[-90 90]); struct('ActorID',27,'ClassID',4,'Length',0.24,'Width',0.45,'Height',1.7,'OriginOffset',[0 0 0],'MeshVertices',[0.12 -0.225 1.7;0.12 0.225 1.7;-0.12 0.225 1.7;-0.12 -0.225 1.7;0.12 -0.225 -1.11022302462516e-16;0.12 0.225 -1.11022302462516e-16;-0.12 0.225 -1.11022302462516e-16;-0.12 -0.225 -1.11022302462516e-16],'MeshFaces',[6 2 1;1 5 6;8 4 3;3 7 8;6 7 3;3 2 6;5 1 4;4 8 5;4 1 2;2 3 4;7 6 5;5 8 7],'RCSPattern',[-8 -8;-8 -8],'RCSAzimuthAngles',[-180 180],'RCSElevationAngles',[-90 90]); struct('ActorID',28,'ClassID',3,'Length',1.7,'Width',0.45,'Height',1.7,'OriginOffset',[0 0 0],'MeshVertices',[0.85 -0.225 1.7;0.85 0.225 1.7;-0.85 0.225 1.7;-0.85 -0.225 1.7;0.85 -0.225 -1.11022302462516e-16;0.85 0.225 -1.11022302462516e-16;-0.85 0.225 -1.11022302462516e-16;-0.85 -0.225 -1.11022302462516e-16],'MeshFaces',[6 2 1;1 5 6;8 4 3;3 7 8;6 7 3;3 2 6;5 1 4;4 8 5;4 1 2;2 3 4;7 6 5;5 8 7],'RCSPattern',[10 10;10 10],'RCSAzimuthAngles',[-180 180],'RCSElevationAngles',[-90 90]); struct('ActorID',29,'ClassID',4,'Length',0.24,'Width',0.45,'Height',1.7,'OriginOffset',[0 0 0],'MeshVertices',[0.12 -0.225 1.7;0.12 0.225 1.7;-0.12 0.225 1.7;-0.12 -0.225 1.7;0.12 -0.225 -1.11022302462516e-16;0.12 0.225 -1.11022302462516e-16;-0.12 0.225 -1.11022302462516e-16;-0.12 -0.225 -1.11022302462516e-16],'MeshFaces',[6 2 1;1 5 6;8 4 3;3 7 8;6 7 3;3 2 6;5 1 4;4 8 5;4 1 2;2 3 4;7 6 5;5 8 7],'RCSPattern',[-8 -8;-8 -8],'RCSAzimuthAngles',[-180 180],'RCSElevationAngles',[-90 90])]
      settings: SourceProductBaseCode=DR
